simulink model "SIM_EXO_DAL_MN"  (R2021b)
(part 15 of 24)

t6933 = ct{2277};
t6934 = ct{2278};
t6994 = ct{2279};
t7 = ct{2280};
t7000 = ct{2281};
t7010 = ct{2282};
t7011 = ct{2283};
t7012 = ct{2284};
t7015 = ct{2285};
t7019 = ct{2286};
t7020 = ct{2287};
t7026 = ct{2288};
t7027 = ct{2289};
t7031 = ct{2290};
t7032 = ct{2291};
t7033 = ct{2292};
t7034 = ct{2293};
t7035 = ct{2294};
t7039 = ct{2295};
t7040 = ct{2296};
t7042 = ct{2297};
t7043 = ct{2298};
t7044 = ct{2299};
t7045 = ct{2300};
t7046 = ct{2301};
t7047 = ct{2302};
t7052 = ct{2303};
t7055 = ct{2304};
t7060 = ct{2305};
t7061 = ct{2306};
t7062 = ct{2307};
t7064 = ct{2308};
t7065 = ct{2309};
t7071 = ct{2310};
t7079 = ct{2311};
t7080 = ct{2312};
t7082 = ct{2313};
t7083 = ct{2314};
t7085 = ct{2315};
t7086 = ct{2316};
t7087 = ct{2317};
t7088 = ct{2318};
t7089 = ct{2319};
t7091 = ct{2320};
t7093 = ct{2321};
t7095 = ct{2322};
t7096 = ct{2323};
t7098 = ct{2324};
t71 = ct{2325};
t7100 = ct{2326};
t7104 = ct{2327};
t7108 = ct{2328};
t7109 = ct{2329};
t7110 = ct{2330};
t7113 = ct{2331};
t7115 = ct{2332};
t7119 = ct{2333};
t712 = ct{2334};
t7140 = ct{2335};
t7141 = ct{2336};
t7148 = ct{2337};
t7149 = ct{2338};
t7153 = ct{2339};
t7159 = ct{2340};
t7199 = ct{2341};
t72 = ct{2342};
t724 = ct{2343};
t7244 = ct{2344};
t7248 = ct{2345};
t7256 = ct{2346};
t7258 = ct{2347};
t7297 = ct{2348};
t73 = ct{2349};
t7306 = ct{2350};
t7334 = ct{2351};
t7335 = ct{2352};
t7364 = ct{2353};
t738 = ct{2354};
t739 = ct{2355};
t741 = ct{2356};
t742 = ct{2357};
t75 = ct{2358};
t7528 = ct{2359};
t753 = ct{2360};
t7549 = ct{2361};
t7550 = ct{2362};
t7551 = ct{2363};
t7553 = ct{2364};
t7557 = ct{2365};
t7558 = ct{2366};
t7560 = ct{2367};
t7564 = ct{2368};
t7565 = ct{2369};
t7567 = ct{2370};
t7568 = ct{2371};
t7569 = ct{2372};
t7570 = ct{2373};
t7571 = ct{2374};
t7573 = ct{2375};
t7574 = ct{2376};
t7575 = ct{2377};
t7576 = ct{2378};
t7577 = ct{2379};
t7578 = ct{2380};
t7579 = ct{2381};
t7580 = ct{2382};
t7581 = ct{2383};
t76 = ct{2384};
t760 = ct{2385};
t781 = ct{2386};
t792 = ct{2387};
t796 = ct{2388};
t797 = ct{2389};
t8 = ct{2390};
t803 = ct{2391};
t81 = ct{2392};
t824 = ct{2393};
t825 = ct{2394};
t826 = ct{2395};
t827 = ct{2396};
t830 = ct{2397};
t832 = ct{2398};
t84 = ct{2399};
t845 = ct{2400};
t847 = ct{2401};
t848 = ct{2402};
t852 = ct{2403};
t856 = ct{2404};
t86 = ct{2405};
t861 = ct{2406};
t866 = ct{2407};
t868 = ct{2408};
t869 = ct{2409};
t874 = ct{2410};
t875 = ct{2411};
t877 = ct{2412};
t878 = ct{2413};
t881 = ct{2414};
t893 = ct{2415};
t899 = ct{2416};
t9 = ct{2417};
t90 = ct{2418};
t902 = ct{2419};
t903 = ct{2420};
t905 = ct{2421};
t908 = ct{2422};
t909 = ct{2423};
t91 = ct{2424};
t910 = ct{2425};
t911 = ct{2426};
t912 = ct{2427};
t915 = ct{2428};
t917 = ct{2429};
t919 = ct{2430};
t922 = ct{2431};
t925 = ct{2432};
t926 = ct{2433};
t928 = ct{2434};
t929 = ct{2435};
t930 = ct{2436};
t931 = ct{2437};
t932 = ct{2438};
t934 = ct{2439};
t940 = ct{2440};
t944 = ct{2441};
t945 = ct{2442};
t947 = ct{2443};
t95 = ct{2444};
t952 = ct{2445};
t954 = ct{2446};
t955 = ct{2447};
t957 = ct{2448};
t958 = ct{2449};
t968 = ct{2450};
t970 = ct{2451};
t971 = ct{2452};
t972 = ct{2453};
t975 = ct{2454};
t976 = ct{2455};
t984 = ct{2456};
t985 = ct{2457};
t986 = ct{2458};
t989 = ct{2459};
t99 = ct{2460};
t991 = ct{2461};
t998 = ct{2462};
t6510 = t5822.*t6230.*(t29-t30).*(-5.517689141340903e-72);
t6527 = t5824.*t6222.*(t29-t30).*(-1.015171749786156e-71);
t6528 = t5824.*t6222.*(t29-t30).*(-5.520609140571798e-70);
t6529 = t5824.*t6222.*(t29-t30).*(-5.517689141340903e-72);
t6530 = t5824.*t6222.*(t29-t30).*1.015171749786156e-71;
t6531 = t5824.*t6222.*(t29-t30).*5.520609140571798e-70;
t6532 = t5824.*t6230.*(t29-t30).*(-1.015171749786156e-71);
t6533 = t5824.*t6230.*(t29-t30).*(-5.520609140571798e-70);
t6534 = t5824.*t6230.*(t29-t30).*(-5.517689141340903e-72);
t6535 = t5824.*t6230.*(t29-t30).*1.015171749786156e-71;
t6536 = t5824.*t6230.*(t29-t30).*5.520609140571798e-70;
t6550 = t5.*t5824.*t6230.*(t29-t30).*(-1.065477564130357e-78);
t6551 = t9.*t5824.*t6230.*(t29-t30).*(-1.065477564130357e-78);
t6552 = t9.*t5824.*t6230.*(t29-t30).*1.065477564130357e-78;
t6573 = t5824.*(t5879-t5.*(t7.*(t3719-t3788)+(t3.*t34.*t191.*(t29-t30))./8.112963841460668e+31)).*(t29-t30).*(-7.596454196607839e-68);
t6574 = (t5824.*(t5878+t9.*(t7.*(t3719-t3788)+(t3.*t34.*t191.*(t29-t30))./8.112963841460668e+31)).*(t29-t30))./1.316403645856965e+67;
t6580 = (t5779.*t6422)./2.0;
t6582 = t5824.*(t5879-t5.*(t7.*(t3719-t3788)+(t3.*t34.*t191.*(t29-t30))./8.112963841460668e+31)).*(t29-t30).*(-1.015171749786156e-71);
t6583 = t5824.*(t5879-t5.*(t7.*(t3719-t3788)+(t3.*t34.*t191.*(t29-t30))./8.112963841460668e+31)).*(t29-t30).*(-5.520609140571798e-70);
t6585 = t5824.*(t5878+t9.*(t7.*(t3719-t3788)+(t3.*t34.*t191.*(t29-t30))./8.112963841460668e+31)).*(t29-t30).*5.520609140571798e-70;
t6586 = t5824.*(t5878+t9.*(t7.*(t3719-t3788)+(t3.*t34.*t191.*(t29-t30))./8.112963841460668e+31)).*(t29-t30).*5.517689141340903e-72;
t6590 = t5824.*(t5879-t5.*(t7.*(t3719-t3788)+(t3.*t34.*t191.*(t29-t30))./8.112963841460668e+31)).*(t29-t30).*(-1.065477564130357e-78);
t6591 = t5824.*(t5878+t9.*(t7.*(t3719-t3788)+(t3.*t34.*t191.*(t29-t30))./8.112963841460668e+31)).*(t29-t30).*1.065477564130357e-78;
t6598 = t6103.*t6230.*2.0;
t6603 = t6103.*t6230.*2.67275158517898e-4;
t6604 = t6103.*t6230.*1.45270122047331e-4;
t6605 = t6103.*t6230.*8.40184101230148e-6;
t6607 = t6103.*t6230.*6.293113355513489e-13;
t6608 = t6103.*t6230.*8.252610559395431e-13;
t6634 = t6222.*t6230.*2.0;
t6638 = (t91.*t5824.*t6418)./1.316403645856965e+67;
t6649 = t6222.*t6230.*2.67275158517898e-4;
t6651 = t6222.*t6230.*1.45270122047331e-4;
t6653 = t6222.*t6230.*8.40184101230148e-6;
t6655 = t6222.*t6230.*6.293113355513489e-13;
t6657 = t6222.*t6230.*8.252610559395431e-13;
t6658 = t91.*t5824.*t6418.*5.520609140571798e-70;
t6659 = t91.*t5824.*t6418.*5.517689141340903e-72;
t6664 = t91.*t5824.*t6418.*1.065477564130357e-78;
t6696 = t6230.*(t5879-t5.*(t7.*(t3719-t3788)+(t3.*t34.*t191.*(t29-t30))./8.112963841460668e+31));
t6698 = -t6230.*(t5878+t9.*(t7.*(t3719-t3788)+(t3.*t34.*t191.*(t29-t30))./8.112963841460668e+31));
t6699 = t1498+t2507+t2772+t4837+t5024+t5145+t5301+t5638+t5639;
t6748 = t6230.*(t5878+t9.*(t7.*(t3719-t3788)+(t3.*t34.*t191.*(t29-t30))./8.112963841460668e+31)).*(-7.26350610236655e-5);
t6751 = t6230.*(t5878+t9.*(t7.*(t3719-t3788)+(t3.*t34.*t191.*(t29-t30))./8.112963841460668e+31)).*(-1.744166498897461e-6);
t6752 = t6230.*(t5878+t9.*(t7.*(t3719-t3788)+(t3.*t34.*t191.*(t29-t30))./8.112963841460668e+31)).*(-1.246862701090643e-6);
t6753 = t6230.*(t5878+t9.*(t7.*(t3719-t3788)+(t3.*t34.*t191.*(t29-t30))./8.112963841460668e+31)).*(-2.179051830709965e-7);
t6764 = t6230.*(t5878+t9.*(t7.*(t3719-t3788)+(t3.*t34.*t191.*(t29-t30))./8.112963841460668e+31)).*(-1.40259855e-11);
t6765 = t6230.*(t5878+t9.*(t7.*(t3719-t3788)+(t3.*t34.*t191.*(t29-t30))./8.112963841460668e+31)).*(-4.126305279697715e-13);
t6795 = t824+t1636+t1779+t3309+t3371+t3421+t3835+t3838+t4427+t5235+t5752;
t6828 = t6230.*(t6105-t9.*((t197.*(t29-t30))./9.007199254740992e+15+t3.*(t3219-t3230)));
t6829 = -t6230.*(t6106+t5.*((t197.*(t29-t30))./9.007199254740992e+15+t3.*(t3219-t3230)));
t6831 = t6230.*(t6106+t5.*((t197.*(t29-t30))./9.007199254740992e+15+t3.*(t3219-t3230)));
t6926 = t1488+t1567+t1628+t2570+t2805+t2889+t4927+t5017+t5093+t5144+t5423+t5650;
et8 = t5888+t5795.*(t2088-t4743).*8.081970098144003e-70;
et9 = t5683.*(t197.*(t29-t30).*9.007199254740992e+15+t3.*(t2444-t2449)).*8.081970098144003e-70;
t7013 = t4119.*(et8+et9).*(-1.0./2.0);
t7014 = t5771+t6353+t6354;
t7016 = -t7015;
et10 = t5889+t5795.*(t2088-t4743).*5.344156668414146e-72;
et11 = t5683.*(t197.*(t29-t30).*9.007199254740992e+15+t3.*(t2444-t2449)).*5.344156668414146e-72;
t7017 = t5658.*(et10+et11).*(-1.0./2.0);
et12 = t5892+t5795.*(t2088-t4743).*7.671525497590686e-73;
et13 = t5683.*(t197.*(t29-t30).*9.007199254740992e+15+t3.*(t2444-t2449)).*7.671525497590686e-73;
t7018 = t5662.*(et12+et13).*(-1.0./2.0);
et14 = t5883+t5795.*(t2088-t4743).*4.121912899099809e-68;
et15 = t5683.*(t197.*(t29-t30).*9.007199254740992e+15+t3.*(t2444-t2449)).*4.121912899099809e-68;
t7028 = t5939.*(et14+et15).*(-1.0./2.0);
et16 = t5882+t5795.*(t2088-t4743).*1.879526485671887e-68;
et17 = t5683.*(t197.*(t29-t30).*9.007199254740992e+15+t3.*(t2444-t2449)).*1.879526485671887e-68;
t7029 = t5940.*(et16+et17).*(-1.0./2.0);
t7030 = (t6422.*t6609)./2.0;
t7036 = -t7034;
t7041 = -t7039;
t7048 = -t7047;
t7051 = (t1429.*t7042)./2.0;
t7054 = (t1427.*t7045)./2.0;
t7056 = -t7055;
t7057 = (t6422.*t6874)./2.0;
t7067 = t1499+t1763+t2284+t2296+t2523+t2740+t2752+t3080+t3166+t4846+t5056+t5314+t5340+t5378+t5391+t5405+t5416+t5644+t5646;
t7069 = t1524+t1946+t2239+t2328+t2548+t2783+t2807+t3096+t3168+t4925+t5189+t5335+t5337+t5392+t5395+t5409+t5431+t5642+t5645;
t7078 = t1536+t1585+t1593+t1700+t1704+t2553+t2577+t2744+t2801+t2815+t2933+t4974+t5031+t5113+t5139+t5202+t5252+t5307+t5412+t5447+t5652+t5655;
t7084 = -t7083;
t7090 = -t7089;
t7092 = -t7091;
t7094 = -t7093;
t7097 = -t7096;
t7101 = -t7100;
t7111 = -t7110;
t7162 = t1533+t1663+t1760+t1809+t2358+t2362+t2435+t2452+t3565+t3572+t3617+t3640+t4047+t4050+t4069+t4083+t4186+t4211+t4683+t4714+t7042;
t7163 = t1683+t1807+t2036+t2081+t2359+t2364+t2439+t2454+t3676+t3717+t3781+t3818+t4053+t4056+t4070+t4086+t4256+t4333+t4684+t4717+t7045;
t7172 = t1605+t1849+t1896+t1961+t2079+t2100+t2176+t2208+t3648+t3752+t3754+t3833+t3892+t3904+t3915+t3940+t4315+t4368+t4371+t4460+t7062;
t5767 = -t5761;
t5785 = t5685./6.582018229284824e+63;
t5801 = t5685.*2.060956449549905e-68;
t5803 = t5685.*9.397632428359433e-69;
t5804 = t5685.*4.040985049072001e-70;
t5806 = t5685.*2.672078334207073e-72;
t5807 = t5685.*3.835762748795343e-73;
t5921 = (t1460.*t5840)./2.0;
t5924 = -t5922;
t5950 = (t3444.*t5840)./2.0;
t5987 = -t5985;
t5989 = -t5986;
t5993 = -t5992;
t6025 = -t6021;
t6040 = -t6033;
t6041 = -t6034;
t6044 = -t6037;
t6063 = -t6059;
t6080 = -t6074;
t6116 = t5657.*t5840;
t6141 = t6114.*7.26350610236655e-5;
t6144 = t6114.*1.744166498897461e-6;
t6146 = t6114.*1.246862701090643e-6;
t6147 = -t6142;
t6150 = -t6145;
t6155 = t6114.*2.179051830709965e-7;
t6172 = -t6170;
t6173 = t6114.*1.40259855e-11;
t6176 = -t6171;
t6177 = t6114.*4.126305279697715e-13;
t6216 = t5694+t5864;
t6217 = t5.*t6213;
t6218 = t9.*t6213;
t6219 = t5784.*t5840;
t6246 = -t6234;
t6252 = t5.*t6239;
t6253 = t9.*t6239;
t6256 = -t6254;
t6273 = t6214.*7.26735e-3;
t6275 = t6214.*7.26350610236655e-5;
t6290 = t6239.*1.33637579258949e-4;
t6294 = t6214.*1.40259855e-11;
t6296 = t6239.*7.26350610236655e-5;
t6297 = t47.*t6239;
t6300 = t6239.*4.20092050615074e-6;
t6304 = t58.*t6239;
t6305 = t75.*t6239;
t6306 = t76.*t6239;
t6307 = t84.*t6239;
t6310 = t71.*t6239;
t6321 = t6239.*3.146556677756745e-13;
t6323 = t6239.*4.126305279697715e-13;
t6324 = t142.*t6239;
t6327 = t151.*t6239;
t6334 = -t6332;
t6335 = -t6333;
t6339 = -t6336;
t6346 = -t6345;
t6358 = t5870+t5880;
t6370 = -t6368;
t6371 = -t6369;
t6394 = -t6392;
t6468 = t5874+t6233;
t6480 = (t91.*t5824.*t6213)./1.316403645856965e+67;
t6485 = -t6483;
t6498 = -t6496;
t6499 = t5.*t6497;
t6500 = t9.*t6497;
t6511 = t91.*t5824.*t6213.*1.015171749786156e-71;
t6512 = t91.*t5824.*t6213.*5.520609140571798e-70;
t6513 = t91.*t5824.*t6213.*5.517689141340903e-72;
t6537 = t9.*t6532;
t6538 = t5.*t6533;
t6539 = t9.*t6533;
t6540 = t9.*t6535;
t6541 = t9.*t6536;
t6542 = t5.*t6534;
t6570 = (t91.*t5824.*t6355)./1.316403645856965e+67;
t6571 = (t91.*t5824.*t6356)./1.316403645856965e+67;
t6575 = -t6574;
t6576 = t91.*t5824.*t6355.*1.015171749786156e-71;
t6577 = t91.*t5824.*t6355.*5.520609140571798e-70;
t6578 = t91.*t5824.*t6356.*5.520609140571798e-70;
t6579 = t91.*t5824.*t6356.*5.517689141340903e-72;
t6584 = t91.*t5824.*t6355.*1.065477564130357e-78;
t6587 = -t6585;
t6588 = t91.*t5824.*t6356.*1.065477564130357e-78;
t6592 = -t6591;
t6639 = (t91.*t5824.*t6419)./1.316403645856965e+67;
t6652 = -t6651;
t6654 = -t6653;
t6656 = -t6655;
t6660 = t91.*t5824.*t6419.*1.015171749786156e-71;
t6661 = t91.*t5824.*t6419.*5.520609140571798e-70;
t6667 = -t6664;
t6668 = t91.*t5824.*t6419.*1.065477564130357e-78;
t6688 = t5809+t6018+t6019;
t6737 = t6696.*1.33637579258949e-4;
t6743 = t6696.*4.00912737776847e-7;
t6744 = t6696.*1.246862701090643e-6;
t6745 = t6696.*3.383302988283333e-6;
t6756 = t6696.*3.146556677756745e-13;
t6757 = t6696.*1.40259855e-11;
t6810 = t5830+t6082+t6090;
t6813 = t5829+t6084+t6091;
t6816 = t5833+t6087+t6095;
t6819 = t5834+t6088+t6096;
t6820 = t5836+t6089+t6097;
t6830 = -t6828;
t6833 = t5843+t6117+t6122;
t6852 = t6828.*7.26350610236655e-5;
t6853 = t6831.*(-1.33637579258949e-4);
t6854 = t6828.*1.744166498897461e-6;
t6856 = t6828.*1.246862701090643e-6;
t6857 = t6831.*1.33637579258949e-4;
t6859 = t6828.*2.179051830709965e-7;
t6860 = t6831.*(-4.00912737776847e-7);
t6861 = t6831.*(-1.246862701090643e-6);
t6862 = t6831.*(-3.383302988283333e-6);
t6863 = t6831.*1.246862701090643e-6;
t6864 = t6828.*1.40259855e-11;
t6865 = t6828.*4.126305279697715e-13;
t6867 = t6831.*(-3.146556677756745e-13);
t6870 = t6831.*(-1.40259855e-11);
t6879 = t4119.*(t5831-t6095+t5679.*(t2088-t4743).*8.081970098144003e-70).*(-1.0./2.0);
t6880 = (t4119.*(t5831-t6095+t5679.*(t2088-t4743).*8.081970098144003e-70))./2.0;
t6886 = t5885+t6139+t6166;
t6887 = t5884+t6140+t6168;
t6899 = t5890+t6149+t6174;
t6905 = t5891+t6156+t6178;
t6912 = t5893+t6163+t6184;
t6927 = t1511+t1586+t1613+t2562+t2775+t2887+t4924+t4946+t5091+t5260+t5422+t5654;
t7006 = t5658.*(t5832-t6096+t5679.*(t2088-t4743).*5.344156668414146e-72).*(-1.0./2.0);
t7007 = (t5658.*(t5832-t6096+t5679.*(t2088-t4743).*5.344156668414146e-72))./2.0;
t7008 = t5662.*(t5835-t6097+t5679.*(t2088-t4743).*7.671525497590686e-73).*(-1.0./2.0);
t7009 = (t5662.*(t5835-t6097+t5679.*(t2088-t4743).*7.671525497590686e-73))./2.0;
t7022 = t5939.*(t5827-t6091+t5679.*(t2088-t4743).*4.121912899099809e-68).*(-1.0./2.0);
t7023 = t5940.*(t5828-t6090+t5679.*(t2088-t4743).*1.879526485671887e-68).*(-1.0./2.0);
t7024 = (t5939.*(t5827-t6091+t5679.*(t2088-t4743).*4.121912899099809e-68))./2.0;
t7025 = (t5940.*(t5828-t6090+t5679.*(t2088-t4743).*1.879526485671887e-68))./2.0;
t7068 = (t5.*t7067)./2.0;
t7070 = (t9.*t7069)./2.0;
t7177 = t2689+t2750+t3065+t3095+t3125+t3159+t4811+t4825+t4826+t4929+t5356+t5364+t5372+t5389+t5393+t5402+t7067;
t7178 = t2780+t2785+t3088+t3117+t3129+t3164+t4862+t4964+t5020+t5140+t5373+t5375+t5383+t5390+t5394+t5404+t7069;
t7214 = t2695+t2725+t2754+t2760+t2792+t2817+t2905+t2915+t4803+t4867+t4920+t4942+t4949+t4988+t4989+t5064+t5083+t5090+t5100+t5211+t7078;
t7544 = t753+t760+t797+t848+t852+t902+t908+t917+t928+t931+t944+t952+t975+t976+t991+t1090+t1122+t1147+t1156+t1194+t1292+t1441+t1816+t2028+t2223+t2486+t3416+t3417+t3426+t3429+t3432+t3436+t3464+t3465+t3469+t3489+t3498+t3501+t3504+t3510+t3521+t3530+t3535+t3540+t3554+t3571+t3574+t3577+t3578+t3605+t3607+t3637+t3659+t3666+t3694+t3726+t3863+t3960+t4004+t4008+t4011+t4015+t4134+t4423+t4592+t4597+t4780+t5228+t5316+t5323+t5354+t7030+t7044+t7048+t7113;
t5923 = -t5921;
t5953 = -t5950;
t6138 = t6116.*1.33637579258949e-4;
t6151 = -t6146;
t6152 = t6116.*3.383302988283333e-6;
t6158 = t6116.*4.00912737776847e-7;
t6159 = t6116.*1.246862701090643e-6;
t6162 = -t6155;
t6179 = t6116.*3.146556677756745e-13;
t6183 = t6116.*1.40259855e-11;
t6220 = t6216.^2;
t6223 = -t6218;
t6278 = t6219.*1.33637579258949e-4;
t6279 = t6219.*7.26735e-3;
t6298 = -t6294;
t6299 = -t6296;
t6301 = t6219.*1.40259855e-11;
t6311 = t6252.*(-7.26350610236655e-5);
t6312 = t6252.*(-1.246862701090643e-6);
t6316 = t6252.*(-1.744166498897461e-6);
t6322 = -t6321;
t6325 = t6252.*1.40259855e-11;
t6326 = t6253.*1.40259855e-11;
t6359 = t5515+t5783+t5785;
t6399 = t5619+t5799+t5803;
t6400 = t5617+t5798+t5801;
t6401 = t5623+t5800+t5804;
t6402 = t5626+t5802+t5806;
t6405 = t5628+t5805+t5807;
t6412 = (t91.*t4838.*t6216)./1.316403645856965e+67;
t6423 = t91.*t4838.*t6216.*1.015171749786156e-71;
t6424 = t91.*t4838.*t6216.*5.520609140571798e-70;
t6425 = t91.*t4838.*t6216.*5.517689141340903e-72;
t6426 = t91.*t4838.*t6216.*1.656182742171539e-72;
t6438 = (t91.*t5684.*t6216)./1.316403645856965e+67;
t6447 = t91.*t5684.*t6216.*1.015171749786156e-71;
t6448 = t91.*t5684.*t6216.*5.520609140571798e-70;
t6449 = t91.*t5684.*t6216.*5.517689141340903e-72;
t6464 = t4.*t6216.*(t3136-t5691).*-2.0;
t6465 = t5863+t6217;
t6470 = t5873+t6246;
t6472 = t4.*t6216.*(t3136-t5691).*(-2.67275158517898e-4);
t6473 = (t91.*t5822.*t6216)./1.316403645856965e+67;
t6474 = t4.*t6216.*(t3136-t5691).*(-1.45270122047331e-4);
t6475 = t4.*t6216.*(t3136-t5691).*1.45270122047331e-4;
t6476 = t4.*t6216.*(t3136-t5691).*(-8.40184101230148e-6);
t6479 = t4.*t6216.*(t3136-t5691).*(-6.293113355513489e-13);
t6482 = t4.*t6216.*(t3136-t5691).*6.293113355513489e-13;
t6484 = -t6480;
t6486 = (t91.*t5824.*t6216)./1.316403645856965e+67;
t6488 = t4.*t6216.*(t3136-t5691).*(-8.252610559395431e-13);
t6493 = t9.*t91.*t5824.*t6216.*(-7.596454196607839e-68);
t6503 = t91.*t5822.*t6216.*5.520609140571798e-70;
t6504 = t91.*t5822.*t6216.*1.015171749786156e-71;
t6505 = t91.*t5822.*t6216.*5.517689141340903e-72;
t6514 = -t6511;
t6515 = -t6512;
t6516 = t91.*t5824.*t6216.*1.015171749786156e-71;
t6517 = t91.*t5824.*t6216.*5.520609140571798e-70;
t6518 = t91.*t5824.*t6216.*5.517689141340903e-72;
t6524 = t9.*t91.*t5824.*t6216.*(-1.015171749786156e-71);
t6525 = t9.*t91.*t5824.*t6216.*(-5.520609140571798e-70);
t6543 = t5.*t91.*t5824.*t6216.*1.065477564130357e-78;
t6544 = t9.*t91.*t5824.*t6216.*1.065477564130357e-78;
t6572 = -t6571;
t6581 = -t6578;
t6589 = -t6588;
t6596 = t6216.*(t5670+t4.*(t1458-t5665)).*-2.0;
t6599 = t6216.*(t5670+t4.*(t1458-t5665)).*(-2.67275158517898e-4);
t6600 = t6216.*(t5670+t4.*(t1458-t5665)).*(-1.45270122047331e-4);
t6601 = t6216.*(t5670+t4.*(t1458-t5665)).*(-8.40184101230148e-6);
t6602 = t6216.*(t5670+t4.*(t1458-t5665)).*(-6.293113355513489e-13);
t6606 = t6216.*(t5670+t4.*(t1458-t5665)).*(-8.252610559395431e-13);
t6611 = t91.*t4838.*(t6218+t5.*(t3136-t5691)).*(-7.596454196607839e-68);
t6612 = (t91.*t4838.*(t6218+t5.*(t3136-t5691)))./1.316403645856965e+67;
t6613 = t4838.*t6468.*(t29-t30).*(-7.596454196607839e-68);
t6618 = t91.*t4838.*(t6218+t5.*(t3136-t5691)).*(-1.015171749786156e-71);
t6619 = t91.*t4838.*(t6218+t5.*(t3136-t5691)).*(-5.520609140571798e-70);
t6621 = t91.*t4838.*(t6218+t5.*(t3136-t5691)).*1.015171749786156e-71;
t6622 = t91.*t4838.*(t6218+t5.*(t3136-t5691)).*5.520609140571798e-70;
t6623 = t6213.*t6216.*2.0;
t6625 = t4838.*t6468.*(t29-t30).*(-5.520609140571798e-70);
t6626 = t91.*t4838.*(t6218+t5.*(t3136-t5691)).*(-1.065477564130357e-78);
t6627 = t4838.*t6468.*(t29-t30).*(-5.517689141340903e-72);
t6630 = t91.*t4838.*(t6218+t5.*(t3136-t5691)).*1.065477564130357e-78;
t6631 = t4838.*t6468.*(t29-t30).*5.517689141340903e-72;
t6635 = t4838.*t6468.*(t29-t30).*(-1.065477564130357e-78);
t6642 = t6213.*t6216.*2.67275158517898e-4;
t6643 = t6213.*t6216.*1.45270122047331e-4;
t6645 = t6213.*t6216.*8.40184101230148e-6;
t6647 = t6213.*t6216.*6.293113355513489e-13;
t6650 = t6213.*t6216.*8.252610559395431e-13;
t6673 = t91.*t5684.*(t6218+t5.*(t3136-t5691)).*(-7.596454196607839e-68);
t6674 = t5684.*t6468.*(t29-t30).*(-7.596454196607839e-68);
t6678 = t91.*t5684.*(t6218+t5.*(t3136-t5691)).*(-1.015171749786156e-71);
t6679 = t91.*t5684.*(t6218+t5.*(t3136-t5691)).*(-5.520609140571798e-70);
t6681 = t5684.*t6468.*(t29-t30).*(-5.520609140571798e-70);
t6682 = t91.*t5684.*(t6218+t5.*(t3136-t5691)).*(-1.065477564130357e-78);
t6683 = t5684.*t6468.*(t29-t30).*(-5.517689141340903e-72);
t6686 = t5684.*t6468.*(t29-t30).*(-1.065477564130357e-78);
t6692 = t6216.*t6355;
t6693 = t4.*(t6218+t5.*(t3136-t5691)).*(t3136-t5691);
t6694 = t6216.*t6356;
t6695 = t4.*t5861.*t6468;
t6705 = t91.*t5822.*(t6218+t5.*(t3136-t5691)).*(-7.596454196607839e-68);
t6707 = t44.*(t6218+t5.*(t3136-t5691)).*(t3136-t5691);
t6708 = (t91.*t5822.*(t6218+t5.*(t3136-t5691)))./1.316403645856965e+67;
t6722 = t5822.*t6468.*(t29-t30).*(-7.596454196607839e-68);
t6725 = (t5822.*t6468.*(t29-t30))./1.316403645856965e+67;
t6727 = t139.*(t6218+t5.*(t3136-t5691)).*(t3136-t5691);
t6736 = t91.*t5824.*(t6218+t5.*(t3136-t5691)).*(-7.596454196607839e-68);
t6754 = t5824.*t6468.*(t29-t30).*(-7.596454196607839e-68);
t6759 = -t6756;
t6769 = t91.*t5822.*(t6218+t5.*(t3136-t5691)).*(-1.015171749786156e-71);
t6770 = t91.*t5822.*(t6218+t5.*(t3136-t5691)).*(-5.520609140571798e-70);
t6772 = t91.*t5822.*(t6218+t5.*(t3136-t5691)).*1.015171749786156e-71;
t6773 = t91.*t5822.*(t6218+t5.*(t3136-t5691)).*5.520609140571798e-70;
t6775 = t5822.*t6468.*(t29-t30).*(-5.520609140571798e-70);
t6777 = t5822.*t6468.*(t29-t30).*5.520609140571798e-70;
t6778 = t91.*t5822.*(t6218+t5.*(t3136-t5691)).*(-1.065477564130357e-78);
t6780 = t5822.*t6468.*(t29-t30).*(-5.517689141340903e-72);
t6785 = t91.*t5822.*(t6218+t5.*(t3136-t5691)).*1.065477564130357e-78;
t6787 = t5822.*t6468.*(t29-t30).*5.517689141340903e-72;
t6791 = t91.*t5824.*(t6218+t5.*(t3136-t5691)).*(-1.015171749786156e-71);
t6792 = t91.*t5824.*(t6218+t5.*(t3136-t5691)).*(-5.520609140571798e-70);
t6793 = t91.*t5824.*(t6218+t5.*(t3136-t5691)).*(-5.517689141340903e-72);
t6794 = t91.*t5824.*(t6218+t5.*(t3136-t5691)).*5.520609140571798e-70;
t6796 = t5822.*t6468.*(t29-t30).*(-1.065477564130357e-78);
t6800 = t5824.*t6468.*(t29-t30).*(-1.015171749786156e-71);
t6801 = t5824.*t6468.*(t29-t30).*(-5.520609140571798e-70);
t6802 = t91.*t5824.*(t6218+t5.*(t3136-t5691)).*(-1.065477564130357e-78);
t6803 = t5824.*t6468.*(t29-t30).*(-5.517689141340903e-72);
t6805 = t5824.*t6468.*(t29-t30).*1.015171749786156e-71;
t6806 = t5824.*t6468.*(t29-t30).*5.520609140571798e-70;
t6807 = t91.*t5824.*(t6218+t5.*(t3136-t5691)).*1.065477564130357e-78;
t6814 = t5824.*t6468.*(t29-t30).*(-1.065477564130357e-78);
t6815 = t5824.*t6468.*(t29-t30).*1.065477564130357e-78;
t6822 = t6216.*t6418;
t6823 = t6216.*t6419;
t6855 = -t6852;
t6858 = -t6854;
t6866 = -t6864;
t6869 = -t6865;
t6876 = (t5670+t4.*(t1458-t5665)).*(t6218+t5.*(t3136-t5691));
t6877 = t6103.*t6468;
t6929 = -t6213.*(t6218+t5.*(t3136-t5691));
t6932 = -t6216.*(t6218+t5.*(t3136-t5691));
t6935 = t6222.*t6468;
t6937 = t6230.*t6468;
t6943 = t6213.*(t6218+t5.*(t3136-t5691)).*(-1.33637579258949e-4);
t6949 = t6216.*(t6218+t5.*(t3136-t5691)).*(-1.33637579258949e-4);
t6951 = t6213.*(t6218+t5.*(t3136-t5691)).*(-1.246862701090643e-6);
t6953 = t6213.*(t6218+t5.*(t3136-t5691)).*(-3.383302988283333e-6);
t6955 = t6216.*(t6218+t5.*(t3136-t5691)).*(-7.26350610236655e-5);
t6958 = t6216.*(t6218+t5.*(t3136-t5691)).*(-1.744166498897461e-6);
t6959 = t6216.*(t6218+t5.*(t3136-t5691)).*(-1.246862701090643e-6);
t6960 = t6216.*(t6218+t5.*(t3136-t5691)).*(-3.383302988283333e-6);
t6963 = t6213.*(t6218+t5.*(t3136-t5691)).*(-3.146556677756745e-13);
t6966 = t6213.*(t6218+t5.*(t3136-t5691)).*(-1.40259855e-11);
t6969 = t6216.*(t6218+t5.*(t3136-t5691)).*(-3.146556677756745e-13);
t6970 = t6216.*(t6218+t5.*(t3136-t5691)).*(-1.40259855e-11);
t6971 = t6216.*(t6218+t5.*(t3136-t5691)).*3.146556677756745e-13;
t6972 = t6216.*(t6218+t5.*(t3136-t5691)).*(-4.126305279697715e-13);
t6160 = -t6152;
t6164 = -t6158;
t6185 = -t6179;
t6188 = -t6183;
t6226 = t5.*t6220;
t6227 = t9.*t6220;
t6281 = t6220.*1.33637579258949e-4;
t6282 = t6220.*7.26350610236655e-5;
t6283 = t47.*t6220;
t6285 = t6220.*4.20092050615074e-6;
t6286 = t58.*t6220;
t6287 = t75.*t6220;
t6288 = t76.*t6220;
t6289 = t84.*t6220;
t6291 = t71.*t6220;
t6302 = t6220.*3.146556677756745e-13;
t6308 = t6220.*4.126305279697715e-13;
t6309 = t142.*t6220;
t6317 = t151.*t6220;
t6328 = -t6325;
t6413 = -t6412;
t6442 = (t4126.*t6401)./2.0;
t6443 = (t4149.*t6401)./2.0;
t6445 = (t4161.*t6402)./2.0;
t6450 = -t6449;
t6451 = (t4154.*t6405)./2.0;
t6466 = t5862+t6223;
t6477 = (t5620.*t6402)./2.0;
t6489 = (t5616.*t6405)./2.0;
t6490 = t5.*t6486;
t6491 = t9.*t6486;
t6519 = -t6516;
t6520 = -t6517;
t6521 = t9.*t6516;
t6522 = t5.*t6517;
t6523 = t9.*t6517;
t6526 = t5.*t6518;
t6545 = -t6544;
t6563 = (t5787.*t6399)./2.0;
t6564 = (t5786.*t6400)./2.0;
t6593 = (t5850.*t6399)./2.0;
t6594 = (t5851.*t6400)./2.0;
t6610 = (t91.*t4838.*t6465)./1.316403645856965e+67;
t6614 = t4838.*t6470.*(t29-t30).*(-7.596454196607839e-68);
t6615 = (t4838.*t6470.*(t29-t30))./1.316403645856965e+67;
t6616 = t91.*t4838.*t6465.*5.520609140571798e-70;
t6617 = t91.*t4838.*t6465.*5.517689141340903e-72;
t6624 = t91.*t4838.*t6465.*1.065477564130357e-78;
t6628 = t4838.*t6470.*(t29-t30).*(-1.015171749786156e-71);
t6629 = t4838.*t6470.*(t29-t30).*(-5.520609140571798e-70);
t6632 = t4838.*t6470.*(t29-t30).*1.015171749786156e-71;
t6633 = t4838.*t6470.*(t29-t30).*5.520609140571798e-70;
t6636 = t4838.*t6470.*(t29-t30).*(-1.065477564130357e-78);
t6637 = t4838.*t6470.*(t29-t30).*1.065477564130357e-78;
t6644 = -t6643;
t6646 = -t6645;
t6648 = -t6647;
t6672 = (t91.*t5684.*t6465)./1.316403645856965e+67;
t6675 = t5684.*t6470.*(t29-t30).*(-7.596454196607839e-68);
t6676 = t91.*t5684.*t6465.*5.520609140571798e-70;
t6677 = t91.*t5684.*t6465.*5.517689141340903e-72;
t6680 = t91.*t5684.*t6465.*1.065477564130357e-78;
t6684 = t5684.*t6470.*(t29-t30).*(-1.015171749786156e-71);
t6685 = t5684.*t6470.*(t29-t30).*(-5.520609140571798e-70);
t6687 = t5684.*t6470.*(t29-t30).*(-1.065477564130357e-78);
t6691 = -t4.*t6465.*(t3136-t5691);
t6697 = t4.*t5861.*t6470;
t6701 = (t91.*t5822.*t6465)./1.316403645856965e+67;
t6704 = t6692.*1.33637579258949e-4;
t6706 = -t57.*t6465.*(t3136-t5691);
t6709 = t4.*t6465.*(t3136-t5691).*(-1.744166498897461e-6);
t6710 = t4.*t6465.*(t3136-t5691).*(-1.246862701090643e-6);
t6711 = t6692.*4.00912737776847e-7;
t6712 = t6692.*1.246862701090643e-6;
t6713 = t6692.*3.383302988283333e-6;
t6714 = t4.*t6465.*(t3136-t5691).*(-2.179051830709965e-7);
t6715 = t6693.*4.00912737776847e-7;
t6716 = t6694.*7.26350610236655e-5;
t6717 = t6693.*1.246862701090643e-6;
t6718 = t6693.*3.383302988283333e-6;
t6719 = t6694.*1.744166498897461e-6;
t6720 = t6694.*1.246862701090643e-6;
t6721 = t6694.*2.179051830709965e-7;
t6723 = t4.*t6465.*(t3136-t5691).*(-1.40259855e-11);
t6724 = t6692.*3.146556677756745e-13;
t6726 = t6692.*1.40259855e-11;
t6729 = (t91.*t5824.*t6465)./1.316403645856965e+67;
t6730 = -t150.*t6465.*(t3136-t5691);
t6731 = t5822.*t6470.*(t29-t30).*(-7.596454196607839e-68);
t6732 = t6693.*1.40259855e-11;
t6733 = t6693.*(-3.146556677756745e-13);
t6734 = (t5822.*t6470.*(t29-t30))./1.316403645856965e+67;
t6735 = t6694.*1.40259855e-11;
t6738 = t6694.*4.126305279697715e-13;
t6739 = t6695.*7.26350610236655e-5;
t6740 = t44.*t5861.*t6470;
t6741 = t6695.*1.744166498897461e-6;
t6742 = t6695.*1.246862701090643e-6;
t6746 = t6695.*2.179051830709965e-7;
t6755 = t6695.*1.40259855e-11;
C_dq = ft_14({dq1,dq2,dq3,dq4,dq5,dq6,t1004,t1016,t1019,t1020,t1031,t1039,t1046,t1050,t1056,t1061,t1069,t1075,t1076,t1077,t1081,t1083,t1088,t1090,t1095,t1099,t1101,t1106,t1108,t112,t1122,t113,t1133,t1144,t1146,t1147,t115,t1150,t1152,t1155,t1156,t1158,t116,t1165,t1170,t1171,t1174,t1177,t1179,t1184,t1185,t1191,t1193,t1194,t1196,t1201,t1203,t1205,t1207,t121,t1211,t1212,t1213,t1215,t1221,t1224,t1225,t1227,t1228,t1233,t1245,t125,t1250,t1253,t1254,t1258,t1273,t1274,t1282,t1285,t1288,t1292,t1300,t1301,t1306,t131,t1316,t132,t1322,t1323,t1324,t133,t1330,t1331,t1333,t1337,t1342,t1344,t1345,t1348,t1353,t1365,t1377,t1379,t1380,t1383,t1388,t139,t1391,t1402,t1407,t1409,t1411,t1413,t1419,t1423,t1426,t1427,t1428,t1429,t1436,t144,t1440,t1441,t1443,t1445,t1446,t1449,t1454,t1457,t1458,t1460,t1471,t148,t1486,t1487,t1489,t1493,t1494,t1495,t1496,t15,t150,t1503,t1508,t1517,t1520,t1523,t1526,t1530,t1531,t1534,t1537,t1538,t1540,t1541,t1542,t1548,t1550,t1551,t156,t1568,t1570,t1574,t1577,t1578,t158,t1581,t1582,t1584,t1587,t1590,t1592,t1593,t1594,t1598,t16,t1600,t1601,t1602,t1606,t1607,t1609,t1612,t1614,t1615,t1616,t1617,t1619,t1620,t1621,t1622,t1625,t1627,t1630,t1642,t1647,t1648,t1651,t1655,t1656,t1659,t166,t1660,t1661,t1667,t1670,t1672,t1674,t1681,t1687,t1692,t1697,t1699,t17,t1701,t1704,t1705,t1706,t1707,t1708,t171,t1710,t1715,t1716,t1718,t1719,t1721,t1724,t1731,t1732,t1734,t1735,t1736,t1740,t1745,t1747,t1748,t1753,t1754,t1756,t1758,t1759,t1761,t1762,t1766,t1767,t1769,t1770,t1771,t1772,t1775,t1776,t1777,t1781,t1783,t1784,t1792,t1793,t1794,t1795,t1797,t1798,t18,t1800,t1805,t1806,t1808,t1811,t1812,t1814,t1815,t1816,t1820,t1821,t1823,t1827,t1828,t1829,t183,t1831,t1833,t1834,t1835,t1836,t1839,t1847,t185,t1855,t1856,t1858,t1860,t1861,t1863,t1868,t1870,t1873,t1878,t1882,t1884,t1886,t1892,t1899,t19,t190,t1900,t1902,t1906,t1908,t1909,t191,t1913,t1916,t1917,t1922,t1925,t1930,t1937,t1938,t1941,t1942,t1947,t1951,t1952,t196,t1967,t1968,t1969,t197,t1974,t1977,t1981,t1983,t1984,t1985,t1986,t1989,t199,t1992,t1993,t1995,t1997,t1998,t1999,t2,t20,t200,t2002,t2003,t2004,t2006,t2008,t201,t2014,t2015,t2017,t202,t2026,t2027,t2028,t2034,t2035,t2038,t2039,t2043,t2047,t2050,t2052,t2053,t206,t2060,t2062,t2066,t2068,t2069,t207,t2070,t2075,t2076,t2077,t2083,t2085,t2088,t2091,t2096,t2098,t21,t2106,t2110,t2113,t2115,t2116,t2118,t2119,t2121,t2123,t2128,t2130,t2132,t2133,t2134,t2136,t2142,t2143,t2145,t2149,t2150,t2154,t2158,t2164,t2165,t2177,t2178,t2180,t2181,t2184,t2186,t2187,t2189,t2191,t2192,t2193,t2196,t2197,t2199,t22,t2200,t2202,t2203,t2211,t2213,t2214,t2217,t2220,t2224,t2234,t2236,t224,t2243,t225,t2253,t2256,t2257,t2266,t2267,t227,t228,t2289,t2291,t2298,t2299,t23,t230,t2300,t2303,t2304,t231,t2312,t2314,t2315,t2320,t2326,t233,t2330,t2333,t2334,t2338,t234,t2341,t2342,t235,t236,t2383,t2390,t2392,t2395,t2396,t2397,t2398,t24,t240,t2416,t2420,t2421,t2424,t243,t244,t2443,t2444,t2449,t2465,t2466,t2474,t2481,t2483,t2486,t249,t2490,t2494,t2497,t2502,t2524,t2525,t2530,t2539,t2544,t2546,t2549,t2552,t2554,t2555,t2556,t2560,t2563,t2564,t2565,t2566,t2567,t2568,t2569,t257,t2571,t2574,t2575,t2576,t2578,t2579,t258,t2588,t2589,t2597,t2598,t2599,t2611,t2612,t2615,t2617,t2627,t263,t2640,t2641,t2655,t2656,t266,t2666,t2684,t2686,t2692,t2694,t270,t2706,t2720,t2722,t2724,t2726,t273,t2737,t274,t2741,t2743,t2748,t2749,t275,t2753,t2755,t2757,t2759,t276,t2761,t2764,t277,t2771,t2778,t278,t2791,t2793,t2795,t2797,t2798,t2799,t280,t2800,t2802,t2806,t2812,t2816,t2818,t2824,t2825,t2827,t2833,t2835,t284,t2851,t2857,t2861,t2868,t287,t2872,t2877,t2880,t2881,t2893,t2895,t2896,t29,t290,t2906,t291,t2911,t2913,t2916,t2918,t292,t2921,t2922,t2932,t294,t2941,t2944,t2956,t2958,t2965,t297,t2973,t2977,t2987,t299,t2999,t3,t30,t300,t302,t303,t304,t3047,t305,t306,t3083,t309,t310,t311,t313,t3136,t314,t3142,t315,t316,t318,t319,t320,t3200,t3209,t3213,t3219,t322,t3222,t3224,t3230,t3239,t324,t3247,t325,t3266,t3268,t3274,t328,t3321,t333,t3338,t336,t3365,t3368,t3369,t337,t3375,t3378,t3380,t3383,t3387,t3390,t3391,t3392,t3397,t34,t340,t3400,t3405,t3407,t3409,t3416,t3417,t3418,t3420,t3422,t3426,t3429,t3430,t3432,t3434,t3435,t3436,t3437,t3439,t344,t3440,t3441,t3443,t3444,t3445,t3446,t3449,t3450,t3453,t3457,t3458,t346,t3462,t3463,t3464,t3465,t3468,t3469,t347,t3471,t3472,t3474,t3475,t3476,t3479,t348,t3480,t3483,t3485,t3489,t349,t3490,t3491,t3492,t3493,t3496,t3498,t3499,t350,t3500,t3501,t3504,t3506,t3507,t3510,t3511,t3513,t3514,t3515,t3517,t3518,t352,t3521,t3522,t3523,t3526,t353,t3530,t3531,t3532,t3535,t3536,t3539,t3540,t3542,t3543,t3547,t3554,t3556,t3557,t356,t3562,t3568,t3569,t357,t3571,t3574,t3577,t3578,t358,t3582,t3583,t3584,t3585,t359,t3592,t3593,t3605,t3606,t3607,t361,t3610,t3611,t3612,t3618,t362,t3634,t3635,t3637,t3642,t3644,t365,t3656,t3658,t3659,t3662,t3666,t3667,t3668,t3672,t3673,t3678,t368,t3682,t369,t3694,t3702,t3706,t3708,t371,t3719,t372,t3725,t3726,t373,t3732,t3733,t3734,t3738,t374,t3743,t3746,t3753,t3755,t3757,t3759,t3761,t3763,t3764,t3765,t3767,t377,t3772,t378,t3783,t3785,t3788,t379,t3792,t380,t3819,t382,t3821,t3822,t3823,t3824,t3831,t384,t3843,t3845,t3851,t3852,t3853,t386,t3863,t3869,t387,t3871,t3873,t3874,t3875,t3876,t388,t3882,t3884,t3889,t3890,t3891,t3907,t391,t3910,t3913,t392,t3921,t3922,t3923,t3944,t395,t3951,t3954,t3956,t3957,t3959,t396,t3960,t3968,t3969,t3971,t3972,t3976,t3978,t3979,t3992,t3993,t3995,t3997,t4,t400,t4000,t4004,t401,t4010,t4011,t4014,t4015,t402,t403,t406,t4089,t4099,t410,t4100,t4103,t4108,t411,t4113,t4115,t4118,t4119,t412,t4121,t4123,t4126,t413,t4132,t4134,t4138,t414,t4143,t4146,t4148,t415,t4152,t4153,t4158,t416,t4166,t417,t4173,t4178,t4179,t418,t4181,t4183,t4185,t4190,t4196,t4197,t420,t4206,t4208,t4210,t4217,t422,t4221,t4223,t4226,t4228,t423,t4230,t4232,t4234,t424,t4243,t4249,t425,t4250,t4251,t4254,t4255,t4259,t4261,t4263,t427,t4274,t4276,t4278,t4279,t428,t4285,t4286,t429,t4293,t4298,t4301,t4304,t4305,t4306,t431,t4317,t4318,t432,t4327,t4329,t433,t4332,t4335,t4337,t4339,t434,t4342,t4344,t4345,t4347,t4348,t4349,t435,t4350,t436,t4369,t437,t4370,t4378,t438,t4380,t4382,t4385,t4388,t439,t4392,t4394,t4395,t4396,t4397,t440,t4402,t4403,t4405,t4406,t4407,t441,t4410,t4412,t4413,t4414,t4416,t4417,t4418,t4419,t442,t4420,t4423,t4425,t4426,t4428,t4429,t4431,t4436,t4437,t444,t4440,t4444,t4446,t4447,t4449,t445,t4450,t4453,t4462,t4467,t4468,t4469,t4471,t4473,t4475,t4478,t4479,t448,t4482,t4483,t4485,t4486,t4487,t4488,t4489,t449,t4490,t4494,t4495,t4498,t4499,t45,t450,t4500,t4501,t4502,t4505,t4506,t4509,t4510,t4515,t4518,t4519,t452,t4520,t4521,t4522,t4523,t4526,t4527,t4528,t453,t4530,t4534,t4536,t4538,t454,t4541,t4543,t4545,t4546,t4549,t4551,t4552,t4553,t4556,t4557,t4558,t4559,t4565,t4568,t457,t4570,t4572,t4575,t4577,t4578,t458,t4581,t4582,t4586,t4587,t4588,t4589,t459,t4590,t4591,t4592,t4593,t4595,t4596,t4598,t460,t4600,t4601,t4602,t4604,t4605,t4606,t4607,t4608,t461,t4614,t4616,t4619,t462,t4621,t4622,t4623,t4624,t4625,t4626,t4629,t463,t4633,t4634,t4636,t464,t4644,t4645,t4647,t4648,t465,t4654,t4656,t4659,t466,t4660,t4666,t4667,t4669,t4673,t4674,t4675,t4678,t468,t4682,t469,t4694,t4695,t4696,t4697,t470,t4707,t4708,t471,t472,t4724,t4727,t4728,t4731,t4732,t4733,t4737,t4738,t4739,t4742,t4743,t4745,t4747,t4748,t475,t4755,t4756,t4762,t4763,t477,t4773,t4775,t4780,t4781,t4782,t4783,t4785,t4786,t479,t480,t481,t4810,t482,t4824,t483,t4838,t4842,t485,t486,t4864,t4866,t4869,t4870,t488,t4884,t489,t4903,t4904,t491,t4911,t4914,t4919,t492,t493,t4934,t4936,t494,t4950,t4953,t4957,t496,t497,t4973,t498,t4981,t4983,t4984,t4987,t499,t4990,t4993,t4994,t4995,t4996,t5,t50,t500,t5000,t5002,t5007,t5008,t5009,t501,t502,t5021,t5022,t5023,t5026,t5027,t503,t5032,t5039,t504,t505,t5058,t506,t5061,t5063,t5065,t507,t5075,t5076,t508,t5080,t5084,t5086,t5087,t509,t5097,t5099,t510,t5102,t5107,t511,t5112,t5114,t512,t5121,t5123,t513,t5132,t5136,t514,t5147,t5150,t5151,t516,t5164,t5166,t517,t518,t5184,t5195,t520,t5203,t5204,t5206,t521,t5210,t5215,t5217,t5219,t522,t5227,t5228,t523,t5232,t5233,t5236,t5238,t524,t5242,t5244,t5249,t525,t5251,t5255,t5258,t5259,t526,t5262,t5269,t527,t5275,t5279,t528,t5280,t5285,t529,t5297,t53,t530,t531,t5316,t5318,t532,t5320,t5323,t5324,t533,t5333,t5339,t534,t5344,t535,t5354,t536,t537,t5370,t538,t539,t540,t543,t544,t5443,t545,t5450,t5457,t5459,t546,t5464,t5465,t5466,t547,t548,t5480,t5482,t5483,t5484,t5486,t5487,t5488,t549,t5507,t551,t552,t5521,t553,t554,t555,t556,t557,t558,t559,t560,t5602,t5605,t561,t562,t5621,t5622,t563,t5633,t5634,t5636,t564,t5647,t5648,t5657,t5658,t5662,t5665,t5666,t567,t5670,t5676,t5677,t5679,t568,t5683,t5684,t5688,t569,t5691,t5699,t57,t570,t5700,t5702,t5704,t5706,t5708,t5709,t571,t5710,t5717,t5718,t572,t5729,t573,t5730,t5735,t5738,t5739,t574,t5740,t5742,t5744,t5750,t5755,t5756,t5757,t576,t5762,t5766,t5767,t5769,t5770,t5772,t5774,t5775,t5776,t5778,t578,t5784,t5786,t5787,t5790,t5791,t5792,t5794,t5795,t5797,t580,t5808,t581,t5810,t582,t5822,t5823,t5824,t5825,t5826,t5831,t5838,t5839,t584,t5840,t5841,t5842,t5844,t5845,t5846,t5847,t5848,t5849,t5850,t5851,t5852,t5859,t586,t5861,t587,t5872,t5878,t5881,t5882,t5883,t5888,t5889,t589,t5892,t5894,t5895,t5897,t5898,t5899,t590,t5900,t5901,t5904,t5905,t5907,t5909,t591,t5911,t5912,t5914,t5915,t5916,t5917,t5918,t5919,t592,t5920,t5921,t5922,t5923,t5924,t5925,t5926,t5928,t5929,t593,t5930,t5931,t5932,t5933,t5934,t5935,t5936,t5937,t5938,t5939,t594,t5940,t5941,t5942,t5943,t5944,t5945,t5946,t5947,t5948,t5949,t595,t5950,t5951,t5952,t5953,t5954,t5956,t5957,t5958,t5959,t596,t5960,t5961,t5962,t5964,t5965,t5966,t5967,t5968,t597,t5970,t5971,t5972,t5973,t5974,t5975,t5976,t5977,t5978,t5979,t5980,t5981,t5982,t5983,t5984,t5985,t5986,t5987,t5988,t5989,t5991,t5993,t5994,t5995,t5996,t5997,t5998,t5999,t6,t60,t600,t6000,t6001,t6002,t6003,t6004,t6005,t6007,t6008,t6009,t6010,t6011,t6012,t6013,t6014,t6016,t6017,t6019,t602,t6020,t6024,t6025,t6026,t6028,t6029,t603,t6030,t6032,t6035,t6037,t6038,t604,t6040,t6041,t6042,t6043,t6044,t6045,t6046,t6047,t6048,t6049,t605,t6051,t6052,t6053,t6054,t6055,t6056,t6057,t6060,t6061,t6062,t6063,t6064,t6065,t6067,t6068,t6069,t6073,t6074,t6075,t6076,t6077,t6078,t6079,t6080,t6081,t6083,t6085,t6086,t609,t6093,t6094,t6095,t610,t6103,t6108,t6109,t611,t6110,t6111,t6113,t6114,t6116,t6118,t6119,t612,t6120,t6121,t6123,t6125,t6126,t6127,t6128,t6129,t613,t6130,t6131,t6132,t6134,t6135,t6136,t6137,t6138,t614,t6141,t6142,t6143,t6144,t6145,t6146,t6147,t615,t6150,t6151,t6152,t6154,t6155,t6157,t6158,t6159,t616,t6160,t6161,t6162,t6164,t6165,t6167,t6169,t6170,t6171,t6172,t6173,t6175,t6176,t6177,t6179,t618,t6180,t6182,t6183,t6185,t6186,t6187,t6188,t6189,t619,t6190,t6191,t6194,t6195,t6196,t6197,t6199,t620,t6200,t6201,t6202,t6203,t6204,t6205,t6206,t6207,t6208,t6209,t621,t6210,t6211,t6212,t6213,t6214,t6215,t6216,t6218,t6219,t622,t6220,t6221,t6222,t6225,t6226,t6227,t6228,t6229,t623,t6230,t6231,t6232,t6235,t6239,t624,t6240,t6241,t6242,t6243,t6244,t6245,t6248,t6249,t625,t6250,t6251,t6252,t6253,t6255,t6256,t6258,t6260,t6262,t6264,t6266,t6267,t6268,t6270,t6271,t6272,t6273,t6274,t6275,t6276,t6277,t6278,t6279,t6280,t6281,t6282,t6283,t6285,t6288,t6289,t6290,t6294,t6296,t6297,t6298,t6299,t6300,t6301,t6302,t6306,t6307,t6308,t6309,t6311,t6312,t6313,t6316,t6317,t6319,t632,t6320,t6322,t6323,t6324,t6326,t6327,t6328,t6329,t6330,t6331,t6332,t6333,t6334,t6335,t6338,t6339,t6341,t6342,t6343,t6345,t6346,t6347,t6348,t6349,t6350,t6351,t6352,t6359,t6360,t6361,t6362,t6364,t6365,t6366,t6367,t6370,t6371,t6374,t6375,t6376,t6378,t6379,t638,t6380,t6382,t6385,t6386,t6387,t6388,t6390,t6391,t6393,t6394,t6395,t6396,t6397,t6398,t6399,t640,t6400,t6401,t6402,t6404,t6405,t6406,t6407,t6408,t6412,t6413,t6414,t6415,t6422,t6423,t6424,t6425,t6426,t6427,t6428,t6429,t6430,t6431,t6432,t6433,t6434,t6435,t6436,t6438,t6439,t6440,t6441,t6442,t6443,t6445,t6447,t6448,t6449,t6450,t6451,t6452,t6453,t6454,t6455,t6456,t6457,t6458,t6459,t6460,t6461,t6462,t6463,t6464,t6465,t6467,t6468,t6469,t6470,t6471,t6472,t6473,t6475,t6476,t6477,t6478,t6481,t6482,t6484,t6485,t6486,t6487,t6488,t6489,t6490,t6493,t6495,t6497,t6498,t6499,t6501,t6502,t6503,t6504,t6505,t6507,t6508,t6509,t6510,t6513,t6514,t6515,t6518,t6519,t6520,t6521,t6522,t6523,t6524,t6525,t6526,t6529,t6530,t6531,t6534,t6535,t6536,t6537,t6538,t6539,t6540,t6541,t6542,t6543,t6544,t6545,t6546,t6547,t6548,t6549,t6550,t6551,t6552,t6555,t6556,t6557,t6558,t6560,t6561,t6562,t6563,t6564,t6566,t6567,t6569,t6570,t6571,t6572,t6573,t6574,t6575,t6576,t6577,t6578,t6579,t6580,t6581,t6582,t6583,t6584,t6585,t6586,t6587,t6589,t6590,t6592,t6593,t6594,t6596,t6597,t6598,t6599,t6600,t6601,t6602,t6603,t6604,t6605,t6606,t6607,t6608,t6610,t6612,t6613,t6615,t6616,t6617,t6621,t6622,t6623,t6624,t6625,t6630,t6631,t6632,t6633,t6634,t6635,t6637,t6638,t6639,t6640,t6641,t6642,t6644,t6646,t6648,t6649,t6650,t6652,t6654,t6656,t6657,t6658,t6659,t6660,t6661,t6662,t6663,t6664,t6665,t6666,t6667,t6668,t6669,t6670,t6671,t6672,t6673,t6674,t6675,t6676,t6677,t6678,t6679,t6680,t6681,t6682,t6683,t6684,t6685,t6686,t6687,t6689,t6691,t6692,t6693,t6694,t6695,t6696,t6697,t6698,t6699,t6700,t6701,t6702,t6704,t6706,t6707,t6708,t6709,t6710,t6711,t6712,t6713,t6714,t6715,t6716,t6717,t6718,t6719,t6720,t6721,t6723,t6724,t6725,t6726,t6727,t6729,t6730,t6732,t6733,t6734,t6735,t6736,t6737,t6738,t6739,t6740,t6741,t6742,t6743,t6744,t6745,t6746,t6748,t6751,t6752,t6753,t6754,t6755,t6756,t6757,t6759,t6764,t6765,t6772,t6773,t6776,t6777,t6785,t6787,t6791,t6792,t6793,t6794,t6795,t6796,t6801,t6802,t6803,t6805,t6806,t6807,t681,t6814,t6815,t6822,t6823,t6826,t6827,t6830,t6831,t6832,t684,t6855,t6856,t6857,t6858,t6859,t6860,t6862,t6863,t6865,t6866,t6867,t6868,t6869,t6870,t6871,t6872,t6873,t6876,t6877,t6879,t6880,t6896,t6902,t6919,t6926,t6927,t6929,t6932,t6933,t6934,t6935,t6937,t6943,t6949,t6951,t6953,t6955,t6958,t6959,t6960,t6963,t6966,t6970,t6971,t6972,t6994,t7,t7000,t7006,t7007,t7008,t7009,t7010,t7011,t7012,t7013,t7015,t7016,t7017,t7018,t7019,t7020,t7022,t7023,t7024,t7025,t7026,t7027,t7028,t7029,t7030,t7031,t7032,t7033,t7034,t7035,t7036,t7039,t7040,t7041,t7042,t7043,t7044,t7045,t7046,t7048,t7051,t7052,t7054,t7055,t7056,t7057,t7060,t7061,t7064,t7065,t7067,t7068,t7069,t7070,t7071,t7078,t7079,t7080,t7082,t7083,t7084,t7085,t7086,t7087,t7088,t7089,t7090,t7091,t7092,t7093,t7094,t7095,t7096,t7097,t7098,t7100,t7101,t7104,t7108,t7109,t7110,t7111,t7113,t7115,t7119,t712,t7140,t7141,t7148,t7149,t7153,t7159,t7162,t7163,t7177,t7178,t7199,t72,t7214,t724,t7244,t7248,t7256,t7258,t7297,t73,t7306,t7334,t7335,t7364,t738,t739,t741,t742,t7528,t753,t7544,t7549,t7550,t7551,t7553,t7557,t7558,t7560,t7564,t7565,t7567,t7568,t7569,t7570,t7571,t7573,t7574,t7575,t7576,t7577,t7578,t7579,t7580,t7581,t760,t781,t792,t796,t797,t8,t803,t81,t825,t826,t827,t830,t832,t845,t847,t848,t852,t856,t86,t861,t866,t868,t869,t874,t875,t877,t878,t881,t893,t899,t9,t90,t902,t903,t905,t908,t909,t91,t910,t911,t912,t915,t917,t919,t922,t925,t926,t928,t929,t930,t931,t932,t934,t940,t944,t945,t947,t95,t952,t954,t955,t957,t958,t968,t970,t971,t972,t975,t976,t984,t985,t986,t989,t99,t991,t998});
end
function C_dq = ft_14(ct)
dq1 = ct{1};
dq2 = ct{2};
dq3 = ct{3};
dq4 = ct{4};
dq5 = ct{5};
dq6 = ct{6};
t1004 = ct{7};
t1016 = ct{8};
t1019 = ct{9};
t1020 = ct{10};
t1031 = ct{11};
t1039 = ct{12};
t1046 = ct{13};
t1050 = ct{14};
t1056 = ct{15};
t1061 = ct{16};
t1069 = ct{17};
t1075 = ct{18};
t1076 = ct{19};
t1077 = ct{20};
t1081 = ct{21};
t1083 = ct{22};
t1088 = ct{23};
t1090 = ct{24};
t1095 = ct{25};
t1099 = ct{26};
t1101 = ct{27};
t1106 = ct{28};
t1108 = ct{29};
t112 = ct{30};
t1122 = ct{31};
t113 = ct{32};
t1133 = ct{33};
t1144 = ct{34};
t1146 = ct{35};
t1147 = ct{36};
t115 = ct{37};
t1150 = ct{38};
t1152 = ct{39};
t1155 = ct{40};
t1156 = ct{41};
t1158 = ct{42};
t116 = ct{43};
t1165 = ct{44};
t1170 = ct{45};
t1171 = ct{46};
t1174 = ct{47};
t1177 = ct{48};
t1179 = ct{49};
t1184 = ct{50};
t1185 = ct{51};
t1191 = ct{52};
t1193 = ct{53};
t1194 = ct{54};
t1196 = ct{55};
t1201 = ct{56};
t1203 = ct{57};
t1205 = ct{58};
t1207 = ct{59};
t121 = ct{60};
t1211 = ct{61};
t1212 = ct{62};
t1213 = ct{63};
t1215 = ct{64};
t1221 = ct{65};
t1224 = ct{66};
t1225 = ct{67};
t1227 = ct{68};
t1228 = ct{69};
t1233 = ct{70};
t1245 = ct{71};
t125 = ct{72};
t1250 = ct{73};
t1253 = ct{74};
t1254 = ct{75};
t1258 = ct{76};
t1273 = ct{77};
t1274 = ct{78};
t1282 = ct{79};
t1285 = ct{80};
t1288 = ct{81};
t1292 = ct{82};
t1300 = ct{83};
t1301 = ct{84};
t1306 = ct{85};
t131 = ct{86};
t1316 = ct{87};
t132 = ct{88};
t1322 = ct{89};
t1323 = ct{90};
t1324 = ct{91};
t133 = ct{92};
t1330 = ct{93};
t1331 = ct{94};
t1333 = ct{95};
t1337 = ct{96};
t1342 = ct{97};
t1344 = ct{98};
t1345 = ct{99};
t1348 = ct{100};
t1353 = ct{101};
t1365 = ct{102};
t1377 = ct{103};
t1379 = ct{104};
t1380 = ct{105};
t1383 = ct{106};
t1388 = ct{107};
t139 = ct{108};
t1391 = ct{109};
t1402 = ct{110};
t1407 = ct{111};
t1409 = ct{112};
t1411 = ct{113};
t1413 = ct{114};
t1419 = ct{115};
t1423 = ct{116};
t1426 = ct{117};
t1427 = ct{118};
t1428 = ct{119};
t1429 = ct{120};
t1436 = ct{121};
t144 = ct{122};
t1440 = ct{123};
t1441 = ct{124};
t1443 = ct{125};
t1445 = ct{126};
t1446 = ct{127};
t1449 = ct{128};
t1454 = ct{129};
t1457 = ct{130};
t1458 = ct{131};
t1460 = ct{132};
t1471 = ct{133};
t148 = ct{134};
t1486 = ct{135};
t1487 = ct{136};
t1489 = ct{137};
t1493 = ct{138};
t1494 = ct{139};
t1495 = ct{140};
t1496 = ct{141};
t15 = ct{142};
t150 = ct{143};
t1503 = ct{144};
t1508 = ct{145};
t1517 = ct{146};
t1520 = ct{147};
t1523 = ct{148};
t1526 = ct{149};
t1530 = ct{150};
t1531 = ct{151};
t1534 = ct{152};
t1537 = ct{153};
t1538 = ct{154};
t1540 = ct{155};
t1541 = ct{156};
t1542 = ct{157};
t1548 = ct{158};
t1550 = ct{159};
t1551 = ct{160};
t156 = ct{161};
t1568 = ct{162};
t1570 = ct{163};
t1574 = ct{164};
t1577 = ct{165};
t1578 = ct{166};
t158 = ct{167};
t1581 = ct{168};
t1582 = ct{169};
t1584 = ct{170};
t1587 = ct{171};
t1590 = ct{172};
t1592 = ct{173};
t1593 = ct{174};
t1594 = ct{175};
t1598 = ct{176};
t16 = ct{177};
t1600 = ct{178};
t1601 = ct{179};
t1602 = ct{180};
t1606 = ct{181};
t1607 = ct{182};
t1609 = ct{183};
t1612 = ct{184};
t1614 = ct{185};
t1615 = ct{186};
t1616 = ct{187};
t1617 = ct{188};
t1619 = ct{189};
t1620 = ct{190};
t1621 = ct{191};
t1622 = ct{192};
t1625 = ct{193};
t1627 = ct{194};
t1630 = ct{195};
t1642 = ct{196};
t1647 = ct{197};
t1648 = ct{198};
t1651 = ct{199};
t1655 = ct{200};
t1656 = ct{201};
t1659 = ct{202};
t166 = ct{203};
t1660 = ct{204};
t1661 = ct{205};
t1667 = ct{206};
t1670 = ct{207};
t1672 = ct{208};
t1674 = ct{209};
t1681 = ct{210};
t1687 = ct{211};
t1692 = ct{212};
t1697 = ct{213};
t1699 = ct{214};
t17 = ct{215};
t1701 = ct{216};
t1704 = ct{217};
t1705 = ct{218};
t1706 = ct{219};
t1707 = ct{220};
t1708 = ct{221};
t171 = ct{222};
t1710 = ct{223};
t1715 = ct{224};
t1716 = ct{225};
t1718 = ct{226};
t1719 = ct{227};
t1721 = ct{228};
t1724 = ct{229};
t1731 = ct{230};
t1732 = ct{231};
t1734 = ct{232};
t1735 = ct{233};
t1736 = ct{234};
t1740 = ct{235};
t1745 = ct{236};
t1747 = ct{237};
t1748 = ct{238};
t1753 = ct{239};
t1754 = ct{240};
t1756 = ct{241};
t1758 = ct{242};
t1759 = ct{243};
t1761 = ct{244};
t1762 = ct{245};
t1766 = ct{246};
t1767 = ct{247};
t1769 = ct{248};
t1770 = ct{249};
t1771 = ct{250};
t1772 = ct{251};
t1775 = ct{252};
t1776 = ct{253};
t1777 = ct{254};
t1781 = ct{255};
t1783 = ct{256};
t1784 = ct{257};
t1792 = ct{258};
t1793 = ct{259};
t1794 = ct{260};
t1795 = ct{261};
t1797 = ct{262};
t1798 = ct{263};
t18 = ct{264};
t1800 = ct{265};
t1805 = ct{266};
t1806 = ct{267};
t1808 = ct{268};
t1811 = ct{269};
t1812 = ct{270};
t1814 = ct{271};
t1815 = ct{272};
t1816 = ct{273};
t1820 = ct{274};
t1821 = ct{275};
t1823 = ct{276};
t1827 = ct{277};
t1828 = ct{278};
t1829 = ct{279};
t183 = ct{280};
t1831 = ct{281};
t1833 = ct{282};
t1834 = ct{283};
t1835 = ct{284};
t1836 = ct{285};
t1839 = ct{286};
t1847 = ct{287};
t185 = ct{288};
t1855 = ct{289};
t1856 = ct{290};
t1858 = ct{291};
t1860 = ct{292};
t1861 = ct{293};
t1863 = ct{294};
t1868 = ct{295};
t1870 = ct{296};
t1873 = ct{297};
t1878 = ct{298};
t1882 = ct{299};
t1884 = ct{300};
t1886 = ct{301};
t1892 = ct{302};
t1899 = ct{303};
t19 = ct{304};
t190 = ct{305};
t1900 = ct{306};
t1902 = ct{307};
t1906 = ct{308};
t1908 = ct{309};
t1909 = ct{310};
t191 = ct{311};
t1913 = ct{312};
t1916 = ct{313};
t1917 = ct{314};
t1922 = ct{315};
t1925 = ct{316};
t1930 = ct{317};
t1937 = ct{318};
t1938 = ct{319};
t1941 = ct{320};
t1942 = ct{321};
t1947 = ct{322};
t1951 = ct{323};
t1952 = ct{324};
t196 = ct{325};
t1967 = ct{326};
t1968 = ct{327};
t1969 = ct{328};
t197 = ct{329};
t1974 = ct{330};
t1977 = ct{331};
t1981 = ct{332};
t1983 = ct{333};
t1984 = ct{334};
t1985 = ct{335};
t1986 = ct{336};
t1989 = ct{337};
t199 = ct{338};
t1992 = ct{339};
t1993 = ct{340};
t1995 = ct{341};
t1997 = ct{342};
t1998 = ct{343};
t1999 = ct{344};
t2 = ct{345};
t20 = ct{346};
t200 = ct{347};
t2002 = ct{348};
t2003 = ct{349};
t2004 = ct{350};
t2006 = ct{351};
t2008 = ct{352};
t201 = ct{353};
t2014 = ct{354};
t2015 = ct{355};
t2017 = ct{356};
t202 = ct{357};
t2026 = ct{358};
t2027 = ct{359};
t2028 = ct{360};
t2034 = ct{361};
t2035 = ct{362};
t2038 = ct{363};
t2039 = ct{364};
t2043 = ct{365};
t2047 = ct{366};
t2050 = ct{367};
t2052 = ct{368};
t2053 = ct{369};
t206 = ct{370};
t2060 = ct{371};
t2062 = ct{372};
t2066 = ct{373};
t2068 = ct{374};
t2069 = ct{375};
t207 = ct{376};
t2070 = ct{377};
t2075 = ct{378};
t2076 = ct{379};
t2077 = ct{380};
t2083 = ct{381};
t2085 = ct{382};
t2088 = ct{383};
t2091 = ct{384};
t2096 = ct{385};
t2098 = ct{386};
t21 = ct{387};
t2106 = ct{388};
t2110 = ct{389};
t2113 = ct{390};
t2115 = ct{391};
t2116 = ct{392};
t2118 = ct{393};
t2119 = ct{394};
t2121 = ct{395};
t2123 = ct{396};
t2128 = ct{397};
t2130 = ct{398};
t2132 = ct{399};
t2133 = ct{400};
t2134 = ct{401};
t2136 = ct{402};
t2142 = ct{403};
t2143 = ct{404};
t2145 = ct{405};
t2149 = ct{406};
t2150 = ct{407};
t2154 = ct{408};
t2158 = ct{409};
t2164 = ct{410};
t2165 = ct{411};
t2177 = ct{412};
t2178 = ct{413};
t2180 = ct{414};
t2181 = ct{415};
t2184 = ct{416};
t2186 = ct{417};
t2187 = ct{418};
t2189 = ct{419};
t2191 = ct{420};
t2192 = ct{421};
t2193 = ct{422};
t2196 = ct{423};
t2197 = ct{424};
t2199 = ct{425};
t22 = ct{426};
t2200 = ct{427};
t2202 = ct{428};
t2203 = ct{429};
t2211 = ct{430};
t2213 = ct{431};
t2214 = ct{432};
t2217 = ct{433};
t2220 = ct{434};
t2224 = ct{435};
t2234 = ct{436};
t2236 = ct{437};
t224 = ct{438};
t2243 = ct{439};
t225 = ct{440};
t2253 = ct{441};
t2256 = ct{442};
t2257 = ct{443};
t2266 = ct{444};
t2267 = ct{445};
t227 = ct{446};
t228 = ct{447};
t2289 = ct{448};
t2291 = ct{449};
t2298 = ct{450};
t2299 = ct{451};
t23 = ct{452};
t230 = ct{453};
t2300 = ct{454};
t2303 = ct{455};
t2304 = ct{456};
t231 = ct{457};
t2312 = ct{458};
t2314 = ct{459};
t2315 = ct{460};
t2320 = ct{461};
t2326 = ct{462};
t233 = ct{463};
t2330 = ct{464};
t2333 = ct{465};
t2334 = ct{466};
t2338 = ct{467};
t234 = ct{468};
t2341 = ct{469};
t2342 = ct{470};
t235 = ct{471};
t236 = ct{472};
t2383 = ct{473};
t2390 = ct{474};
t2392 = ct{475};
t2395 = ct{476};
t2396 = ct{477};
t2397 = ct{478};
t2398 = ct{479};
t24 = ct{480};
t240 = ct{481};
t2416 = ct{482};
t2420 = ct{483};
t2421 = ct{484};
t2424 = ct{485};
t243 = ct{486};
t244 = ct{487};
t2443 = ct{488};
t2444 = ct{489};
t2449 = ct{490};
t2465 = ct{491};
t2466 = ct{492};
t2474 = ct{493};
t2481 = ct{494};
t2483 = ct{495};
t2486 = ct{496};
t249 = ct{497};
t2490 = ct{498};
t2494 = ct{499};
t2497 = ct{500};
t2502 = ct{501};
t2524 = ct{502};
t2525 = ct{503};
t2530 = ct{504};
t2539 = ct{505};
t2544 = ct{506};
t2546 = ct{507};
t2549 = ct{508};
t2552 = ct{509};
t2554 = ct{510};
t2555 = ct{511};
t2556 = ct{512};
t2560 = ct{513};
t2563 = ct{514};
t2564 = ct{515};
t2565 = ct{516};
t2566 = ct{517};
t2567 = ct{518};
t2568 = ct{519};
t2569 = ct{520};
t257 = ct{521};
t2571 = ct{522};
t2574 = ct{523};
t2575 = ct{524};
t2576 = ct{525};
t2578 = ct{526};
t2579 = ct{527};
t258 = ct{528};
t2588 = ct{529};
t2589 = ct{530};
t2597 = ct{531};
t2598 = ct{532};
t2599 = ct{533};
t2611 = ct{534};
t2612 = ct{535};
t2615 = ct{536};
t2617 = ct{537};
t2627 = ct{538};
t263 = ct{539};
t2640 = ct{540};
t2641 = ct{541};
t2655 = ct{542};
t2656 = ct{543};
t266 = ct{544};
t2666 = ct{545};
t2684 = ct{546};
t2686 = ct{547};
t2692 = ct{548};
t2694 = ct{549};
t270 = ct{550};
t2706 = ct{551};
t2720 = ct{552};
t2722 = ct{553};
t2724 = ct{554};
t2726 = ct{555};
t273 = ct{556};
t2737 = ct{557};
t274 = ct{558};
t2741 = ct{559};
t2743 = ct{560};
t2748 = ct{561};
t2749 = ct{562};
t275 = ct{563};
t2753 = ct{564};
t2755 = ct{565};
t2757 = ct{566};
t2759 = ct{567};
t276 = ct{568};
t2761 = ct{569};
t2764 = ct{570};
t277 = ct{571};
t2771 = ct{572};
t2778 = ct{573};
t278 = ct{574};
t2791 = ct{575};
t2793 = ct{576};
t2795 = ct{577};
t2797 = ct{578};
t2798 = ct{579};
t2799 = ct{580};
t280 = ct{581};
t2800 = ct{582};
t2802 = ct{583};
t2806 = ct{584};
t2812 = ct{585};
t2816 = ct{586};
t2818 = ct{587};
t2824 = ct{588};
t2825 = ct{589};
t2827 = ct{590};
t2833 = ct{591};
t2835 = ct{592};
t284 = ct{593};
t2851 = ct{594};
t2857 = ct{595};
t2861 = ct{596};
t2868 = ct{597};
t287 = ct{598};
t2872 = ct{599};
t2877 = ct{600};
t2880 = ct{601};
t2881 = ct{602};
t2893 = ct{603};
t2895 = ct{604};
t2896 = ct{605};
t29 = ct{606};
t290 = ct{607};
t2906 = ct{608};
t291 = ct{609};
t2911 = ct{610};
t2913 = ct{611};
t2916 = ct{612};
t2918 = ct{613};
t292 = ct{614};
t2921 = ct{615};
t2922 = ct{616};
t2932 = ct{617};
t294 = ct{618};
t2941 = ct{619};
t2944 = ct{620};
t2956 = ct{621};
t2958 = ct{622};
t2965 = ct{623};
t297 = ct{624};
t2973 = ct{625};
t2977 = ct{626};
t2987 = ct{627};
t299 = ct{628};
t2999 = ct{629};
t3 = ct{630};
t30 = ct{631};
t300 = ct{632};
t302 = ct{633};
t303 = ct{634};
t304 = ct{635};
t3047 = ct{636};
t305 = ct{637};
t306 = ct{638};
t3083 = ct{639};
t309 = ct{640};
t310 = ct{641};
t311 = ct{642};
t313 = ct{643};
t3136 = ct{644};
t314 = ct{645};
t3142 = ct{646};
t315 = ct{647};
t316 = ct{648};
t318 = ct{649};
t319 = ct{650};
t320 = ct{651};
t3200 = ct{652};
t3209 = ct{653};
t3213 = ct{654};
t3219 = ct{655};
t322 = ct{656};
t3222 = ct{657};
t3224 = ct{658};
t3230 = ct{659};
t3239 = ct{660};
t324 = ct{661};
t3247 = ct{662};
t325 = ct{663};
t3266 = ct{664};
t3268 = ct{665};
t3274 = ct{666};
t328 = ct{667};
t3321 = ct{668};
t333 = ct{669};
t3338 = ct{670};
t336 = ct{671};
t3365 = ct{672};
t3368 = ct{673};
t3369 = ct{674};
t337 = ct{675};
t3375 = ct{676};
t3378 = ct{677};
t3380 = ct{678};
t3383 = ct{679};
t3387 = ct{680};
t3390 = ct{681};
t3391 = ct{682};
t3392 = ct{683};
t3397 = ct{684};
t34 = ct{685};
t340 = ct{686};
t3400 = ct{687};
t3405 = ct{688};
t3407 = ct{689};
t3409 = ct{690};
t3416 = ct{691};
t3417 = ct{692};
t3418 = ct{693};
t3420 = ct{694};
t3422 = ct{695};
t3426 = ct{696};
t3429 = ct{697};
t3430 = ct{698};
t3432 = ct{699};
t3434 = ct{700};
t3435 = ct{701};
t3436 = ct{702};
t3437 = ct{703};
t3439 = ct{704};
t344 = ct{705};
t3440 = ct{706};
t3441 = ct{707};
t3443 = ct{708};
t3444 = ct{709};
t3445 = ct{710};
t3446 = ct{711};
t3449 = ct{712};
t3450 = ct{713};
t3453 = ct{714};
t3457 = ct{715};
t3458 = ct{716};
t346 = ct{717};
t3462 = ct{718};
t3463 = ct{719};
t3464 = ct{720};
t3465 = ct{721};
t3468 = ct{722};
t3469 = ct{723};
t347 = ct{724};
t3471 = ct{725};
t3472 = ct{726};
t3474 = ct{727};
t3475 = ct{728};
t3476 = ct{729};
t3479 = ct{730};
t348 = ct{731};
t3480 = ct{732};
t3483 = ct{733};
t3485 = ct{734};
t3489 = ct{735};
t349 = ct{736};
t3490 = ct{737};
t3491 = ct{738};
t3492 = ct{739};
t3493 = ct{740};
t3496 = ct{741};
t3498 = ct{742};
t3499 = ct{743};
t350 = ct{744};
t3500 = ct{745};
t3501 = ct{746};
t3504 = ct{747};
t3506 = ct{748};
t3507 = ct{749};
t3510 = ct{750};
t3511 = ct{751};
t3513 = ct{752};
t3514 = ct{753};
t3515 = ct{754};
t3517 = ct{755};
t3518 = ct{756};
t352 = ct{757};
t3521 = ct{758};
t3522 = ct{759};
t3523 = ct{760};
t3526 = ct{761};
t353 = ct{762};
t3530 = ct{763};
t3531 = ct{764};
t3532 = ct{765};
t3535 = ct{766};
t3536 = ct{767};
t3539 = ct{768};
t3540 = ct{769};
t3542 = ct{770};
t3543 = ct{771};
t3547 = ct{772};
t3554 = ct{773};
t3556 = ct{774};
t3557 = ct{775};
t356 = ct{776};
t3562 = ct{777};
t3568 = ct{778};
t3569 = ct{779};
t357 = ct{780};
t3571 = ct{781};
t3574 = ct{782};
t3577 = ct{783};
t3578 = ct{784};
t358 = ct{785};
t3582 = ct{786};
t3583 = ct{787};
t3584 = ct{788};
t3585 = ct{789};
t359 = ct{790};
t3592 = ct{791};
t3593 = ct{792};
t3605 = ct{793};
t3606 = ct{794};
t3607 = ct{795};
t361 = ct{796};
t3610 = ct{797};
t3611 = ct{798};
t3612 = ct{799};
t3618 = ct{800};
t362 = ct{801};
t3634 = ct{802};
t3635 = ct{803};
t3637 = ct{804};
t3642 = ct{805};
t3644 = ct{806};
t365 = ct{807};
t3656 = ct{808};
t3658 = ct{809};
t3659 = ct{810};
t3662 = ct{811};
t3666 = ct{812};
t3667 = ct{813};
t3668 = ct{814};
t3672 = ct{815};
t3673 = ct{816};
t3678 = ct{817};
t368 = ct{818};
t3682 = ct{819};
t369 = ct{820};
t3694 = ct{821};
t3702 = ct{822};
t3706 = ct{823};
t3708 = ct{824};
t371 = ct{825};
t3719 = ct{826};
t372 = ct{827};
t3725 = ct{828};
t3726 = ct{829};
t373 = ct{830};
t3732 = ct{831};
t3733 = ct{832};
t3734 = ct{833};
t3738 = ct{834};
t374 = ct{835};
t3743 = ct{836};
t3746 = ct{837};
t3753 = ct{838};
t3755 = ct{839};
t3757 = ct{840};
t3759 = ct{841};
t3761 = ct{842};
t3763 = ct{843};
t3764 = ct{844};
t3765 = ct{845};
t3767 = ct{846};
t377 = ct{847};
t3772 = ct{848};
t378 = ct{849};
t3783 = ct{850};
t3785 = ct{851};
t3788 = ct{852};
t379 = ct{853};
t3792 = ct{854};
t380 = ct{855};
t3819 = ct{856};
t382 = ct{857};
t3821 = ct{858};
t3822 = ct{859};
t3823 = ct{860};
t3824 = ct{861};
t3831 = ct{862};
t384 = ct{863};
t3843 = ct{864};
t3845 = ct{865};
t3851 = ct{866};
t3852 = ct{867};
t3853 = ct{868};
t386 = ct{869};
t3863 = ct{870};
t3869 = ct{871};
t387 = ct{872};
t3871 = ct{873};
t3873 = ct{874};
t3874 = ct{875};
t3875 = ct{876};
t3876 = ct{877};
t388 = ct{878};
t3882 = ct{879};
t3884 = ct{880};
t3889 = ct{881};
t3890 = ct{882};
t3891 = ct{883};
t3907 = ct{884};
t391 = ct{885};
t3910 = ct{886};
t3913 = ct{887};
t392 = ct{888};
t3921 = ct{889};
t3922 = ct{890};
t3923 = ct{891};
t3944 = ct{892};
t395 = ct{893};
t3951 = ct{894};
t3954 = ct{895};
t3956 = ct{896};
t3957 = ct{897};
t3959 = ct{898};
t396 = ct{899};
t3960 = ct{900};
t3968 = ct{901};
t3969 = ct{902};
t3971 = ct{903};
t3972 = ct{904};
t3976 = ct{905};
t3978 = ct{906};
t3979 = ct{907};
t3992 = ct{908};
t3993 = ct{909};
t3995 = ct{910};
t3997 = ct{911};
t4 = ct{912};
t400 = ct{913};
t4000 = ct{914};
t4004 = ct{915};
t401 = ct{916};
t4010 = ct{917};
t4011 = ct{918};
t4014 = ct{919};
t4015 = ct{920};
t402 = ct{921};
t403 = ct{922};
t406 = ct{923};
t4089 = ct{924};
t4099 = ct{925};
t410 = ct{926};
t4100 = ct{927};
t4103 = ct{928};
t4108 = ct{929};
t411 = ct{930};
t4113 = ct{931};
t4115 = ct{932};
t4118 = ct{933};
t4119 = ct{934};
t412 = ct{935};
t4121 = ct{936};
t4123 = ct{937};
t4126 = ct{938};
t413 = ct{939};
t4132 = ct{940};
t4134 = ct{941};
t4138 = ct{942};
t414 = ct{943};
t4143 = ct{944};
t4146 = ct{945};
t4148 = ct{946};
t415 = ct{947};
t4152 = ct{948};
t4153 = ct{949};
t4158 = ct{950};
t416 = ct{951};
t4166 = ct{952};
t417 = ct{953};
t4173 = ct{954};
t4178 = ct{955};
t4179 = ct{956};
t418 = ct{957};
t4181 = ct{958};
t4183 = ct{959};
t4185 = ct{960};
t4190 = ct{961};
t4196 = ct{962};
t4197 = ct{963};
t420 = ct{964};
t4206 = ct{965};
t4208 = ct{966};
t4210 = ct{967};
t4217 = ct{968};
t422 = ct{969};
t4221 = ct{970};
t4223 = ct{971};
t4226 = ct{972};
t4228 = ct{973};
t423 = ct{974};
t4230 = ct{975};
t4232 = ct{976};
t4234 = ct{977};
t424 = ct{978};
t4243 = ct{979};
t4249 = ct{980};
t425 = ct{981};
t4250 = ct{982};
t4251 = ct{983};
t4254 = ct{984};
t4255 = ct{985};
t4259 = ct{986};
t4261 = ct{987};
t4263 = ct{988};
t427 = ct{989};
t4274 = ct{990};
t4276 = ct{991};
t4278 = ct{992};
t4279 = ct{993};
t428 = ct{994};
t4285 = ct{995};
t4286 = ct{996};
t429 = ct{997};
t4293 = ct{998};
t4298 = ct{999};
t4301 = ct{1000};
t4304 = ct{1001};
t4305 = ct{1002};
t4306 = ct{1003};
t431 = ct{1004};
t4317 = ct{1005};
t4318 = ct{1006};
t432 = ct{1007};
t4327 = ct{1008};
t4329 = ct{1009};
t433 = ct{1010};
t4332 = ct{1011};
t4335 = ct{1012};
t4337 = ct{1013};
t4339 = ct{1014};
t434 = ct{1015};
t4342 = ct{1016};
t4344 = ct{1017};
t4345 = ct{1018};
t4347 = ct{1019};
t4348 = ct{1020};
t4349 = ct{1021};
t435 = ct{1022};
t4350 = ct{1023};
t436 = ct{1024};
t4369 = ct{1025};
t437 = ct{1026};
t4370 = ct{1027};
t4378 = ct{1028};
t438 = ct{1029};
t4380 = ct{1030};
t4382 = ct{1031};
t4385 = ct{1032};
t4388 = ct{1033};
t439 = ct{1034};
t4392 = ct{1035};
t4394 = ct{1036};
t4395 = ct{1037};
t4396 = ct{1038};
t4397 = ct{1039};
t440 = ct{1040};
t4402 = ct{1041};
t4403 = ct{1042};
t4405 = ct{1043};
t4406 = ct{1044};
t4407 = ct{1045};
t441 = ct{1046};
t4410 = ct{1047};
t4412 = ct{1048};
t4413 = ct{1049};
t4414 = ct{1050};
t4416 = ct{1051};
t4417 = ct{1052};
t4418 = ct{1053};
t4419 = ct{1054};
t442 = ct{1055};
t4420 = ct{1056};
t4423 = ct{1057};
t4425 = ct{1058};
t4426 = ct{1059};
t4428 = ct{1060};
t4429 = ct{1061};
t4431 = ct{1062};
t4436 = ct{1063};
t4437 = ct{1064};
t444 = ct{1065};
t4440 = ct{1066};
t4444 = ct{1067};
t4446 = ct{1068};
t4447 = ct{1069};
t4449 = ct{1070};
t445 = ct{1071};
t4450 = ct{1072};
t4453 = ct{1073};
t4462 = ct{1074};
t4467 = ct{1075};
t4468 = ct{1076};
t4469 = ct{1077};
t4471 = ct{1078};
t4473 = ct{1079};
t4475 = ct{1080};
t4478 = ct{1081};
t4479 = ct{1082};
t448 = ct{1083};
t4482 = ct{1084};
t4483 = ct{1085};
t4485 = ct{1086};
t4486 = ct{1087};
t4487 = ct{1088};
t4488 = ct{1089};
t4489 = ct{1090};
t449 = ct{1091};
t4490 = ct{1092};
t4494 = ct{1093};
t4495 = ct{1094};
t4498 = ct{1095};
t4499 = ct{1096};
t45 = ct{1097};
t450 = ct{1098};
t4500 = ct{1099};
t4501 = ct{1100};
t4502 = ct{1101};
t4505 = ct{1102};
t4506 = ct{1103};
t4509 = ct{1104};
t4510 = ct{1105};
t4515 = ct{1106};
t4518 = ct{1107};
t4519 = ct{1108};
t452 = ct{1109};
t4520 = ct{1110};
t4521 = ct{1111};
t4522 = ct{1112};
t4523 = ct{1113};
t4526 = ct{1114};
t4527 = ct{1115};
t4528 = ct{1116};
t453 = ct{1117};
t4530 = ct{1118};
t4534 = ct{1119};
t4536 = ct{1120};
t4538 = ct{1121};
t454 = ct{1122};
t4541 = ct{1123};
t4543 = ct{1124};
t4545 = ct{1125};
t4546 = ct{1126};
t4549 = ct{1127};
t4551 = ct{1128};
t4552 = ct{1129};
t4553 = ct{1130};
t4556 = ct{1131};
t4557 = ct{1132};
t4558 = ct{1133};
t4559 = ct{1134};
t4565 = ct{1135};
t4568 = ct{1136};
t457 = ct{1137};
t4570 = ct{1138};
t4572 = ct{1139};
t4575 = ct{1140};
t4577 = ct{1141};
t4578 = ct{1142};
t458 = ct{1143};
t4581 = ct{1144};
t4582 = ct{1145};
t4586 = ct{1146};
t4587 = ct{1147};
t4588 = ct{1148};
t4589 = ct{1149};
t459 = ct{1150};
t4590 = ct{1151};
t4591 = ct{1152};
t4592 = ct{1153};
t4593 = ct{1154};
t4595 = ct{1155};
t4596 = ct{1156};
t4598 = ct{1157};
t460 = ct{1158};
t4600 = ct{1159};
t4601 = ct{1160};
t4602 = ct{1161};
t4604 = ct{1162};
t4605 = ct{1163};
t4606 = ct{1164};
t4607 = ct{1165};
t4608 = ct{1166};
t461 = ct{1167};
t4614 = ct{1168};
t4616 = ct{1169};
t4619 = ct{1170};
t462 = ct{1171};
t4621 = ct{1172};
t4622 = ct{1173};
t4623 = ct{1174};
t4624 = ct{1175};
t4625 = ct{1176};
t4626 = ct{1177};
t4629 = ct{1178};
t463 = ct{1179};
t4633 = ct{1180};
t4634 = ct{1181};
t4636 = ct{1182};
t464 = ct{1183};
t4644 = ct{1184};
t4645 = ct{1185};
t4647 = ct{1186};
t4648 = ct{1187};
t465 = ct{1188};
t4654 = ct{1189};
t4656 = ct{1190};
t4659 = ct{1191};
t466 = ct{1192};
t4660 = ct{1193};
t4666 = ct{1194};
t4667 = ct{1195};
t4669 = ct{1196};
t4673 = ct{1197};
t4674 = ct{1198};
t4675 = ct{1199};
t4678 = ct{1200};
t468 = ct{1201};
t4682 = ct{1202};
t469 = ct{1203};
t4694 = ct{1204};
t4695 = ct{1205};
t4696 = ct{1206};
t4697 = ct{1207};
t470 = ct{1208};
t4707 = ct{1209};
t4708 = ct{1210};
t471 = ct{1211};
t472 = ct{1212};
t4724 = ct{1213};
t4727 = ct{1214};
t4728 = ct{1215};
t4731 = ct{1216};
t4732 = ct{1217};
t4733 = ct{1218};
t4737 = ct{1219};
t4738 = ct{1220};
t4739 = ct{1221};
t4742 = ct{1222};
t4743 = ct{1223};
t4745 = ct{1224};
t4747 = ct{1225};
t4748 = ct{1226};
t475 = ct{1227};
t4755 = ct{1228};
t4756 = ct{1229};
t4762 = ct{1230};
t4763 = ct{1231};
t477 = ct{1232};
t4773 = ct{1233};
t4775 = ct{1234};
t4780 = ct{1235};
t4781 = ct{1236};
t4782 = ct{1237};
t4783 = ct{1238};
t4785 = ct{1239};
t4786 = ct{1240};
t479 = ct{1241};
t480 = ct{1242};
t481 = ct{1243};
t4810 = ct{1244};
t482 = ct{1245};
t4824 = ct{1246};
t483 = ct{1247};
t4838 = ct{1248};
t4842 = ct{1249};
t485 = ct{1250};
t486 = ct{1251};
t4864 = ct{1252};
t4866 = ct{1253};
t4869 = ct{1254};
t4870 = ct{1255};
t488 = ct{1256};
t4884 = ct{1257};
t489 = ct{1258};
t4903 = ct{1259};
t4904 = ct{1260};
t491 = ct{1261};
t4911 = ct{1262};
t4914 = ct{1263};
t4919 = ct{1264};
t492 = ct{1265};
t493 = ct{1266};
t4934 = ct{1267};
t4936 = ct{1268};
t494 = ct{1269};
t4950 = ct{1270};
t4953 = ct{1271};
t4957 = ct{1272};
t496 = ct{1273};
t497 = ct{1274};
t4973 = ct{1275};
t498 = ct{1276};
t4981 = ct{1277};
t4983 = ct{1278};
t4984 = ct{1279};
t4987 = ct{1280};
t499 = ct{1281};
t4990 = ct{1282};
t4993 = ct{1283};
t4994 = ct{1284};
t4995 = ct{1285};
t4996 = ct{1286};
t5 = ct{1287};
t50 = ct{1288};
t500 = ct{1289};
t5000 = ct{1290};
t5002 = ct{1291};
t5007 = ct{1292};
t5008 = ct{1293};
t5009 = ct{1294};
t501 = ct{1295};
t502 = ct{1296};
t5021 = ct{1297};
t5022 = ct{1298};
t5023 = ct{1299};
t5026 = ct{1300};
t5027 = ct{1301};
t503 = ct{1302};
t5032 = ct{1303};
t5039 = ct{1304};
t504 = ct{1305};
t505 = ct{1306};
t5058 = ct{1307};
t506 = ct{1308};
t5061 = ct{1309};
t5063 = ct{1310};
t5065 = ct{1311};
t507 = ct{1312};
t5075 = ct{1313};
t5076 = ct{1314};
t508 = ct{1315};
t5080 = ct{1316};
t5084 = ct{1317};
t5086 = ct{1318};
t5087 = ct{1319};
t509 = ct{1320};
t5097 = ct{1321};
t5099 = ct{1322};
t510 = ct{1323};
t5102 = ct{1324};
t5107 = ct{1325};
t511 = ct{1326};
t5112 = ct{1327};
t5114 = ct{1328};
t512 = ct{1329};
t5121 = ct{1330};
t5123 = ct{1331};
t513 = ct{1332};
t5132 = ct{1333};
t5136 = ct{1334};
t514 = ct{1335};
t5147 = ct{1336};
t5150 = ct{1337};
t5151 = ct{1338};
t516 = ct{1339};
t5164 = ct{1340};
t5166 = ct{1341};
t517 = ct{1342};
t518 = ct{1343};
t5184 = ct{1344};
t5195 = ct{1345};
t520 = ct{1346};
t5203 = ct{1347};
t5204 = ct{1348};
t5206 = ct{1349};
t521 = ct{1350};
t5210 = ct{1351};
t5215 = ct{1352};
t5217 = ct{1353};
t5219 = ct{1354};
t522 = ct{1355};
t5227 = ct{1356};
t5228 = ct{1357};
t523 = ct{1358};
t5232 = ct{1359};
t5233 = ct{1360};
t5236 = ct{1361};
t5238 = ct{1362};
t524 = ct{1363};
t5242 = ct{1364};
t5244 = ct{1365};
t5249 = ct{1366};
t525 = ct{1367};
t5251 = ct{1368};
t5255 = ct{1369};
t5258 = ct{1370};
t5259 = ct{1371};
t526 = ct{1372};
t5262 = ct{1373};
t5269 = ct{1374};
t527 = ct{1375};
t5275 = ct{1376};
t5279 = ct{1377};
t528 = ct{1378};
t5280 = ct{1379};
t5285 = ct{1380};
t529 = ct{1381};
t5297 = ct{1382};
t53 = ct{1383};
t530 = ct{1384};
t531 = ct{1385};
t5316 = ct{1386};
t5318 = ct{1387};
t532 = ct{1388};
t5320 = ct{1389};
t5323 = ct{1390};
t5324 = ct{1391};
t533 = ct{1392};
t5333 = ct{1393};
t5339 = ct{1394};
t534 = ct{1395};
t5344 = ct{1396};
t535 = ct{1397};
t5354 = ct{1398};
t536 = ct{1399};
t537 = ct{1400};
t5370 = ct{1401};
t538 = ct{1402};
t539 = ct{1403};
t540 = ct{1404};
t543 = ct{1405};
t544 = ct{1406};
t5443 = ct{1407};
t545 = ct{1408};
t5450 = ct{1409};
t5457 = ct{1410};
t5459 = ct{1411};
t546 = ct{1412};
t5464 = ct{1413};
t5465 = ct{1414};
t5466 = ct{1415};
t547 = ct{1416};
t548 = ct{1417};
t5480 = ct{1418};
t5482 = ct{1419};
t5483 = ct{1420};
t5484 = ct{1421};
t5486 = ct{1422};
t5487 = ct{1423};
t5488 = ct{1424};
t549 = ct{1425};
t5507 = ct{1426};
t551 = ct{1427};
t552 = ct{1428};
t5521 = ct{1429};
t553 = ct{1430};
t554 = ct{1431};
t555 = ct{1432};
t556 = ct{1433};
t557 = ct{1434};
t558 = ct{1435};
t559 = ct{1436};
t560 = ct{1437};
t5602 = ct{1438};
t5605 = ct{1439};
t561 = ct{1440};
t562 = ct{1441};
t5621 = ct{1442};
t5622 = ct{1443};
t563 = ct{1444};
t5633 = ct{1445};
t5634 = ct{1446};
t5636 = ct{1447};
t564 = ct{1448};
t5647 = ct{1449};
t5648 = ct{1450};
t5657 = ct{1451};
t5658 = ct{1452};
t5662 = ct{1453};
t5665 = ct{1454};
t5666 = ct{1455};
t567 = ct{1456};
t5670 = ct{1457};
t5676 = ct{1458};
t5677 = ct{1459};
t5679 = ct{1460};
t568 = ct{1461};
t5683 = ct{1462};
t5684 = ct{1463};
t5688 = ct{1464};
t569 = ct{1465};
t5691 = ct{1466};
t5699 = ct{1467};
t57 = ct{1468};
t570 = ct{1469};
t5700 = ct{1470};
t5702 = ct{1471};
t5704 = ct{1472};
t5706 = ct{1473};
t5708 = ct{1474};
t5709 = ct{1475};
t571 = ct{1476};
t5710 = ct{1477};
t5717 = ct{1478};
t5718 = ct{1479};
t572 = ct{1480};
t5729 = ct{1481};
t573 = ct{1482};
t5730 = ct{1483};
t5735 = ct{1484};
t5738 = ct{1485};
t5739 = ct{1486};
t574 = ct{1487};
t5740 = ct{1488};
t5742 = ct{1489};
t5744 = ct{1490};
t5750 = ct{1491};
t5755 = ct{1492};
t5756 = ct{1493};
t5757 = ct{1494};
t576 = ct{1495};
t5762 = ct{1496};
t5766 = ct{1497};
t5767 = ct{1498};
t5769 = ct{1499};
t5770 = ct{1500};
t5772 = ct{1501};
t5774 = ct{1502};
t5775 = ct{1503};
t5776 = ct{1504};
t5778 = ct{1505};
t578 = ct{1506};
t5784 = ct{1507};
t5786 = ct{1508};
t5787 = ct{1509};
t5790 = ct{1510};
t5791 = ct{1511};
t5792 = ct{1512};
t5794 = ct{1513};
t5795 = ct{1514};
t5797 = ct{1515};
t580 = ct{1516};
t5808 = ct{1517};
t581 = ct{1518};
t5810 = ct{1519};
t582 = ct{1520};
t5822 = ct{1521};
t5823 = ct{1522};
t5824 = ct{1523};
t5825 = ct{1524};
t5826 = ct{1525};
t5831 = ct{1526};
t5838 = ct{1527};
t5839 = ct{1528};
t584 = ct{1529};
t5840 = ct{1530};
t5841 = ct{1531};
t5842 = ct{1532};
t5844 = ct{1533};
t5845 = ct{1534};
t5846 = ct{1535};
t5847 = ct{1536};
t5848 = ct{1537};
t5849 = ct{1538};
t5850 = ct{1539};
t5851 = ct{1540};
t5852 = ct{1541};
t5859 = ct{1542};
t586 = ct{1543};
t5861 = ct{1544};
t587 = ct{1545};
t5872 = ct{1546};
t5878 = ct{1547};
t5881 = ct{1548};
t5882 = ct{1549};
t5883 = ct{1550};
t5888 = ct{1551};
t5889 = ct{1552};
t589 = ct{1553};
t5892 = ct{1554};
t5894 = ct{1555};
t5895 = ct{1556};
t5897 = ct{1557};
t5898 = ct{1558};
t5899 = ct{1559};
t590 = ct{1560};
t5900 = ct{1561};
t5901 = ct{1562};
t5904 = ct{1563};
t5905 = ct{1564};
t5907 = ct{1565};
t5909 = ct{1566};
t591 = ct{1567};
t5911 = ct{1568};
t5912 = ct{1569};
t5914 = ct{1570};
t5915 = ct{1571};
t5916 = ct{1572};
t5917 = ct{1573};
t5918 = ct{1574};
t5919 = ct{1575};
t592 = ct{1576};
t5920 = ct{1577};
t5921 = ct{1578};
t5922 = ct{1579};
t5923 = ct{1580};
t5924 = ct{1581};
t5925 = ct{1582};
t5926 = ct{1583};
t5928 = ct{1584};
t5929 = ct{1585};
t593 = ct{1586};
t5930 = ct{1587};
t5931 = ct{1588};
t5932 = ct{1589};
t5933 = ct{1590};
t5934 = ct{1591};
t5935 = ct{1592};
t5936 = ct{1593};
t5937 = ct{1594};
t5938 = ct{1595};
t5939 = ct{1596};
t594 = ct{1597};
t5940 = ct{1598};
t5941 = ct{1599};
t5942 = ct{1600};
t5943 = ct{1601};
t5944 = ct{1602};
t5945 = ct{1603};
t5946 = ct{1604};
t5947 = ct{1605};
t5948 = ct{1606};
t5949 = ct{1607};
t595 = ct{1608};
t5950 = ct{1609};
t5951 = ct{1610};
t5952 = ct{1611};
t5953 = ct{1612};
t5954 = ct{1613};
t5956 = ct{1614};
t5957 = ct{1615};
t5958 = ct{1616};
t5959 = ct{1617};
t596 = ct{1618};
t5960 = ct{1619};
t5961 = ct{1620};
t5962 = ct{1621};
t5964 = ct{1622};
t5965 = ct{1623};
t5966 = ct{1624};
t5967 = ct{1625};
t5968 = ct{1626};
t597 = ct{1627};
t5970 = ct{1628};
t5971 = ct{1629};
t5972 = ct{1630};
t5973 = ct{1631};
t5974 = ct{1632};
t5975 = ct{1633};
t5976 = ct{1634};
t5977 = ct{1635};
t5978 = ct{1636};
t5979 = ct{1637};
t5980 = ct{1638};
t5981 = ct{1639};
t5982 = ct{1640};
t5983 = ct{1641};
t5984 = ct{1642};
t5985 = ct{1643};
t5986 = ct{1644};
t5987 = ct{1645};
t5988 = ct{1646};
t5989 = ct{1647};
t5991 = ct{1648};
t5993 = ct{1649};
t5994 = ct{1650};
t5995 = ct{1651};
t5996 = ct{1652};
t5997 = ct{1653};
t5998 = ct{1654};
t5999 = ct{1655};
t6 = ct{1656};
t60 = ct{1657};
t600 = ct{1658};
t6000 = ct{1659};
t6001 = ct{1660};
t6002 = ct{1661};
t6003 = ct{1662};
t6004 = ct{1663};
t6005 = ct{1664};
t6007 = ct{1665};
t6008 = ct{1666};
t6009 = ct{1667};
t6010 = ct{1668};
t6011 = ct{1669};
t6012 = ct{1670};
t6013 = ct{1671};
t6014 = ct{1672};
t6016 = ct{1673};
t6017 = ct{1674};
t6019 = ct{1675};
t602 = ct{1676};
t6020 = ct{1677};
t6024 = ct{1678};
t6025 = ct{1679};
t6026 = ct{1680};
t6028 = ct{1681};
t6029 = ct{1682};
t603 = ct{1683};
t6030 = ct{1684};
t6032 = ct{1685};
t6035 = ct{1686};
t6037 = ct{1687};
t6038 = ct{1688};
t604 = ct{1689};
t6040 = ct{1690};
t6041 = ct{1691};
t6042 = ct{1692};
t6043 = ct{1693};
t6044 = ct{1694};
t6045 = ct{1695};
t6046 = ct{1696};
t6047 = ct{1697};
t6048 = ct{1698};
t6049 = ct{1699};
t605 = ct{1700};
t6051 = ct{1701};
t6052 = ct{1702};
t6053 = ct{1703};
t6054 = ct{1704};
t6055 = ct{1705};
t6056 = ct{1706};
t6057 = ct{1707};
t6060 = ct{1708};
t6061 = ct{1709};
t6062 = ct{1710};
t6063 = ct{1711};
t6064 = ct{1712};
t6065 = ct{1713};
t6067 = ct{1714};
t6068 = ct{1715};
t6069 = ct{1716};
t6073 = ct{1717};
t6074 = ct{1718};
t6075 = ct{1719};
t6076 = ct{1720};
t6077 = ct{1721};
t6078 = ct{1722};
t6079 = ct{1723};
t6080 = ct{1724};
t6081 = ct{1725};
t6083 = ct{1726};
t6085 = ct{1727};
t6086 = ct{1728};
t609 = ct{1729};
t6093 = ct{1730};
t6094 = ct{1731};
t6095 = ct{1732};
t610 = ct{1733};
t6103 = ct{1734};
t6108 = ct{1735};
t6109 = ct{1736};
t611 = ct{1737};
t6110 = ct{1738};
t6111 = ct{1739};
t6113 = ct{1740};
t6114 = ct{1741};
t6116 = ct{1742};
t6118 = ct{1743};
t6119 = ct{1744};
t612 = ct{1745};
t6120 = ct{1746};
t6121 = ct{1747};
t6123 = ct{1748};
t6125 = ct{1749};
t6126 = ct{1750};
t6127 = ct{1751};
t6128 = ct{1752};
t6129 = ct{1753};
t613 = ct{1754};
t6130 = ct{1755};
t6131 = ct{1756};
t6132 = ct{1757};
t6134 = ct{1758};
t6135 = ct{1759};
t6136 = ct{1760};
t6137 = ct{1761};
t6138 = ct{1762};
t614 = ct{1763};
t6141 = ct{1764};
t6142 = ct{1765};
t6143 = ct{1766};
t6144 = ct{1767};
t6145 = ct{1768};
t6146 = ct{1769};
t6147 = ct{1770};
t615 = ct{1771};
t6150 = ct{1772};
t6151 = ct{1773};
t6152 = ct{1774};
t6154 = ct{1775};
t6155 = ct{1776};
t6157 = ct{1777};
t6158 = ct{1778};
t6159 = ct{1779};
t616 = ct{1780};
t6160 = ct{1781};
t6161 = ct{1782};
t6162 = ct{1783};
t6164 = ct{1784};
t6165 = ct{1785};
t6167 = ct{1786};
t6169 = ct{1787};
t6170 = ct{1788};
t6171 = ct{1789};
t6172 = ct{1790};
t6173 = ct{1791};
t6175 = ct{1792};
t6176 = ct{1793};
t6177 = ct{1794};
t6179 = ct{1795};
t618 = ct{1796};
t6180 = ct{1797};
t6182 = ct{1798};
t6183 = ct{1799};
t6185 = ct{1800};
t6186 = ct{1801};
t6187 = ct{1802};
t6188 = ct{1803};
t6189 = ct{1804};
t619 = ct{1805};
t6190 = ct{1806};
t6191 = ct{1807};
t6194 = ct{1808};
t6195 = ct{1809};
t6196 = ct{1810};
t6197 = ct{1811};
t6199 = ct{1812};
t620 = ct{1813};
t6200 = ct{1814};
t6201 = ct{1815};
t6202 = ct{1816};
t6203 = ct{1817};
t6204 = ct{1818};
t6205 = ct{1819};
t6206 = ct{1820};
t6207 = ct{1821};
t6208 = ct{1822};
t6209 = ct{1823};
t621 = ct{1824};
t6210 = ct{1825};
t6211 = ct{1826};
t6212 = ct{1827};
t6213 = ct{1828};
t6214 = ct{1829};
t6215 = ct{1830};
t6216 = ct{1831};
t6218 = ct{1832};
t6219 = ct{1833};
t622 = ct{1834};
t6220 = ct{1835};
t6221 = ct{1836};
t6222 = ct{1837};
t6225 = ct{1838};
t6226 = ct{1839};
t6227 = ct{1840};
t6228 = ct{1841};
t6229 = ct{1842};
t623 = ct{1843};
t6230 = ct{1844};
t6231 = ct{1845};
t6232 = ct{1846};
t6235 = ct{1847};
t6239 = ct{1848};
t624 = ct{1849};
t6240 = ct{1850};
t6241 = ct{1851};
t6242 = ct{1852};
t6243 = ct{1853};
t6244 = ct{1854};
t6245 = ct{1855};
t6248 = ct{1856};
t6249 = ct{1857};
t625 = ct{1858};
t6250 = ct{1859};
t6251 = ct{1860};
t6252 = ct{1861};
t6253 = ct{1862};
t6255 = ct{1863};
t6256 = ct{1864};
t6258 = ct{1865};
t6260 = ct{1866};
t6262 = ct{1867};
t6264 = ct{1868};
t6266 = ct{1869};
t6267 = ct{1870};
t6268 = ct{1871};
t6270 = ct{1872};
t6271 = ct{1873};
t6272 = ct{1874};
t6273 = ct{1875};
t6274 = ct{1876};
t6275 = ct{1877};
t6276 = ct{1878};
t6277 = ct{1879};
t6278 = ct{1880};
t6279 = ct{1881};
t6280 = ct{1882};
t6281 = ct{1883};
t6282 = ct{1884};
t6283 = ct{1885};
t6285 = ct{1886};
t6288 = ct{1887};
t6289 = ct{1888};
t6290 = ct{1889};
t6294 = ct{1890};
t6296 = ct{1891};
t6297 = ct{1892};
t6298 = ct{1893};
t6299 = ct{1894};
t6300 = ct{1895};
t6301 = ct{1896};
t6302 = ct{1897};
t6306 = ct{1898};
t6307 = ct{1899};
t6308 = ct{1900};
t6309 = ct{1901};
t6311 = ct{1902};
t6312 = ct{1903};
t6313 = ct{1904};
t6316 = ct{1905};
t6317 = ct{1906};
t6319 = ct{1907};
t632 = ct{1908};
t6320 = ct{1909};
t6322 = ct{1910};
t6323 = ct{1911};
t6324 = ct{1912};
t6326 = ct{1913};
t6327 = ct{1914};
t6328 = ct{1915};
t6329 = ct{1916};
t6330 = ct{1917};
t6331 = ct{1918};
t6332 = ct{1919};
t6333 = ct{1920};
t6334 = ct{1921};
t6335 = ct{1922};
t6338 = ct{1923};
t6339 = ct{1924};
t6341 = ct{1925};
t6342 = ct{1926};
t6343 = ct{1927};
t6345 = ct{1928};
t6346 = ct{1929};
t6347 = ct{1930};
t6348 = ct{1931};
t6349 = ct{1932};
t6350 = ct{1933};
t6351 = ct{1934};
t6352 = ct{1935};
t6359 = ct{1936};
t6360 = ct{1937};
t6361 = ct{1938};
t6362 = ct{1939};
t6364 = ct{1940};
t6365 = ct{1941};
t6366 = ct{1942};
t6367 = ct{1943};
t6370 = ct{1944};
t6371 = ct{1945};
t6374 = ct{1946};
t6375 = ct{1947};
t6376 = ct{1948};
t6378 = ct{1949};
t6379 = ct{1950};
t638 = ct{1951};
t6380 = ct{1952};
t6382 = ct{1953};
t6385 = ct{1954};
t6386 = ct{1955};
t6387 = ct{1956};
t6388 = ct{1957};
t6390 = ct{1958};
t6391 = ct{1959};
t6393 = ct{1960};
t6394 = ct{1961};
t6395 = ct{1962};
t6396 = ct{1963};
t6397 = ct{1964};
t6398 = ct{1965};
t6399 = ct{1966};
t640 = ct{1967};
t6400 = ct{1968};
t6401 = ct{1969};
t6402 = ct{1970};
t6404 = ct{1971};
t6405 = ct{1972};
t6406 = ct{1973};
t6407 = ct{1974};
t6408 = ct{1975};
t6412 = ct{1976};
t6413 = ct{1977};
t6414 = ct{1978};
t6415 = ct{1979};
t6422 = ct{1980};
t6423 = ct{1981};
t6424 = ct{1982};
t6425 = ct{1983};
t6426 = ct{1984};
t6427 = ct{1985};
t6428 = ct{1986};
t6429 = ct{1987};
t6430 = ct{1988};
t6431 = ct{1989};
t6432 = ct{1990};
t6433 = ct{1991};
t6434 = ct{1992};
t6435 = ct{1993};
t6436 = ct{1994};
t6438 = ct{1995};
t6439 = ct{1996};
t6440 = ct{1997};
t6441 = ct{1998};
t6442 = ct{1999};
t6443 = ct{2000};
t6445 = ct{2001};
t6447 = ct{2002};
t6448 = ct{2003};
t6449 = ct{2004};
t6450 = ct{2005};
t6451 = ct{2006};
t6452 = ct{2007};
t6453 = ct{2008};
t6454 = ct{2009};
t6455 = ct{2010};
t6456 = ct{2011};
t6457 = ct{2012};
t6458 = ct{2013};
t6459 = ct{2014};
t6460 = ct{2015};
t6461 = ct{2016};
t6462 = ct{2017};
t6463 = ct{2018};
t6464 = ct{2019};
t6465 = ct{2020};
t6467 = ct{2021};
t6468 = ct{2022};
t6469 = ct{2023};
t6470 = ct{2024};
t6471 = ct{2025};
t6472 = ct{2026};
t6473 = ct{2027};
t6475 = ct{2028};
t6476 = ct{2029};
t6477 = ct{2030};
t6478 = ct{2031};
t6481 = ct{2032};
t6482 = ct{2033};
t6484 = ct{2034};
t6485 = ct{2035};
t6486 = ct{2036};
t6487 = ct{2037};
t6488 = ct{2038};
t6489 = ct{2039};
t6490 = ct{2040};
t6493 = ct{2041};
t6495 = ct{2042};
t6497 = ct{2043};
t6498 = ct{2044};
t6499 = ct{2045};
t6501 = ct{2046};
t6502 = ct{2047};
t6503 = ct{2048};
t6504 = ct{2049};
t6505 = ct{2050};
t6507 = ct{2051};
t6508 = ct{2052};
t6509 = ct{2053};
t6510 = ct{2054};
t6513 = ct{2055};
t6514 = ct{2056};
t6515 = ct{2057};
t6518 = ct{2058};
t6519 = ct{2059};
t6520 = ct{2060};
t6521 = ct{2061};
t6522 = ct{2062};
t6523 = ct{2063};
t6524 = ct{2064};
t6525 = ct{2065};
t6526 = ct{2066};
t6529 = ct{2067};
t6530 = ct{2068};
t6531 = ct{2069};
t6534 = ct{2070};
t6535 = ct{2071};
t6536 = ct{2072};
t6537 = ct{2073};
t6538 = ct{2074};
t6539 = ct{2075};
t6540 = ct{2076};
t6541 = ct{2077};
t6542 = ct{2078};
t6543 = ct{2079};
t6544 = ct{2080};
t6545 = ct{2081};
t6546 = ct{2082};
t6547 = ct{2083};
t6548 = ct{2084};
t6549 = ct{2085};
t6550 = ct{2086};
t6551 = ct{2087};
t6552 = ct{2088};
t6555 = ct{2089};
t6556 = ct{2090};
t6557 = ct{2091};
t6558 = ct{2092};
t6560 = ct{2093};
t6561 = ct{2094};
t6562 = ct{2095};
t6563 = ct{2096};
t6564 = ct{2097};
t6566 = ct{2098};
t6567 = ct{2099};
t6569 = ct{2100};
t6570 = ct{2101};
t6571 = ct{2102};
t6572 = ct{2103};
t6573 = ct{2104};
t6574 = ct{2105};
t6575 = ct{2106};
t6576 = ct{2107};
t6577 = ct{2108};
t6578 = ct{2109};
t6579 = ct{2110};
t6580 = ct{2111};
t6581 = ct{2112};
t6582 = ct{2113};
t6583 = ct{2114};
t6584 = ct{2115};
t6585 = ct{2116};
t6586 = ct{2117};
t6587 = ct{2118};
t6589 = ct{2119};
t6590 = ct{2120};
t6592 = ct{2121};
t6593 = ct{2122};
t6594 = ct{2123};
t6596 = ct{2124};
t6597 = ct{2125};
t6598 = ct{2126};
t6599 = ct{2127};
t6600 = ct{2128};
t6601 = ct{2129};
t6602 = ct{2130};
t6603 = ct{2131};
t6604 = ct{2132};
t6605 = ct{2133};
t6606 = ct{2134};
t6607 = ct{2135};
t6608 = ct{2136};
t6610 = ct{2137};
t6612 = ct{2138};
t6613 = ct{2139};
t6615 = ct{2140};
t6616 = ct{2141};
t6617 = ct{2142};
t6621 = ct{2143};
t6622 = ct{2144};
t6623 = ct{2145};
t6624 = ct{2146};
t6625 = ct{2147};
t6630 = ct{2148};
t6631 = ct{2149};
t6632 = ct{2150};
t6633 = ct{2151};
t6634 = ct{2152};
t6635 = ct{2153};
t6637 = ct{2154};
t6638 = ct{2155};
t6639 = ct{2156};
t6640 = ct{2157};
t6641 = ct{2158};
t6642 = ct{2159};
t6644 = ct{2160};
t6646 = ct{2161};
t6648 = ct{2162};
t6649 = ct{2163};
t6650 = ct{2164};
t6652 = ct{2165};
t6654 = ct{2166};
t6656 = ct{2167};
t6657 = ct{2168};
t6658 = ct{2169};
t6659 = ct{2170};
t6660 = ct{2171};
t6661 = ct{2172};
t6662 = ct{2173};
t6663 = ct{2174};
t6664 = ct{2175};
t6665 = ct{2176};
t6666 = ct{2177};
t6667 = ct{2178};
t6668 = ct{2179};
t6669 = ct{2180};
t6670 = ct{2181};
t6671 = ct{2182};
t6672 = ct{2183};
t6673 = ct{2184};
t6674 = ct{2185};
t6675 = ct{2186};
t6676 = ct{2187};
t6677 = ct{2188};
t6678 = ct{2189};
t6679 = ct{2190};
t6680 = ct{2191};
t6681 = ct{2192};
t6682 = ct{2193};
t6683 = ct{2194};
t6684 = ct{2195};
t6685 = ct{2196};
t6686 = ct{2197};
t6687 = ct{2198};
t6689 = ct{2199};
t6691 = ct{2200};
t6692 = ct{2201};
t6693 = ct{2202};
t6694 = ct{2203};
t6695 = ct{2204};
t6696 = ct{2205};
t6697 = ct{2206};
t6698 = ct{2207};
t6699 = ct{2208};
t6700 = ct{2209};
t6701 = ct{2210};
t6702 = ct{2211};
t6704 = ct{2212};
t6706 = ct{2213};
t6707 = ct{2214};
t6708 = ct{2215};
t6709 = ct{2216};
t6710 = ct{2217};
t6711 = ct{2218};
t6712 = ct{2219};
t6713 = ct{2220};
t6714 = ct{2221};
t6715 = ct{2222};
t6716 = ct{2223};
t6717 = ct{2224};
t6718 = ct{2225};
t6719 = ct{2226};
t6720 = ct{2227};
t6721 = ct{2228};
t6723 = ct{2229};
t6724 = ct{2230};
t6725 = ct{2231};
t6726 = ct{2232};
t6727 = ct{2233};
t6729 = ct{2234};
t6730 = ct{2235};
t6732 = ct{2236};
t6733 = ct{2237};
t6734 = ct{2238};
t6735 = ct{2239};
t6736 = ct{2240};
t6737 = ct{2241};
t6738 = ct{2242};
t6739 = ct{2243};
t6740 = ct{2244};
t6741 = ct{2245};
t6742 = ct{2246};
t6743 = ct{2247};
t6744 = ct{2248};
t6745 = ct{2249};
t6746 = ct{2250};
t6748 = ct{2251};
t6751 = ct{2252};
t6752 = ct{2253};
t6753 = ct{2254};
t6754 = ct{2255};
t6755 = ct{2256};
t6756 = ct{2257};
t6757 = ct{2258};
t6759 = ct{2259};
t6764 = ct{2260};
t6765 = ct{2261};
t6772 = ct{2262};
t6773 = ct{2263};
t6776 = ct{2264};
t6777 = ct{2265};
t6785 = ct{2266};
t6787 = ct{2267};
t6791 = ct{2268};
t6792 = ct{2269};
t6793 = ct{2270};
t6794 = ct{2271};
t6795 = ct{2272};
t6796 = ct{2273};
t6801 = ct{2274};
t6802 = ct{2275};
t6803 = ct{2276};
t6805 = ct{2277};
t6806 = ct{2278};
t6807 = ct{2279};
t681 = ct{2280};
t6814 = ct{2281};
t6815 = ct{2282};
t6822 = ct{2283};
t6823 = ct{2284};
t6826 = ct{2285};
t6827 = ct{2286};
t6830 = ct{2287};
t6831 = ct{2288};
t6832 = ct{2289};
t684 = ct{2290};
t6855 = ct{2291};
t6856 = ct{2292};
t6857 = ct{2293};
t6858 = ct{2294};
t6859 = ct{2295};
t6860 = ct{2296};
t6862 = ct{2297};
t6863 = ct{2298};
t6865 = ct{2299};
t6866 = ct{2300};
t6867 = ct{2301};
t6868 = ct{2302};
t6869 = ct{2303};
t6870 = ct{2304};
t6871 = ct{2305};
t6872 = ct{2306};
t6873 = ct{2307};
t6876 = ct{2308};
t6877 = ct{2309};
t6879 = ct{2310};
t6880 = ct{2311};
t6896 = ct{2312};
t6902 = ct{2313};
t6919 = ct{2314};
t6926 = ct{2315};
t6927 = ct{2316};
t6929 = ct{2317};
t6932 = ct{2318};
t6933 = ct{2319};
t6934 = ct{2320};
t6935 = ct{2321};
t6937 = ct{2322};
t6943 = ct{2323};
t6949 = ct{2324};
t6951 = ct{2325};
t6953 = ct{2326};
t6955 = ct{2327};
t6958 = ct{2328};
t6959 = ct{2329};
t6960 = ct{2330};
t6963 = ct{2331};
t6966 = ct{2332};
t6970 = ct{2333};
t6971 = ct{2334};
t6972 = ct{2335};
t6994 = ct{2336};
t7 = ct{2337};
t7000 = ct{2338};
t7006 = ct{2339};
t7007 = ct{2340};
t7008 = ct{2341};
t7009 = ct{2342};
t7010 = ct{2343};
t7011 = ct{2344};
t7012 = ct{2345};
t7013 = ct{2346};
t7015 = ct{2347};
t7016 = ct{2348};
t7017 = ct{2349};
t7018 = ct{2350};
t7019 = ct{2351};
t7020 = ct{2352};
t7022 = ct{2353};
t7023 = ct{2354};
t7024 = ct{2355};
t7025 = ct{2356};
t7026 = ct{2357};
t7027 = ct{2358};
t7028 = ct{2359};
t7029 = ct{2360};
t7030 = ct{2361};
t7031 = ct{2362};
t7032 = ct{2363};
t7033 = ct{2364};
t7034 = ct{2365};
t7035 = ct{2366};
t7036 = ct{2367};
t7039 = ct{2368};
t7040 = ct{2369};
t7041 = ct{2370};
t7042 = ct{2371};
t7043 = ct{2372};
t7044 = ct{2373};
t7045 = ct{2374};
t7046 = ct{2375};
t7048 = ct{2376};
t7051 = ct{2377};
t7052 = ct{2378};
t7054 = ct{2379};
t7055 = ct{2380};
t7056 = ct{2381};
t7057 = ct{2382};
t7060 = ct{2383};
t7061 = ct{2384};
t7064 = ct{2385};
t7065 = ct{2386};
t7067 = ct{2387};
t7068 = ct{2388};
t7069 = ct{2389};
t7070 = ct{2390};
t7071 = ct{2391};
t7078 = ct{2392};
t7079 = ct{2393};
t7080 = ct{2394};
t7082 = ct{2395};
t7083 = ct{2396};
t7084 = ct{2397};
t7085 = ct{2398};
t7086 = ct{2399};
t7087 = ct{2400};
t7088 = ct{2401};
t7089 = ct{2402};
t7090 = ct{2403};
t7091 = ct{2404};
t7092 = ct{2405};
t7093 = ct{2406};
t7094 = ct{2407};
t7095 = ct{2408};
t7096 = ct{2409};
t7097 = ct{2410};
t7098 = ct{2411};
t7100 = ct{2412};
t7101 = ct{2413};
t7104 = ct{2414};
t7108 = ct{2415};
t7109 = ct{2416};
t7110 = ct{2417};
t7111 = ct{2418};
t7113 = ct{2419};
t7115 = ct{2420};
t7119 = ct{2421};
t712 = ct{2422};
t7140 = ct{2423};
t7141 = ct{2424};
t7148 = ct{2425};
t7149 = ct{2426};
t7153 = ct{2427};
t7159 = ct{2428};
t7162 = ct{2429};
t7163 = ct{2430};
t7177 = ct{2431};
t7178 = ct{2432};
t7199 = ct{2433};
t72 = ct{2434};
t7214 = ct{2435};
t724 = ct{2436};
t7244 = ct{2437};
t7248 = ct{2438};
t7256 = ct{2439};
t7258 = ct{2440};
t7297 = ct{2441};
t73 = ct{2442};
t7306 = ct{2443};
t7334 = ct{2444};
t7335 = ct{2445};
t7364 = ct{2446};
t738 = ct{2447};
t739 = ct{2448};
t741 = ct{2449};
t742 = ct{2450};
t7528 = ct{2451};
t753 = ct{2452};
t7544 = ct{2453};
t7549 = ct{2454};
t7550 = ct{2455};
t7551 = ct{2456};
t7553 = ct{2457};
t7557 = ct{2458};
t7558 = ct{2459};
t7560 = ct{2460};
t7564 = ct{2461};
t7565 = ct{2462};
t7567 = ct{2463};
t7568 = ct{2464};
t7569 = ct{2465};
t7570 = ct{2466};
t7571 = ct{2467};
t7573 = ct{2468};
t7574 = ct{2469};
t7575 = ct{2470};
t7576 = ct{2471};
t7577 = ct{2472};
t7578 = ct{2473};
t7579 = ct{2474};
t7580 = ct{2475};
t7581 = ct{2476};
t760 = ct{2477};
t781 = ct{2478};
t792 = ct{2479};
t796 = ct{2480};
t797 = ct{2481};
t8 = ct{2482};
t803 = ct{2483};
t81 = ct{2484};
t825 = ct{2485};
t826 = ct{2486};
t827 = ct{2487};
t830 = ct{2488};
t832 = ct{2489};
t845 = ct{2490};
t847 = ct{2491};
t848 = ct{2492};
t852 = ct{2493};
t856 = ct{2494};
t86 = ct{2495};
t861 = ct{2496};
t866 = ct{2497};
t868 = ct{2498};
t869 = ct{2499};
t874 = ct{2500};
t875 = ct{2501};
t877 = ct{2502};
t878 = ct{2503};
t881 = ct{2504};
t893 = ct{2505};
t899 = ct{2506};
t9 = ct{2507};
t90 = ct{2508};
t902 = ct{2509};
t903 = ct{2510};
t905 = ct{2511};
t908 = ct{2512};
t909 = ct{2513};
t91 = ct{2514};
t910 = ct{2515};
t911 = ct{2516};
t912 = ct{2517};
t915 = ct{2518};
t917 = ct{2519};
t919 = ct{2520};
t922 = ct{2521};
t925 = ct{2522};
t926 = ct{2523};
t928 = ct{2524};
t929 = ct{2525};
t930 = ct{2526};
t931 = ct{2527};
t932 = ct{2528};
t934 = ct{2529};
t940 = ct{2530};
t944 = ct{2531};
t945 = ct{2532};
t947 = ct{2533};
t95 = ct{2534};
t952 = ct{2535};
t954 = ct{2536};
t955 = ct{2537};
t957 = ct{2538};
t958 = ct{2539};
t968 = ct{2540};
t970 = ct{2541};
t971 = ct{2542};
t972 = ct{2543};
t975 = ct{2544};
t976 = ct{2545};
t984 = ct{2546};
t985 = ct{2547};
t986 = ct{2548};
t989 = ct{2549};
t99 = ct{2550};
t991 = ct{2551};
t998 = ct{2552};
t6758 = t139.*t5861.*t6470;
t6760 = t5824.*t6470.*(t29-t30).*(-7.596454196607839e-68);
t6761 = t6695.*4.126305279697715e-13;
t6766 = t91.*t5822.*t6465.*5.520609140571798e-70;
t6768 = t91.*t5822.*t6465.*5.517689141340903e-72;
t6774 = t91.*t5822.*t6465.*1.065477564130357e-78;
t6779 = t91.*t5824.*t6465.*1.015171749786156e-71;
t6781 = t91.*t5824.*t6465.*5.520609140571798e-70;
t6782 = t5822.*t6470.*(t29-t30).*(-1.015171749786156e-71);
t6783 = t91.*t5824.*t6465.*5.517689141340903e-72;
t6784 = t5822.*t6470.*(t29-t30).*(-5.520609140571798e-70);
t6789 = t5822.*t6470.*(t29-t30).*1.015171749786156e-71;
t6790 = t5822.*t6470.*(t29-t30).*5.520609140571798e-70;
t6797 = t91.*t5824.*t6465.*1.065477564130357e-78;
t6799 = t5822.*t6470.*(t29-t30).*(-1.065477564130357e-78);
t6804 = t5822.*t6470.*(t29-t30).*1.065477564130357e-78;
t6808 = t5824.*t6470.*(t29-t30).*(-1.015171749786156e-71);
t6809 = t5824.*t6470.*(t29-t30).*(-5.520609140571798e-70);
t6811 = t5824.*t6470.*(t29-t30).*(-5.517689141340903e-72);
t6812 = t5824.*t6470.*(t29-t30).*5.520609140571798e-70;
t6817 = t5824.*t6470.*(t29-t30).*(-1.065477564130357e-78);
t6818 = t5824.*t6470.*(t29-t30).*1.065477564130357e-78;
t6821 = t5666+t6220+t6239;
t6824 = -t6822;
t6825 = -t6823;
t6834 = t6822.*7.26350610236655e-5;
t6835 = t6823.*1.33637579258949e-4;
t6836 = t6822.*1.744166498897461e-6;
t6838 = t6822.*1.246862701090643e-6;
t6841 = t6822.*2.179051830709965e-7;
t6842 = t6823.*4.00912737776847e-7;
t6843 = t6823.*1.246862701090643e-6;
t6844 = t6823.*3.383302988283333e-6;
t6846 = t6822.*1.40259855e-11;
t6847 = t6822.*4.126305279697715e-13;
t6849 = t6823.*3.146556677756745e-13;
t6851 = t6823.*1.40259855e-11;
t6875 = -t6465.*(t5670+t4.*(t1458-t5665));
t6878 = t6103.*t6470;
t6881 = t6465.*(t5670+t4.*(t1458-t5665)).*(-7.26350610236655e-5);
t6882 = t6876.*1.33637579258949e-4;
t6883 = t6465.*(t5670+t4.*(t1458-t5665)).*(-1.744166498897461e-6);
t6884 = t6465.*(t5670+t4.*(t1458-t5665)).*(-1.246862701090643e-6);
t6885 = t6465.*(t5670+t4.*(t1458-t5665)).*1.246862701090643e-6;
t6888 = t6876.*4.00912737776847e-7;
t6889 = t6876.*1.246862701090643e-6;
t6890 = t6876.*3.383302988283333e-6;
t6891 = t6465.*(t5670+t4.*(t1458-t5665)).*(-2.179051830709965e-7);
t6894 = t6465.*(t5670+t4.*(t1458-t5665)).*2.179051830709965e-7;
t6897 = t6465.*(t5670+t4.*(t1458-t5665)).*(-1.40259855e-11);
t6898 = t6876.*3.146556677756745e-13;
t6900 = t6465.*(t5670+t4.*(t1458-t5665)).*(-4.126305279697715e-13);
t6903 = t6876.*1.40259855e-11;
t6906 = t6877.*7.26350610236655e-5;
t6908 = t6877.*1.744166498897461e-6;
t6909 = t6877.*1.246862701090643e-6;
t6915 = t6877.*2.179051830709965e-7;
t6920 = t6877.*1.40259855e-11;
t6922 = t6877.*4.126305279697715e-13;
t6928 = t6213.*t6465;
t6930 = t6216.*t6465;
t6936 = t6222.*t6470;
t6938 = -t6935;
t6939 = t6230.*t6470;
t6973 = t6935.*7.26350610236655e-5;
t6975 = t6937.*1.33637579258949e-4;
t6976 = t6935.*1.744166498897461e-6;
t6977 = t6935.*1.246862701090643e-6;
t6979 = t6937.*7.26350610236655e-5;
t6981 = t6937.*1.744166498897461e-6;
t6983 = t6937.*1.246862701090643e-6;
t6985 = t6937.*3.383302988283333e-6;
t6992 = t6935.*1.40259855e-11;
t6993 = t6935.*4.126305279697715e-13;
t6996 = t6937.*3.146556677756745e-13;
t6999 = t6937.*1.40259855e-11;
t7001 = t6937.*4.126305279697715e-13;
t7037 = t6359.*(t5831-t6095+t5679.*(t2088-t4743).*8.081970098144003e-70).*(-1.0./2.0);
t7038 = t6401.*(t5808-t6019+t5679.*(t2088-t4743).*3.038581678643136e-64).*(-1.0./2.0);
et18 = t5888+t5795.*(t2088-t4743).*8.081970098144003e-70;
et19 = t5683.*(t197.*(t29-t30).*9.007199254740992e+15+t3.*(t2444-t2449)).*8.081970098144003e-70;
t7049 = t6359.*(et18+et19).*(-1.0./2.0);
et20 = t5842+t5795.*(t2088-t4743).*3.038581678643136e-64;
et21 = t5683.*(t197.*(t29-t30).*9.007199254740992e+15+t3.*(t2444-t2449)).*3.038581678643136e-64;
t7050 = t6401.*(et20+et21).*(-1.0./2.0);
t7053 = t5859+t6464+t6467;
t7063 = t6010+t6486+t6497;
t7066 = t520.*(t6005-t6486+(t5824.*t6230.*(t29-t30))./1.316403645856965e+67).*(-1.0./2.0);
t7072 = t5929+t6596+t6598;
t7077 = t5957+t6623+t6634;
t7103 = ((t6005-t6486+(t5824.*t6230.*(t29-t30))./1.316403645856965e+67).*(t4148.*1.33637579258949e-4-t5087+t45.*(t2421-t4158)+t60.*(t2421-t4158)))./2.0;
t7114 = t6558.*(t6005-t6486+(t5824.*t6230.*(t29-t30))./1.316403645856965e+67).*(-1.0./2.0);
t7116 = (t6558.*(t6005-t6486+(t5824.*t6230.*(t29-t30))./1.316403645856965e+67))./2.0;
t7120 = t6597.*(t6005-t6486+(t5824.*t6230.*(t29-t30))./1.316403645856965e+67).*(-1.0./2.0);
t7121 = (t6597.*(t6005-t6486+(t5824.*t6230.*(t29-t30))./1.316403645856965e+67))./2.0;
t7143 = t1426.*(-t5881+t5918+t6412+t6414+(t4.*t5824.*t5861.*(t29-t30))./1.316403645856965e+67+(t4.*t91.*t5824.*(t3136-t5691))./1.316403645856965e+67).*(-1.0./2.0);
t7152 = t230+t266+t276+t400+t5912+t5932+t6376+t6388+t6424+t6429;
t7170 = t6700.*(t6313+(t91.*t5824.*(t6218+t5.*(t3136-t5691)))./1.316403645856965e+67+(t5824.*t6470.*(t29-t30))./1.316403645856965e+67).*(-1.0./2.0);
t7171 = (t6700.*(t6313+(t91.*t5824.*(t6218+t5.*(t3136-t5691)))./1.316403645856965e+67+(t5824.*t6470.*(t29-t30))./1.316403645856965e+67))./2.0;
t7173 = t6776.*(t6313+(t91.*t5824.*(t6218+t5.*(t3136-t5691)))./1.316403645856965e+67+(t5824.*t6470.*(t29-t30))./1.316403645856965e+67).*(-1.0./2.0);
t7176 = t5930+t6013+t6438+t6439+t6484+t6495;
t7181 = t5962+t6215+t6440+t6441+t6473+t6478;
t7183 = t6994.*(t6313+(t91.*t5824.*(t6218+t5.*(t3136-t5691)))./1.316403645856965e+67+(t5824.*t6470.*(t29-t30))./1.316403645856965e+67).*(-1.0./2.0);
t7184 = t5987+t6274+t6457+t6460+t6503+t6508;
t7186 = t243+t270+t292+t365+t5946+t6077+t6448+t6453+t6515+t6531;
t7194 = t7027.*(t6313+(t91.*t5824.*(t6218+t5.*(t3136-t5691)))./1.316403645856965e+67+(t5824.*t6470.*(t29-t30))./1.316403645856965e+67).*(-1.0./2.0);
t7195 = (t7027.*(t6313+(t91.*t5824.*(t6218+t5.*(t3136-t5691)))./1.316403645856965e+67+(t5824.*t6470.*(t29-t30))./1.316403645856965e+67))./2.0;
t7209 = t6919.*(-t5881+t5918+t6412+t6414+(t4.*t5824.*t5861.*(t29-t30))./1.316403645856965e+67+(t4.*t91.*t5824.*(t3136-t5691))./1.316403645856965e+67).*(-1.0./2.0);
t7273 = t1471.*(t5984+t5988-t6694-t6695+t6230.*(t5878+t9.*(t7.*(t3719-t3788)+(t3.*t34.*t191.*(t29-t30))./8.112963841460668e+31))+t4.*t6465.*(t3136-t5691)).*(-1.0./2.0);
t7388 = t7085.*(t5984+t5988-t6694-t6695+t6230.*(t5878+t9.*(t7.*(t3719-t3788)+(t3.*t34.*t191.*(t29-t30))./8.112963841460668e+31))+t4.*t6465.*(t3136-t5691)).*(-1.0./2.0);
et22 = t284-t311+t391-t463+t534+t5947-t6009.*1.40259855e-11+t6013.*7.26350610236655e-5-t6194+t6449+t6454-t6513+t6544+t6551;
et23 = t91.*t5684.*(t6218+t5.*(t3136-t5691)).*1.065477564130357e-78-t4.*t7.*t9.*1.07175327657342e-6;
et24 = t5824.*t6222.*(t29-t30).*5.517689141340903e-72;
et25 = t5684.*t6470.*(t29-t30).*1.065477564130357e-78;
t7437 = ((t4148+t5.*(t2421-t4158)).*(et22+et23+et24+et25))./2.0;
t7467 = t7248.*(t5984+t5988-t6694-t6695+t6230.*(t5878+t9.*(t7.*(t3719-t3788)+(t3.*t34.*t191.*(t29-t30))./8.112963841460668e+31))+t4.*t6465.*(t3136-t5691)).*(-1.0./2.0);
t6284 = -t6282;
t6292 = t6226.*(-7.26350610236655e-5);
t6293 = t6226.*(-1.246862701090643e-6);
t6295 = t6226.*(-1.744166498897461e-6);
t6303 = -t6302;
t6314 = t6226.*1.40259855e-11;
t6315 = t6227.*1.40259855e-11;
t6444 = -t6443;
t6446 = -t6445;
t6492 = -t6489;
t6595 = -t6593;
t6620 = -t6617;
t6703 = -t6701;
t6728 = -t6724;
t6747 = t6697.*4.00912737776847e-7;
t6749 = t6697.*1.246862701090643e-6;
t6750 = t6697.*3.383302988283333e-6;
t6762 = t6697.*1.40259855e-11;
t6763 = t6697.*(-3.146556677756745e-13);
t6767 = -t6766;
t6771 = -t6768;
t6786 = -t6779;
t6788 = -t6781;
t6798 = -t6797;
t6837 = -t6834;
t6839 = -t6835;
t6840 = -t6836;
t6845 = -t6843;
t6848 = -t6846;
t6850 = -t6847;
t6892 = -t6888;
t6893 = -t6890;
t6901 = -t6898;
t6904 = -t6903;
t6907 = t6878.*1.33637579258949e-4;
t6910 = -t6909;
t6911 = t6878.*4.00912737776847e-7;
t6913 = t6878.*1.246862701090643e-6;
t6914 = t6878.*3.383302988283333e-6;
t6918 = -t6915;
t6921 = t6878.*3.146556677756745e-13;
t6924 = t6878.*1.40259855e-11;
t6931 = -t6928;
t6941 = (t4763.*t6821)./2.0;
t6942 = t6928.*7.26350610236655e-5;
t6944 = t6930.*1.33637579258949e-4;
t6945 = t6928.*1.744166498897461e-6;
t6946 = t6928.*1.246862701090643e-6;
t6948 = t6930.*7.26350610236655e-5;
t6950 = t6930.*1.744166498897461e-6;
t6952 = t6930.*1.246862701090643e-6;
t6954 = t6930.*3.383302988283333e-6;
t6961 = t6928.*1.40259855e-11;
t6962 = t6928.*4.126305279697715e-13;
t6964 = t6930.*3.146556677756745e-13;
t6967 = t6930.*1.40259855e-11;
t6968 = t6930.*4.126305279697715e-13;
t6974 = t6936.*1.33637579258949e-4;
t6978 = -t6975;
t6980 = t6939.*1.33637579258949e-4;
t6982 = t6936.*1.246862701090643e-6;
t6984 = t6936.*3.383302988283333e-6;
t6986 = t6939.*7.26350610236655e-5;
t6987 = -t6983;
t6988 = -t6985;
t6989 = t6939.*1.744166498897461e-6;
t6990 = t6939.*1.246862701090643e-6;
t6991 = t6939.*3.383302988283333e-6;
t6995 = t6936.*3.146556677756745e-13;
t6997 = -t6993;
t6998 = t6936.*1.40259855e-11;
t7002 = t6939.*3.146556677756745e-13;
t7003 = t6939.*1.40259855e-11;
t7005 = t6939.*4.126305279697715e-13;
t7058 = (t640.*t7053)./2.0;
t7073 = (t640.*t7072)./2.0;
t7075 = t225+t227+t274+t291+t294+t368+t6068+t6520+t6536;
t7076 = (t4742.*t7072)./2.0;
t7081 = (t4742.*t7077)./2.0;
t7105 = t6319+t6729+t6754;
t7106 = t6320+t6736+t6760;
t7117 = t503+t530+t555+t6338+t6781+t6801;
t7118 = t499+t502+t554+t6335+t6792+t6809;
t7122 = t206+t228+t462+t537+t574+t6333+t6794+t6812;
t7124 = t303+t324+t344+t359+t388+t396+t6347+t6797+t6814;
t7125 = t319+t346+t353+t369+t382+t392+t6346+t6802+t6817;
t7128 = t5.*(t305-t319+t322+t336+t6345+t6807+t6818-t5.*t7.*t8.*2.908151843953269e-6-t7.*t8.*t9.*1.07175327657342e-6).*(-1.0./2.0);
t7129 = t6191+t6932+t6939;
t7130 = t6197+t6930+t6937;
t7138 = t5881+t5920+t6366+t6367+t6413+t6415;
et26 = t741+t868+t1568+t1834-t3274-t3391-t3440+t3874+t3891+t4348+t5259+t5742+t5757-t5.*t8.*1.133811468776912e-7;
et27 = t5.*t201.*(-6.364473664374288e-6)+t8.*t3365+t8.*t3449;
et28 = t4.*t5.*t7.*(-1.907069379620846e-7);
et29 = t8.*t9.*t190.*(-6.800564119502148e-6);
et30 = t3.*t4.*t5.*t34.*t191.*(-7.138318981153782e-22);
t7139 = t6821.*(et26+et27+et28+et29+et30).*(-1.0./2.0);
t7142 = (t6821.*t7065)./2.0;
t7146 = t5872.*(t305-t319+t322+t336+t6345+t6807+t6818-t5.*t7.*t8.*2.908151843953269e-6-t7.*t8.*t9.*1.07175327657342e-6).*(-1.0./2.0);
t7147 = (t5872.*(t305-t319+t322+t336+t6345+t6807+t6818-t5.*t7.*t8.*2.908151843953269e-6-t7.*t8.*t9.*1.07175327657342e-6))./2.0;
t7154 = (t6821.*t7078)./2.0;
t7165 = t6462.*(t462+t537+t574+t6333+t6794+t6812).*(-1.0./2.0);
t7168 = t6702.*(-t6729+t5784.*(t4148+t5.*(t2421-t4158))+(t5824.*t6468.*(t29-t30))./1.316403645856965e+67).*(-1.0./2.0);
t7169 = (t6702.*(-t6729+t5784.*(t4148+t5.*(t2421-t4158))+(t5824.*t6468.*(t29-t30))./1.316403645856965e+67))./2.0;
t7174 = t6795.*(-t6729+t5784.*(t4148+t5.*(t2421-t4158))+(t5824.*t6468.*(t29-t30))./1.316403645856965e+67).*(-1.0./2.0);
t7175 = (t6795.*(-t6729+t5784.*(t4148+t5.*(t2421-t4158))+(t5824.*t6468.*(t29-t30))./1.316403645856965e+67))./2.0;
t7179 = (t6136.*t7152)./2.0;
t7182 = t7000.*(-t6729+t5784.*(t4148+t5.*(t2421-t4158))+(t5824.*t6468.*(t29-t30))./1.316403645856965e+67).*(-1.0./2.0);
t7185 = (t6821.*t7119)./2.0;
t7191 = t5677+t6196+t6227+t6253+t6929+t6936;
t7193 = t7026.*(-t6729+t5784.*(t4148+t5.*(t2421-t4158))+(t5824.*t6468.*(t29-t30))./1.316403645856965e+67).*(-1.0./2.0);
t7215 = t6009+t6120+t6493+t6502+t6673+t6675;
t7216 = t6016+t6126+t6490+t6499+t6672+t6674;
t7217 = (t6136.*t7186)./2.0;
t7219 = t5997+t6110+t6570+t6573+t6612+t6615;
t7220 = t6000+t6111+t6572+t6575+t6610+t6613;
t7223 = t5.*(t6109+t6571+t6574-t6610+t4528.*(t4148+t5.*(t2421-t4158))+(t4838.*t6468.*(t29-t30))./1.316403645856965e+67).*(-7.01299275e-12);
t7224 = t5.*(t6109+t6571+t6574-t6610+t4528.*(t4148+t5.*(t2421-t4158))+(t4838.*t6468.*(t29-t30))./1.316403645856965e+67).*7.01299275e-12;
t7225 = (t6832.*t7152)./2.0;
t7226 = (t7053.*t7109)./2.0;
t7227 = t224+t501+t570+t6054+t6132+t6577+t6583+t6622+t6633;
t7228 = t337+t500+t552+t6061+t6129+t6581+t6587+t6616+t6625;
t7229 = t207+t244+t504+t571+t6076+t6169+t6525+t6541+t6679+t6685;
t7230 = t231+t299+t507+t573+t6080+t6180+t6522+t6538+t6676+t6681;
t7238 = t7060.*(t462+t537+t574+t6333+t6794+t6812).*(-1.0./2.0);
t7240 = (t7060.*(t462+t537+t574+t6333+t6794+t6812))./2.0;
et31 = t741+t868+t1568+t1735+t1834+t1969+t1998+t2116-t3274-t3391-t3440+t3672+t3764+t3823+t3853+t3874+t3891+t4250+t4305+t4348+t5259+t5742+t5757-t5.*t8.*1.133811468776912e-7;
et32 = t5.*t201.*(-6.364473664374288e-6)+t8.*t3365+t8.*t3449;
et33 = t2.*t5.*t8.*(-3.96815841743287e-6);
et34 = t4.*t5.*t7.*(-1.907069379620846e-7);
et35 = t6.*t8.*t9.*(-1.769880715106441e-6);
et36 = t8.*t9.*t190.*(-6.800564119502148e-6);
et37 = t2.*t5.*t201.*(-9.619703863182361e-7);
et38 = t5.*t6.*t201.*(-3.96815841743287e-6);
et39 = t2.*t4.*t5.*t7.*(-6.674437170347525e-6);
et40 = t4.*t6.*t7.*t9.*(-2.976937004352228e-6);
et41 = t2.*t8.*t9.*t190.*(-2.976937004352228e-6);
et42 = t6.*t8.*t9.*t190.*(-1.22799597575967e-5);
et43 = t3.*t4.*t5.*t34.*t191.*(-7.138318981153782e-22);
et44 = t2.*t3.*t4.*t5.*t34.*t191.*(-2.089880210625419e-22);
et45 = t3.*t4.*t5.*t6.*t34.*t191.*(-8.620822290548326e-22);
t7257 = t6821.*(et31+et32+et33+et34+et35+et36+et37+et38+et39+et40+et41+et42+et43+et44+et45).*(-1.0./2.0);
et46 = t741+t868+t1568+t1735+t1834+t1969+t1998+t2116-t3274-t3391-t3440+t3672+t3764+t3823+t3853+t3874+t3891+t4250+t4305+t4348+t5259+t5742+t5757-t5.*t8.*1.133811468776912e-7;
et47 = t5.*t201.*(-6.364473664374288e-6)+t8.*t3365+t8.*t3449;
et48 = t2.*t5.*t8.*(-3.96815841743287e-6);
et49 = t4.*t5.*t7.*(-1.907069379620846e-7);
et50 = t6.*t8.*t9.*(-1.769880715106441e-6);
et51 = t8.*t9.*t190.*(-6.800564119502148e-6);
et52 = t2.*t5.*t201.*(-9.619703863182361e-7);
et53 = t5.*t6.*t201.*(-3.96815841743287e-6);
et54 = t2.*t4.*t5.*t7.*(-6.674437170347525e-6);
et55 = t4.*t6.*t7.*t9.*(-2.976937004352228e-6);
et56 = t2.*t8.*t9.*t190.*(-2.976937004352228e-6);
et57 = t6.*t8.*t9.*t190.*(-1.22799597575967e-5);
et58 = t3.*t4.*t5.*t34.*t191.*(-7.138318981153782e-22);
et59 = t2.*t3.*t4.*t5.*t34.*t191.*(-2.089880210625419e-22);
et60 = t3.*t4.*t5.*t6.*t34.*t191.*(-8.620822290548326e-22);
t7259 = (t6821.*(et46+et47+et48+et49+et50+et51+et52+et53+et54+et55+et56+et57+et58+et59+et60))./2.0;
t7260 = (t7072.*t7109)./2.0;
t7261 = (t6919.*t7176)./2.0;
t7263 = t5983+t5995+t6692+t6693+t6696+t6697;
t7264 = t5991+t5994+t6691+t6694+t6695+t6698;
t7269 = t280+t346+t353+t362+t392+t420+t466+t528+t6078+t6345+t6518+t6534+t6807+t6818;
t7271 = (t7077.*t7109)./2.0;
t7275 = (t6832.*t7186)./2.0;
t7276 = t6219+t6365+t6639+t6641+t6708+t6734;
t7284 = t6279+t6371+t6661+t6666+t6773+t6790;
t7296 = (t6821.*t7199)./2.0;
t7299 = t6462.*(-t337-t500-t552+t6128+t6578+t6585-t6616+t4528.*(t4148+t5.*(t2421-t4158)).*7.26735e-3+t4838.*t6468.*(t29-t30).*5.520609140571798e-70).*(-1.0./2.0);
et61 = -t207+t233+t465+t551-t6076-t6169+t6523+t6539+t91.*t5684.*(t6218+t5.*(t3136-t5691)).*5.520609140571798e-70;
et62 = t5684.*t6470.*(t29-t30).*5.520609140571798e-70;
t7300 = t6463.*(et61+et62).*(-1.0./2.0);
et63 = -t207+t233+t465+t551-t6076-t6169+t6523+t6539+t91.*t5684.*(t6218+t5.*(t3136-t5691)).*5.520609140571798e-70;
et64 = t5684.*t6470.*(t29-t30).*5.520609140571798e-70;
t7301 = (t6463.*(et63+et64))./2.0;
et65 = -t231+t275+t469+t553+t6074+t6175-t6676+t5.*t6536+t5684.*t6468.*(t29-t30).*5.520609140571798e-70;
et66 = t5.*t91.*t5824.*t6216.*(-5.520609140571798e-70);
t7302 = t6462.*(et65+et66).*(-1.0./2.0);
t7303 = (t6821.*t7214)./2.0;
t7304 = t6114+t6118+t6824+t6830+t6875+t6877;
t7305 = t6113+t6116+t6825+t6831+t6876+t6878;
t7313 = t249+t347+t438+t506+t529+t546+t556+t569+t6334+t6343+t6783+t6791+t6803+t6808;
et67 = t236+t314+t410+t468-t529+t531+t6332-t6783+t5784.*(t4148+t5.*(t2421-t4158)).*7.26350610236655e-5+t91.*t5824.*(t6218+t5.*(t3136-t5691)).*1.015171749786156e-71;
et68 = t5.*t7.*t8.*(-3.546806877605634e-13)-t7.*t8.*t9.*2.7046541903611e-13;
et69 = t5824.*t6468.*(t29-t30).*5.517689141340903e-72;
et70 = t5824.*t6470.*(t29-t30).*1.015171749786156e-71;
t7314 = t4.*t4119.*(et67+et68+et69+et70).*(-1.0./2.0);
et71 = t236+t314+t410+t468-t529+t531+t6332-t6783+t5784.*(t4148+t5.*(t2421-t4158)).*7.26350610236655e-5+t91.*t5824.*(t6218+t5.*(t3136-t5691)).*1.015171749786156e-71;
et72 = t5.*t7.*t8.*(-3.546806877605634e-13)-t7.*t8.*t9.*2.7046541903611e-13;
et73 = t5824.*t6468.*(t29-t30).*5.517689141340903e-72;
et74 = t5824.*t6470.*(t29-t30).*1.015171749786156e-71;
t7315 = (t4.*t4119.*(et71+et72+et73+et74))./2.0;
et75 = t236+t314+t410+t468-t529+t531+t6332-t6783+t5784.*(t4148+t5.*(t2421-t4158)).*7.26350610236655e-5+t91.*t5824.*(t6218+t5.*(t3136-t5691)).*1.015171749786156e-71;
et76 = t5.*t7.*t8.*(-3.546806877605634e-13)-t7.*t8.*t9.*2.7046541903611e-13;
et77 = t5824.*t6468.*(t29-t30).*5.517689141340903e-72;
et78 = t5824.*t6470.*(t29-t30).*1.015171749786156e-71;
t7318 = t5622.*(et75+et76+et77+et78).*(-1.0./2.0);
et79 = t236+t314+t410+t468-t529+t531+t6332-t6783+t5784.*(t4148+t5.*(t2421-t4158)).*7.26350610236655e-5+t91.*t5824.*(t6218+t5.*(t3136-t5691)).*1.015171749786156e-71;
et80 = t5.*t7.*t8.*(-3.546806877605634e-13)-t7.*t8.*t9.*2.7046541903611e-13;
et81 = t5824.*t6468.*(t29-t30).*5.517689141340903e-72;
et82 = t5824.*t6470.*(t29-t30).*1.015171749786156e-71;
t7319 = (t5622.*(et79+et80+et81+et82))./2.0;
et83 = t236+t314+t410+t468-t529+t531+t6332-t6783+t5784.*(t4148+t5.*(t2421-t4158)).*7.26350610236655e-5+t91.*t5824.*(t6218+t5.*(t3136-t5691)).*1.015171749786156e-71;
et84 = t5.*t7.*t8.*(-3.546806877605634e-13)-t7.*t8.*t9.*2.7046541903611e-13;
et85 = t5824.*t6468.*(t29-t30).*5.517689141340903e-72;
et86 = t5824.*t6470.*(t29-t30).*1.015171749786156e-71;
t7320 = ((t2421-t4158).*(et83+et84+et85+et86))./2.0;
et87 = t6008+t6123-t6672+(t5684.*t6468.*(t29-t30))./1.316403645856965e+67-(t5.*t91.*t5824.*t6216)./1.316403645856965e+67;
et88 = (t5.*t5824.*t6230.*(t29-t30))./1.316403645856965e+67;
t7323 = t7027.*(et87+et88).*(-1.0./2.0);
t7326 = t7027.*(t6109+t6571+t6574-t6610+t4528.*(t4148+t5.*(t2421-t4158))+(t4838.*t6468.*(t29-t30))./1.316403645856965e+67).*(-1.0./2.0);
t7353 = t7060.*(-t337-t500-t552+t6128+t6578+t6585-t6616+t4528.*(t4148+t5.*(t2421-t4158)).*7.26735e-3+t4838.*t6468.*(t29-t30).*5.520609140571798e-70).*(-1.0./2.0);
t7354 = (t7060.*(-t337-t500-t552+t6128+t6578+t6585-t6616+t4528.*(t4148+t5.*(t2421-t4158)).*7.26735e-3+t4838.*t6468.*(t29-t30).*5.520609140571798e-70))./2.0;
et89 = -t207+t233+t465+t551-t6076-t6169+t6523+t6539+t91.*t5684.*(t6218+t5.*(t3136-t5691)).*5.520609140571798e-70;
et90 = t5684.*t6470.*(t29-t30).*5.520609140571798e-70;
t7355 = t7061.*(et89+et90).*(-1.0./2.0);
et91 = -t231+t275+t469+t553+t6074+t6175-t6676+t5.*t6536+t5684.*t6468.*(t29-t30).*5.520609140571798e-70;
et92 = t5.*t91.*t5824.*t6216.*(-5.520609140571798e-70);
t7356 = t7060.*(et91+et92).*(-1.0./2.0);
et93 = -t231+t275+t469+t553+t6074+t6175-t6676+t5.*t6536+t5684.*t6468.*(t29-t30).*5.520609140571798e-70;
et94 = t5.*t91.*t5824.*t6216.*(-5.520609140571798e-70);
t7357 = (t7060.*(et93+et94))./2.0;
t7362 = t5901+t6055+t6062+t6472+t6481+t6723+t6735+t6755+t6764;
t7387 = (t7053.*t7306)./2.0;
et95 = t236+t314+t410+t468-t529+t531+t6332-t6783+t5784.*(t4148+t5.*(t2421-t4158)).*7.26350610236655e-5+t91.*t5824.*(t6218+t5.*(t3136-t5691)).*1.015171749786156e-71;
et96 = t5.*t7.*t8.*(-3.546806877605634e-13)-t7.*t8.*t9.*2.7046541903611e-13;
et97 = t5824.*t6468.*(t29-t30).*5.517689141340903e-72;
et98 = t5824.*t6470.*(t29-t30).*1.015171749786156e-71;
t7397 = t7053.*(et95+et96+et97+et98).*(-1.0./2.0);
t7400 = (t7072.*t7306)./2.0;
t7405 = (t7077.*t7306)./2.0;
t7408 = t320+t328+t380+t414+t505+t5911+t5931+t6086+t6134+t6375+t6387+t6423+t6428+t6589+t6592+t6624+t6635;
t7411 = t325+t333+t386+t416+t526+t5914+t5933+t6083+t6135+t6379+t6390+t6425+t6430+t6584+t6590+t6630+t6637;
et99 = t236+t314+t410+t468-t529+t531+t6332-t6783+t5784.*(t4148+t5.*(t2421-t4158)).*7.26350610236655e-5+t91.*t5824.*(t6218+t5.*(t3136-t5691)).*1.015171749786156e-71;
et100 = t5.*t7.*t8.*(-3.546806877605634e-13)-t7.*t8.*t9.*2.7046541903611e-13;
et101 = t5824.*t6468.*(t29-t30).*5.517689141340903e-72;
et102 = t5824.*t6470.*(t29-t30).*1.015171749786156e-71;
t7414 = t7077.*(et99+et100+et101+et102).*(-1.0./2.0);
et103 = t236+t314+t410+t468-t529+t531+t6332-t6783+t5784.*(t4148+t5.*(t2421-t4158)).*7.26350610236655e-5+t91.*t5824.*(t6218+t5.*(t3136-t5691)).*1.015171749786156e-71;
et104 = t5.*t7.*t8.*(-3.546806877605634e-13)-t7.*t8.*t9.*2.7046541903611e-13;
et105 = t5824.*t6468.*(t29-t30).*5.517689141340903e-72;
et106 = t5824.*t6470.*(t29-t30).*1.015171749786156e-71;
t7415 = (t7077.*(et103+et104+et105+et106))./2.0;
t7421 = t306+t340+t350+t384+t412+t511+t5945+t6075+t6094+t6200+t6447+t6452+t6514+t6530+t6543+t6550+t6680+t6686;
t7424 = t304+t311+t387+t417+t463+t557+t5948+t6079+t6093+t6194+t6450+t6455+t6513+t6529+t6545+t6552+t6682+t6687;
t7438 = -t7437;
t7449 = t5989+t6272+t6298+t6398+t6456+t6459+t6504+t6509+t6667+t6670+t6774+t6796;
t7450 = t5993+t6277+t6301+t6394+t6458+t6461+t6505+t6510+t6668+t6671+t6785+t6804;
t7451 = t235+t348+t439+t558+t562+t593+t6073+t6085+t6167+t6187+t6524+t6526+t6540+t6542+t6677+t6678+t6683+t6684;
et107 = -t235+t315+t413+t539+t543+t567+t6081-t6167+t6182+t6521+t6537-t6677+t5704.*t5784+t91.*t5684.*(t6218+t5.*(t3136-t5691)).*1.015171749786156e-71;
et108 = t5684.*t6468.*(t29-t30).*5.517689141340903e-72;
et109 = t5684.*t6470.*(t29-t30).*1.015171749786156e-71;
et110 = t5.*t91.*t5824.*t6216.*(-5.517689141340903e-72);
et111 = t5.*t5824.*t6230.*(t29-t30).*5.517689141340903e-72;
t7454 = t5657.*(et107+et108+et109+et110+et111).*(-1.0./2.0);
et112 = -t235+t315+t413+t539+t543+t567+t6081-t6167+t6182+t6521+t6537-t6677+t5704.*t5784+t91.*t5684.*(t6218+t5.*(t3136-t5691)).*1.015171749786156e-71;
et113 = t5684.*t6468.*(t29-t30).*5.517689141340903e-72;
et114 = t5684.*t6470.*(t29-t30).*1.015171749786156e-71;
et115 = t5.*t91.*t5824.*t6216.*(-5.517689141340903e-72);
et116 = t5.*t5824.*t6230.*(t29-t30).*5.517689141340903e-72;
t7455 = (t5657.*(et112+et113+et114+et115+et116))./2.0;
et117 = t5986-t6272+t6294+t6397-t6504+t6664+t6669-t6774+t91.*t5824.*(t5670+t4.*(t1458-t5665)).*1.015171749786156e-71;
et118 = t5824.*t6103.*(t29-t30).*1.015171749786156e-71;
et119 = t5822.*t6230.*(t29-t30).*1.015171749786156e-71;
et120 = t5822.*t6468.*(t29-t30).*1.065477564130357e-78;
t7458 = t5872.*(et117+et118+et119+et120).*(-1.0./2.0);
t7472 = t6020+t6025+t6028+t6038+t6704+t6706+t6707+t6716+t6737+t6739+t6740+t6748;
et121 = -t235+t315+t413+t539+t543+t567+t6081-t6167+t6182+t6521+t6537-t6677+t5704.*t5784+t91.*t5684.*(t6218+t5.*(t3136-t5691)).*1.015171749786156e-71;
et122 = t5684.*t6468.*(t29-t30).*5.517689141340903e-72;
et123 = t5684.*t6470.*(t29-t30).*1.015171749786156e-71;
et124 = t5.*t91.*t5824.*t6216.*(-5.517689141340903e-72);
et125 = t5.*t5824.*t6230.*(t29-t30).*5.517689141340903e-72;
t7478 = t6821.*(et121+et122+et123+et124+et125).*(-1.0./2.0);
t7481 = (t6136.*(t5983.*1.33637579258949e-4+t6025+t6028+t6693.*1.33637579258949e-4+t6697.*1.33637579258949e-4+t6704+t6716+t6737+t6748+t5086.*(t4148+t5.*(t2421-t4158))+t57.*t5861.*t6468-t4.*t6465.*(t3136-t5691).*7.26350610236655e-5))./2.0;
et126 = -t5905+t6048+t6053-t6056+t6060-t6487+t6724+t6727-t6738+t6756+t6758+t6230.*(t5878+t9.*(t7.*(t3719-t3788)+(t3.*t34.*t191.*(t29-t30))./8.112963841460668e+31)).*4.126305279697715e-13-t150.*t5861.*t6468+t4.*t6216.*(t3136-t5691).*8.40184101230148e-6;
et127 = t4.*t6465.*(t3136-t5691).*4.126305279697715e-13;
t7517 = t318.*(et126+et127).*(-1.0./2.0);
et128 = -t5905+t6048+t6053-t6056+t6060-t6487+t6724+t6727-t6738+t6756+t6758+t6230.*(t5878+t9.*(t7.*(t3719-t3788)+(t3.*t34.*t191.*(t29-t30))./8.112963841460668e+31)).*4.126305279697715e-13-t150.*t5861.*t6468+t4.*t6216.*(t3136-t5691).*8.40184101230148e-6;
et129 = t4.*t6465.*(t3136-t5691).*4.126305279697715e-13;
t7518 = (t318.*(et128+et129))./2.0;
et130 = t6005-t6486+(t5824.*t6230.*(t29-t30))./1.316403645856965e+67;
et131 = (t5983.*1.33637579258949e-4+t6025+t6028+t6693.*1.33637579258949e-4+t6697.*1.33637579258949e-4+t6704+t6716+t6737+t6748+t5086.*(t4148+t5.*(t2421-t4158))+t57.*t5861.*t6468-t4.*t6465.*(t3136-t5691).*7.26350610236655e-5).*(-1.0./2.0);
t7519 = et130.*et131;
et132 = t6005-t6486+(t5824.*t6230.*(t29-t30))./1.316403645856965e+67;
et133 = (t5983.*1.33637579258949e-4+t6025+t6028+t6693.*1.33637579258949e-4+t6697.*1.33637579258949e-4+t6704+t6716+t6737+t6748+t5086.*(t4148+t5.*(t2421-t4158))+t57.*t5861.*t6468-t4.*t6465.*(t3136-t5691).*7.26350610236655e-5)./2.0;
t7520 = et132.*et133;
et134 = -t5905+t6048+t6053-t6056+t6060-t6487+t6724+t6727-t6738+t6756+t6758+t6230.*(t5878+t9.*(t7.*(t3719-t3788)+(t3.*t34.*t191.*(t29-t30))./8.112963841460668e+31)).*4.126305279697715e-13-t150.*t5861.*t6468+t4.*t6216.*(t3136-t5691).*8.40184101230148e-6;
et135 = t4.*t6465.*(t3136-t5691).*4.126305279697715e-13;
t7523 = t5657.*(et134+et135).*(-1.0./2.0);
et136 = -t5905+t6048+t6053-t6056+t6060-t6487+t6724+t6727-t6738+t6756+t6758+t6230.*(t5878+t9.*(t7.*(t3719-t3788)+(t3.*t34.*t191.*(t29-t30))./8.112963841460668e+31)).*4.126305279697715e-13-t150.*t5861.*t6468+t4.*t6216.*(t3136-t5691).*8.40184101230148e-6;
et137 = t4.*t6465.*(t3136-t5691).*4.126305279697715e-13;
t7524 = (t5657.*(et136+et137))./2.0;
et138 = -t5905+t6048+t6053-t6056+t6060-t6487+t6724+t6727-t6738+t6756+t6758+t6230.*(t5878+t9.*(t7.*(t3719-t3788)+(t3.*t34.*t191.*(t29-t30))./8.112963841460668e+31)).*4.126305279697715e-13-t150.*t5861.*t6468+t4.*t6216.*(t3136-t5691).*8.40184101230148e-6;
et139 = t4.*t6465.*(t3136-t5691).*4.126305279697715e-13;
t7531 = t6821.*(et138+et139).*(-1.0./2.0);
t6318 = -t6314;
t6916 = -t6911;
t6917 = -t6914;
t6923 = -t6921;
t6925 = -t6924;
t6947 = -t6944;
t6956 = -t6952;
t6957 = -t6954;
t6965 = -t6962;
t7004 = -t7002;
t7059 = -t7058;
t7074 = -t7073;
t7099 = (t5925.*t7075)./2.0;
t7102 = (t5939.*t7075)./2.0;
t7123 = t234+t273+t464+t497+t576+t6342+t6788+t6806;
t7126 = (t6436.*t7075)./2.0;
t7127 = (t9.*t7124)./2.0;
t7131 = (t6469.*t7075)./2.0;
t7133 = t6266+t6967+t6999;
t7134 = t6255+t6970+t7003;
t7135 = (t3443.*t7129)./2.0;
t7137 = (t3514.*t7130)./2.0;
t7144 = t7124.*(t4148+t5.*(t2421-t4158)).*(-1.0./2.0);
t7145 = (t7124.*(t4148+t5.*(t2421-t4158)))./2.0;
t7150 = (t6689.*t7075)./2.0;
t7155 = -t7154;
t7156 = (t6350.*t7122)./2.0;
t7160 = (t6351.*t7122)./2.0;
t7164 = t6463.*(t464+t497+t576+t6342+t6788+t6806).*(-1.0./2.0);
t7166 = (t6462.*t7122)./2.0;
t7180 = -t7179;
t7187 = (t6827.*t7122)./2.0;
t7192 = t5676+t6199+t6226+t6252+t6931+t6938;
t7196 = (t6934.*t7122)./2.0;
t7200 = (t3444.*t7191)./2.0;
t7208 = t4.*t9.*(t5709-t6255+t6282+t6296-t7003+t6216.*(t6218+t5.*(t3136-t5691)).*1.40259855e-11).*(-3.0./1.0e+3);
t7210 = (t7019.*t7122)./2.0;
t7218 = -t7217;
t7221 = t9.*t7219.*7.01299275e-12;
t7231 = (t7042.*t7129)./2.0;
t7233 = (t7043.*t7129)./2.0;
t7235 = (t7045.*t7130)./2.0;
t7237 = (t7046.*t7130)./2.0;
t7239 = t7061.*(t464+t497+t576+t6342+t6788+t6806).*(-1.0./2.0);
t7241 = (t7061.*(t464+t497+t576+t6342+t6788+t6806))./2.0;
t7243 = t6349.*(t5709-t6255+t6282+t6296-t7003+t6216.*(t6218+t5.*(t3136-t5691)).*1.40259855e-11).*(-1.0./2.0);
t7247 = t6352.*(t5709-t6255+t6282+t6296-t7003+t6216.*(t6218+t5.*(t3136-t5691)).*1.40259855e-11).*(-1.0./2.0);
t7249 = (t7060.*t7122)./2.0;
t7255 = t6391.*(t5709-t6255+t6282+t6296-t7003+t6216.*(t6218+t5.*(t3136-t5691)).*1.40259855e-11).*(-1.0./2.0);
t7262 = -t7261;
t7265 = (t7067.*t7129)./2.0;
t7266 = (t7069.*t7130)./2.0;
t7267 = t297+t316+t324+t344+t352+t388+t415+t471+t6067+t6348+t6519+t6535+t6798+t6815;
t7270 = (t5.*t7269)./2.0;
t7272 = (t1460.*t7263)./2.0;
t7274 = t6214+t6364+t6638+t6640+t6703+t6725;
t7280 = t5.*t5657.*t7269.*(-1.0./2.0);
t7281 = t6273+t6374+t6658+t6662+t6767+t6777;
t7285 = (t5775.*t7269)./2.0;
t7289 = (t5839.*t7269)./2.0;
t7290 = (t7079.*t7129)./2.0;
t7291 = (t7080.*t7130)./2.0;
t7294 = (t5872.*t7269)./2.0;
t7298 = (t6463.*t7227)./2.0;
t7307 = (t1471.*t7304)./2.0;
t7308 = (t1460.*t7305)./2.0;
t7309 = t437+t472+t527+t538+t544+t595+t6339+t6341+t6786+t6793+t6805+t6811;
t7310 = (t3515.*t7304)./2.0;
t7311 = (t3444.*t7305)./2.0;
t7321 = -t7320;
t7322 = (t7026.*t7215)./2.0;
t7324 = (t7026.*t7219)./2.0;
t7327 = t6221+t6240+t6948+t6949+t6979+t6980;
t7331 = t6258+t6264+t6964+t6972+t6996+t7005;
t7337 = (t7129.*t7153)./2.0;
t7339 = (t7130.*t7159)./2.0;
t7341 = (t7129.*t7162)./2.0;
t7342 = (t7130.*t7163)./2.0;
t7343 = (t7082.*t7191)./2.0;
t7347 = t5762+t5965+t6262+t6315+t6326+t6644+t6652+t6966+t6998;
t7351 = (t7061.*t7227)./2.0;
t7358 = (t7129.*t7177)./2.0;
t7360 = (t7130.*t7178)./2.0;
t7363 = t5904+t6049+t6063+t6475+t6485+t6726+t6732+t6757+t6762;
t7365 = t5750+t6232+t6248+t6303+t6322+t6952+t6960+t6983+t6991;
t7366 = t5755+t6231+t6250+t6308+t6323+t6950+t6959+t6981+t6990;
t7367 = (t8.*t9.*(-t5744+t6232+t6248+t6303+t6322+t6952+t6960+t6983+t6991))./2.0;
t7374 = (t435.*(-t5744+t6232+t6248+t6303+t6322+t6952+t6960+t6983+t6991))./2.0;
t7375 = (t461.*(-t5744+t6232+t6248+t6303+t6322+t6952+t6960+t6983+t6991))./2.0;
t7386 = (t7082.*t7263)./2.0;
C_dq = ft_15({dq1,dq2,dq3,dq4,dq5,dq6,t1004,t1016,t1019,t1020,t1031,t1039,t1046,t1050,t1056,t1061,t1069,t1075,t1076,t1077,t1081,t1083,t1088,t1090,t1095,t1099,t1101,t1106,t1108,t112,t1122,t113,t1133,t1144,t1146,t1147,t115,t1150,t1152,t1155,t1156,t1158,t116,t1165,t1170,t1171,t1174,t1177,t1179,t1184,t1185,t1191,t1193,t1194,t1196,t1201,t1203,t1205,t1207,t121,t1211,t1212,t1213,t1215,t1221,t1224,t1225,t1227,t1228,t1233,t1245,t125,t1250,t1253,t1254,t1258,t1273,t1274,t1282,t1285,t1288,t1292,t1300,t1301,t1306,t131,t1316,t132,t1322,t1323,t1324,t133,t1330,t1331,t1333,t1337,t1342,t1344,t1345,t1348,t1353,t1365,t1377,t1379,t1380,t1383,t1388,t1391,t1402,t1407,t1409,t1411,t1413,t1419,t1423,t1426,t1427,t1428,t1429,t1436,t144,t1440,t1441,t1443,t1445,t1446,t1449,t1454,t1457,t1458,t1460,t1471,t148,t1486,t1487,t1489,t1493,t1494,t1495,t1496,t15,t150,t1503,t1508,t1517,t1520,t1523,t1526,t1530,t1531,t1534,t1537,t1538,t1540,t1541,t1542,t1548,t1550,t1551,t156,t1568,t1570,t1574,t1577,t1578,t158,t1581,t1582,t1584,t1587,t1590,t1592,t1593,t1594,t1598,t16,t1600,t1601,t1602,t1606,t1607,t1609,t1612,t1614,t1615,t1616,t1617,t1619,t1620,t1621,t1622,t1625,t1627,t1630,t1642,t1647,t1648,t1651,t1655,t1656,t1659,t166,t1660,t1661,t1667,t1670,t1672,t1674,t1681,t1687,t1692,t1697,t1699,t17,t1701,t1704,t1705,t1706,t1707,t1708,t171,t1710,t1715,t1716,t1718,t1719,t1721,t1724,t1731,t1732,t1734,t1736,t1740,t1745,t1747,t1748,t1753,t1754,t1756,t1758,t1759,t1761,t1762,t1766,t1767,t1769,t1770,t1771,t1772,t1775,t1776,t1777,t1781,t1783,t1784,t1792,t1793,t1794,t1795,t1797,t1798,t18,t1800,t1805,t1806,t1808,t1811,t1812,t1814,t1815,t1816,t1820,t1821,t1823,t1827,t1828,t1829,t183,t1831,t1833,t1834,t1835,t1836,t1839,t1847,t185,t1855,t1856,t1858,t1860,t1861,t1863,t1868,t1870,t1873,t1878,t1882,t1884,t1886,t1892,t1899,t19,t190,t1900,t1902,t1906,t1908,t1909,t191,t1913,t1916,t1917,t1922,t1925,t1930,t1937,t1938,t1941,t1942,t1947,t1951,t1952,t196,t1967,t1968,t197,t1974,t1977,t1981,t1983,t1984,t1985,t1986,t1989,t199,t1992,t1993,t1995,t1997,t1999,t2,t20,t200,t2002,t2003,t2004,t2006,t2008,t201,t2014,t2015,t2017,t202,t2026,t2027,t2028,t2034,t2035,t2038,t2039,t2043,t2047,t2050,t2052,t2053,t2060,t2062,t2066,t2068,t2069,t2070,t2075,t2076,t2077,t2083,t2085,t2088,t2091,t2096,t2098,t21,t2106,t2110,t2113,t2115,t2118,t2119,t2121,t2123,t2128,t2130,t2132,t2133,t2134,t2136,t2142,t2143,t2145,t2149,t2150,t2154,t2158,t2164,t2165,t2177,t2178,t2180,t2181,t2184,t2186,t2187,t2189,t2191,t2192,t2193,t2196,t2197,t2199,t22,t2200,t2202,t2203,t2211,t2213,t2214,t2217,t2220,t2224,t2234,t2236,t2243,t2253,t2256,t2257,t2266,t2267,t2289,t2291,t2298,t2299,t23,t2300,t2303,t2304,t231,t2312,t2314,t2315,t2320,t2326,t2330,t2333,t2334,t2338,t2341,t2342,t235,t236,t2383,t2390,t2392,t2395,t2396,t2397,t2398,t24,t240,t2416,t2420,t2421,t2424,t2443,t2444,t2449,t2465,t2466,t2474,t2481,t2483,t2486,t2490,t2494,t2497,t2502,t2524,t2525,t2530,t2539,t2544,t2546,t2549,t2552,t2554,t2555,t2556,t2560,t2563,t2564,t2565,t2566,t2567,t2568,t2569,t257,t2571,t2574,t2575,t2576,t2578,t2579,t258,t2588,t2589,t2597,t2598,t2599,t2611,t2612,t2615,t2617,t2627,t263,t2640,t2641,t2655,t2656,t2666,t2684,t2686,t2692,t2694,t2706,t2720,t2722,t2724,t2726,t2737,t2741,t2743,t2748,t2749,t275,t2753,t2755,t2757,t2759,t2761,t2764,t277,t2771,t2778,t278,t2791,t2793,t2795,t2797,t2798,t2799,t2800,t2802,t2806,t2812,t2816,t2818,t2824,t2825,t2827,t2833,t2835,t284,t2851,t2857,t2861,t2868,t287,t2872,t2877,t2880,t2881,t2893,t2895,t2896,t29,t290,t2906,t2911,t2913,t2916,t2918,t2921,t2922,t2932,t2941,t2944,t2956,t2958,t2965,t2973,t2977,t2987,t2999,t3,t30,t300,t302,t3047,t305,t3083,t309,t310,t311,t313,t3136,t314,t3142,t315,t318,t319,t3200,t3209,t3213,t3219,t322,t3222,t3224,t3230,t3239,t3247,t3266,t3268,t3274,t3321,t3338,t336,t3365,t3368,t3369,t337,t3375,t3378,t3380,t3383,t3387,t3390,t3391,t3392,t3397,t34,t3400,t3405,t3407,t3409,t3416,t3417,t3418,t3420,t3422,t3426,t3429,t3430,t3432,t3434,t3435,t3436,t3437,t3439,t3440,t3441,t3443,t3444,t3445,t3446,t3449,t3450,t3453,t3457,t3458,t3462,t3463,t3464,t3465,t3468,t3469,t3471,t3472,t3474,t3475,t3476,t3479,t3480,t3483,t3485,t3489,t349,t3490,t3491,t3492,t3493,t3496,t3498,t3499,t3500,t3501,t3504,t3506,t3507,t3510,t3511,t3513,t3514,t3515,t3517,t3518,t3521,t3522,t3523,t3526,t3530,t3531,t3532,t3535,t3536,t3539,t3540,t3542,t3543,t3547,t3554,t3556,t3557,t356,t3562,t3568,t3569,t357,t3571,t3574,t3577,t3578,t358,t3582,t3583,t3584,t3585,t3592,t3593,t3605,t3606,t3607,t361,t3610,t3611,t3612,t3618,t3634,t3635,t3637,t3642,t3644,t3656,t3658,t3659,t3662,t3666,t3667,t3668,t3673,t3678,t3682,t3694,t3702,t3706,t3708,t371,t3719,t372,t3725,t3726,t373,t3732,t3733,t3734,t3738,t374,t3743,t3746,t3753,t3755,t3757,t3759,t3761,t3763,t3765,t3767,t377,t3772,t378,t3783,t3785,t3788,t379,t3792,t3819,t3821,t3822,t3824,t3831,t3843,t3845,t3851,t3852,t3863,t3869,t3871,t3873,t3874,t3875,t3876,t3882,t3884,t3889,t3890,t3891,t3907,t391,t3910,t3913,t3921,t3922,t3923,t3944,t395,t3951,t3954,t3956,t3957,t3959,t3960,t3968,t3969,t3971,t3972,t3976,t3978,t3979,t3992,t3993,t3995,t3997,t4,t4000,t4004,t401,t4010,t4011,t4014,t4015,t402,t403,t406,t4089,t4099,t410,t4100,t4103,t4108,t411,t4113,t4115,t4118,t4119,t4121,t4123,t4126,t413,t4132,t4134,t4138,t414,t4143,t4146,t4148,t4152,t4153,t4158,t4166,t4173,t4178,t4179,t418,t4181,t4183,t4185,t4190,t4196,t4197,t4206,t4208,t4210,t4217,t422,t4221,t4223,t4226,t4228,t423,t4230,t4232,t4234,t424,t4243,t4249,t425,t4251,t4254,t4255,t4259,t4261,t4263,t427,t4274,t4276,t4278,t4279,t428,t4285,t4286,t429,t4293,t4298,t4301,t4304,t4306,t431,t4317,t4318,t432,t4327,t4329,t433,t4332,t4335,t4337,t4339,t434,t4342,t4344,t4345,t4347,t4348,t4349,t435,t4350,t436,t4369,t4370,t4378,t4380,t4382,t4385,t4388,t4392,t4394,t4395,t4396,t4397,t440,t4402,t4403,t4405,t4406,t4407,t441,t4410,t4412,t4413,t4414,t4416,t4417,t4418,t4419,t442,t4420,t4423,t4425,t4426,t4428,t4429,t4431,t4436,t4437,t444,t4440,t4444,t4446,t4447,t4449,t445,t4450,t4453,t4462,t4467,t4468,t4469,t4471,t4473,t4475,t4478,t4479,t448,t4482,t4483,t4485,t4486,t4487,t4488,t4489,t449,t4490,t4494,t4495,t4498,t4499,t450,t4500,t4501,t4502,t4505,t4506,t4509,t4510,t4515,t4518,t4519,t452,t4520,t4521,t4522,t4523,t4526,t4527,t4528,t453,t4530,t4534,t4536,t4538,t454,t4541,t4543,t4545,t4546,t4549,t4551,t4552,t4553,t4556,t4557,t4558,t4559,t4565,t4568,t457,t4570,t4572,t4575,t4577,t4578,t458,t4581,t4582,t4586,t4587,t4588,t4589,t459,t4590,t4591,t4592,t4593,t4595,t4596,t4598,t460,t4600,t4601,t4602,t4604,t4605,t4606,t4607,t4608,t4614,t4616,t4619,t4621,t4622,t4623,t4624,t4625,t4626,t4629,t463,t4633,t4634,t4636,t4644,t4645,t4647,t4648,t4654,t4656,t4659,t4660,t4666,t4667,t4669,t4673,t4674,t4675,t4678,t468,t4682,t469,t4694,t4695,t4696,t4697,t470,t4707,t4708,t472,t4724,t4727,t4728,t4731,t4732,t4733,t4737,t4738,t4739,t4742,t4743,t4745,t4747,t4748,t475,t4755,t4756,t4762,t477,t4773,t4775,t4780,t4781,t4782,t4783,t4785,t4786,t479,t480,t481,t4810,t482,t4824,t483,t4838,t4842,t485,t486,t4864,t4866,t4869,t4870,t488,t4884,t489,t4903,t4904,t491,t4911,t4914,t4919,t492,t493,t4934,t4936,t494,t4950,t4953,t4957,t496,t4973,t498,t4981,t4983,t4984,t4987,t4990,t4993,t4994,t4995,t4996,t5,t50,t500,t5000,t5002,t5007,t5008,t5009,t5021,t5022,t5023,t5026,t5027,t5032,t5039,t5058,t5061,t5063,t5065,t5075,t5076,t508,t5080,t5084,t509,t5097,t5099,t510,t5102,t5107,t5112,t5114,t512,t5121,t5123,t513,t5132,t5136,t514,t5147,t5150,t5151,t516,t5164,t5166,t517,t518,t5184,t5195,t520,t5203,t5204,t5206,t521,t5210,t5215,t5217,t5219,t522,t5227,t5228,t523,t5232,t5233,t5236,t5238,t524,t5242,t5244,t5249,t525,t5251,t5255,t5258,t5259,t5262,t5269,t527,t5275,t5279,t5280,t5285,t529,t5297,t53,t531,t5316,t5318,t532,t5320,t5323,t5324,t533,t5333,t5339,t534,t5344,t535,t5354,t536,t5370,t539,t540,t543,t5443,t545,t5450,t5457,t5459,t5464,t5465,t5466,t547,t548,t5480,t5482,t5483,t5484,t5486,t5487,t5488,t549,t5507,t552,t5521,t553,t559,t560,t5602,t5605,t561,t5621,t5622,t563,t5633,t5634,t5636,t564,t5647,t5648,t5657,t5658,t5662,t5665,t5666,t567,t5670,t5676,t5679,t568,t5683,t5684,t5688,t5691,t5699,t5700,t5702,t5704,t5706,t5708,t5709,t5710,t5717,t5718,t572,t5729,t5730,t5735,t5738,t5739,t5740,t5742,t5744,t5756,t5757,t5766,t5767,t5769,t5770,t5772,t5774,t5775,t5776,t5778,t578,t5784,t5786,t5787,t5790,t5791,t5792,t5794,t5795,t5797,t580,t5808,t581,t5810,t582,t5822,t5823,t5824,t5825,t5826,t5831,t5838,t5839,t584,t5840,t5841,t5842,t5844,t5845,t5846,t5847,t5848,t5849,t5850,t5851,t5852,t586,t5861,t587,t5872,t5878,t5881,t5882,t5883,t5888,t5889,t589,t5892,t5894,t5895,t5897,t5898,t5899,t590,t5900,t5905,t5907,t5909,t591,t5915,t5916,t5917,t5918,t5919,t592,t5921,t5922,t5923,t5924,t5925,t5926,t5928,t5930,t5934,t5935,t5936,t5937,t5938,t5939,t594,t5940,t5941,t5942,t5943,t5944,t5947,t5949,t5950,t5951,t5952,t5953,t5954,t5956,t5958,t5959,t596,t5960,t5961,t5964,t5966,t5967,t5968,t597,t5970,t5971,t5972,t5973,t5974,t5975,t5976,t5977,t5978,t5979,t5980,t5981,t5982,t5984,t5985,t5986,t5988,t5996,t5998,t5999,t6,t600,t6001,t6002,t6003,t6004,t6005,t6007,t6008,t6009,t6011,t6012,t6013,t6014,t6017,t6019,t602,t6024,t6026,t6029,t603,t6030,t6032,t6035,t6037,t604,t6040,t6041,t6042,t6043,t6044,t6045,t6046,t6047,t6048,t605,t6051,t6052,t6053,t6056,t6057,t6060,t6064,t6065,t6069,t6074,t6081,t609,t6095,t610,t6103,t6108,t6109,t611,t6118,t6119,t612,t6121,t6123,t6125,t6127,t6128,t613,t6130,t6131,t6136,t6137,t6138,t614,t6141,t6142,t6143,t6144,t6145,t6146,t6147,t615,t6150,t6151,t6152,t6154,t6155,t6157,t6158,t6159,t616,t6160,t6161,t6162,t6164,t6165,t6167,t6170,t6171,t6172,t6173,t6175,t6176,t6177,t6179,t618,t6182,t6183,t6185,t6186,t6188,t6189,t619,t6190,t6191,t6194,t6195,t6196,t6197,t620,t6201,t6202,t6203,t6204,t6205,t6206,t6207,t6208,t6209,t621,t6210,t6211,t6212,t6213,t6215,t6216,t6218,t622,t6220,t6222,t6225,t6226,t6228,t6229,t623,t6230,t6231,t6232,t6235,t6239,t624,t6241,t6242,t6243,t6244,t6245,t6248,t6249,t625,t6251,t6252,t6255,t6256,t6260,t6267,t6268,t6270,t6271,t6272,t6274,t6275,t6276,t6278,t6280,t6281,t6282,t6283,t6284,t6285,t6288,t6289,t6290,t6292,t6293,t6294,t6295,t6296,t6297,t6299,t6300,t6303,t6306,t6307,t6309,t6311,t6312,t6313,t6316,t6317,t6318,t632,t6322,t6324,t6327,t6328,t6329,t6330,t6331,t6332,t6345,t6349,t6350,t6351,t6352,t6359,t6360,t6361,t6362,t6370,t6378,t638,t6380,t6382,t6385,t6386,t6391,t6393,t6395,t6396,t6397,t6399,t640,t6400,t6401,t6402,t6404,t6405,t6406,t6407,t6408,t6412,t6414,t6422,t6426,t6427,t6431,t6432,t6433,t6434,t6435,t6442,t6443,t6444,t6445,t6446,t6449,t6451,t6454,t6462,t6463,t6465,t6468,t6470,t6471,t6473,t6476,t6477,t6482,t6486,t6487,t6488,t6489,t6492,t6498,t6501,t6503,t6504,t6507,t6513,t6521,t6536,t6537,t6544,t6546,t6547,t6548,t6549,t6551,t6555,t6556,t6557,t6560,t6561,t6562,t6563,t6564,t6566,t6567,t6569,t6571,t6574,t6576,t6578,t6579,t6580,t6582,t6585,t6586,t6593,t6594,t6595,t6599,t6600,t6601,t6602,t6603,t6604,t6605,t6606,t6607,t6608,t6610,t6616,t6620,t6621,t6631,t6632,t6642,t6646,t6648,t6649,t6650,t6654,t6656,t6657,t6659,t6660,t6663,t6664,t6665,t6669,t6672,t6676,t6677,t6694,t6695,t6699,t6709,t6710,t6711,t6712,t6713,t6714,t6715,t6717,t6718,t6719,t6720,t6721,t6724,t6727,t6728,t6729,t6730,t6733,t6738,t6741,t6742,t6743,t6744,t6745,t6746,t6747,t6749,t6750,t6751,t6752,t6753,t6756,t6758,t6759,t6761,t6763,t6765,t6771,t6772,t6774,t6776,t6783,t6787,t6789,t6807,t681,t6818,t6821,t6826,t6831,t6832,t6837,t6838,t6839,t684,t6840,t6841,t6842,t6844,t6845,t6847,t6848,t6849,t6850,t6851,t6855,t6856,t6857,t6858,t6859,t6860,t6862,t6863,t6865,t6866,t6867,t6868,t6869,t6870,t6871,t6872,t6873,t6879,t6880,t6881,t6882,t6883,t6884,t6885,t6888,t6889,t6890,t6891,t6892,t6893,t6894,t6896,t6897,t6898,t6900,t6901,t6902,t6903,t6904,t6906,t6907,t6908,t6909,t6910,t6911,t6913,t6914,t6915,t6916,t6917,t6918,t6919,t6920,t6921,t6922,t6923,t6924,t6925,t6926,t6927,t6928,t6930,t6933,t6935,t6936,t6937,t6939,t6941,t6942,t6943,t6944,t6945,t6946,t6947,t6951,t6952,t6953,t6954,t6955,t6956,t6957,t6958,t6959,t6960,t6961,t6963,t6965,t6968,t6971,t6973,t6974,t6975,t6976,t6977,t6978,t6982,t6983,t6984,t6985,t6986,t6987,t6988,t6989,t6990,t6991,t6992,t6994,t6995,t6997,t7,t7000,t7001,t7003,t7004,t7006,t7007,t7008,t7009,t7010,t7011,t7012,t7013,t7015,t7016,t7017,t7018,t7020,t7022,t7023,t7024,t7025,t7026,t7027,t7028,t7029,t7030,t7031,t7032,t7033,t7034,t7035,t7036,t7039,t7040,t7041,t7042,t7044,t7045,t7048,t7051,t7052,t7053,t7054,t7055,t7056,t7057,t7059,t7060,t7061,t7064,t7066,t7067,t7068,t7069,t7070,t7071,t7072,t7073,t7074,t7075,t7076,t7077,t7078,t7081,t7082,t7083,t7084,t7085,t7086,t7087,t7088,t7089,t7090,t7091,t7092,t7093,t7094,t7095,t7096,t7097,t7098,t7099,t7100,t7101,t7102,t7103,t7104,t7108,t7110,t7111,t7113,t7114,t7115,t7116,t712,t7120,t7121,t7122,t7123,t7124,t7126,t7127,t7128,t7129,t7130,t7131,t7133,t7134,t7135,t7137,t7139,t7140,t7141,t7142,t7143,t7144,t7145,t7146,t7147,t7148,t7149,t7150,t7155,t7156,t7160,t7164,t7165,t7166,t7168,t7169,t7170,t7171,t7173,t7174,t7175,t7176,t7179,t7180,t7182,t7183,t7185,t7187,t7191,t7192,t7193,t7194,t7195,t7196,t72,t7200,t7208,t7209,t7210,t7215,t7217,t7218,t7219,t7221,t7223,t7224,t7225,t7226,t7231,t7233,t7235,t7237,t7238,t7239,t724,t7240,t7241,t7243,t7244,t7247,t7248,t7249,t7255,t7256,t7257,t7258,t7259,t7260,t7261,t7262,t7263,t7265,t7266,t7267,t7269,t7270,t7271,t7272,t7273,t7274,t7275,t7276,t7280,t7281,t7284,t7285,t7289,t7290,t7291,t7294,t7296,t7297,t7298,t7299,t73,t7300,t7301,t7302,t7303,t7304,t7305,t7307,t7308,t7309,t7310,t7311,t7314,t7315,t7319,t7320,t7321,t7322,t7323,t7324,t7326,t7327,t7331,t7334,t7335,t7337,t7339,t7341,t7342,t7343,t7347,t7351,t7354,t7355,t7357,t7358,t7360,t7362,t7363,t7364,t7366,t7367,t7374,t7375,t738,t7386,t7387,t7388,t739,t7397,t7400,t7405,t7408,t741,t7411,t7414,t7415,t742,t7421,t7437,t7438,t7450,t7454,t7455,t7458,t7467,t7478,t7481,t7517,t7519,t7523,t7524,t7528,t753,t7531,t7544,t7549,t7550,t7551,t7553,t7557,t7558,t7560,t7564,t7565,t7567,t7568,t7569,t7570,t7571,t7573,t7574,t7575,t7576,t7577,t7578,t7579,t7580,t7581,t760,t781,t792,t796,t797,t8,t803,t81,t825,t826,t827,t830,t832,t845,t847,t848,t852,t856,t86,t861,t866,t868,t869,t874,t875,t877,t878,t881,t893,t899,t9,t90,t902,t903,t905,t908,t909,t91,t910,t911,t912,t915,t917,t919,t922,t925,t926,t928,t929,t930,t931,t932,t934,t940,t944,t945,t947,t95,t952,t954,t955,t957,t958,t968,t970,t971,t972,t975,t976,t984,t985,t986,t989,t99,t991,t998});
end
function C_dq = ft_15(ct)
dq1 = ct{1};
dq2 = ct{2};
dq3 = ct{3};
dq4 = ct{4};
dq5 = ct{5};
dq6 = ct{6};
t1004 = ct{7};
t1016 = ct{8};
t1019 = ct{9};
t1020 = ct{10};
t1031 = ct{11};
t1039 = ct{12};
t1046 = ct{13};
t1050 = ct{14};
t1056 = ct{15};
t1061 = ct{16};
t1069 = ct{17};
t1075 = ct{18};
t1076 = ct{19};
t1077 = ct{20};
t1081 = ct{21};
t1083 = ct{22};
t1088 = ct{23};
t1090 = ct{24};
t1095 = ct{25};
t1099 = ct{26};
t1101 = ct{27};
t1106 = ct{28};
t1108 = ct{29};
t112 = ct{30};
t1122 = ct{31};
t113 = ct{32};
t1133 = ct{33};
t1144 = ct{34};
t1146 = ct{35};
t1147 = ct{36};
t115 = ct{37};
t1150 = ct{38};
t1152 = ct{39};
t1155 = ct{40};
t1156 = ct{41};
t1158 = ct{42};
t116 = ct{43};
t1165 = ct{44};
t1170 = ct{45};
t1171 = ct{46};
t1174 = ct{47};
t1177 = ct{48};
t1179 = ct{49};
t1184 = ct{50};
t1185 = ct{51};
t1191 = ct{52};
t1193 = ct{53};
t1194 = ct{54};
t1196 = ct{55};
t1201 = ct{56};
t1203 = ct{57};
t1205 = ct{58};
t1207 = ct{59};
t121 = ct{60};
t1211 = ct{61};
t1212 = ct{62};
t1213 = ct{63};
t1215 = ct{64};
t1221 = ct{65};
t1224 = ct{66};
t1225 = ct{67};
t1227 = ct{68};
t1228 = ct{69};
t1233 = ct{70};
t1245 = ct{71};
t125 = ct{72};
t1250 = ct{73};
t1253 = ct{74};
t1254 = ct{75};
t1258 = ct{76};
t1273 = ct{77};
t1274 = ct{78};
t1282 = ct{79};
t1285 = ct{80};
t1288 = ct{81};
t1292 = ct{82};
t1300 = ct{83};
t1301 = ct{84};
t1306 = ct{85};
t131 = ct{86};
t1316 = ct{87};
t132 = ct{88};
t1322 = ct{89};
t1323 = ct{90};
t1324 = ct{91};
t133 = ct{92};
t1330 = ct{93};
t1331 = ct{94};
t1333 = ct{95};
t1337 = ct{96};
t1342 = ct{97};
t1344 = ct{98};
t1345 = ct{99};
t1348 = ct{100};
t1353 = ct{101};
t1365 = ct{102};
t1377 = ct{103};
t1379 = ct{104};
t1380 = ct{105};
t1383 = ct{106};
t1388 = ct{107};
t1391 = ct{108};
t1402 = ct{109};
t1407 = ct{110};
t1409 = ct{111};
t1411 = ct{112};
t1413 = ct{113};
t1419 = ct{114};
t1423 = ct{115};
t1426 = ct{116};
t1427 = ct{117};
t1428 = ct{118};
t1429 = ct{119};
t1436 = ct{120};
t144 = ct{121};
t1440 = ct{122};
t1441 = ct{123};
t1443 = ct{124};
t1445 = ct{125};
t1446 = ct{126};
t1449 = ct{127};
t1454 = ct{128};
t1457 = ct{129};
t1458 = ct{130};
t1460 = ct{131};
t1471 = ct{132};
t148 = ct{133};
t1486 = ct{134};
t1487 = ct{135};
t1489 = ct{136};
t1493 = ct{137};
t1494 = ct{138};
t1495 = ct{139};
t1496 = ct{140};
t15 = ct{141};
t150 = ct{142};
t1503 = ct{143};
t1508 = ct{144};
t1517 = ct{145};
t1520 = ct{146};
t1523 = ct{147};
t1526 = ct{148};
t1530 = ct{149};
t1531 = ct{150};
t1534 = ct{151};
t1537 = ct{152};
t1538 = ct{153};
t1540 = ct{154};
t1541 = ct{155};
t1542 = ct{156};
t1548 = ct{157};
t1550 = ct{158};
t1551 = ct{159};
t156 = ct{160};
t1568 = ct{161};
t1570 = ct{162};
t1574 = ct{163};
t1577 = ct{164};
t1578 = ct{165};
t158 = ct{166};
t1581 = ct{167};
t1582 = ct{168};
t1584 = ct{169};
t1587 = ct{170};
t1590 = ct{171};
t1592 = ct{172};
t1593 = ct{173};
t1594 = ct{174};
t1598 = ct{175};
t16 = ct{176};
t1600 = ct{177};
t1601 = ct{178};
t1602 = ct{179};
t1606 = ct{180};
t1607 = ct{181};
t1609 = ct{182};
t1612 = ct{183};
t1614 = ct{184};
t1615 = ct{185};
t1616 = ct{186};
t1617 = ct{187};
t1619 = ct{188};
t1620 = ct{189};
t1621 = ct{190};
t1622 = ct{191};
t1625 = ct{192};
t1627 = ct{193};
t1630 = ct{194};
t1642 = ct{195};
t1647 = ct{196};
t1648 = ct{197};
t1651 = ct{198};
t1655 = ct{199};
t1656 = ct{200};
t1659 = ct{201};
t166 = ct{202};
t1660 = ct{203};
t1661 = ct{204};
t1667 = ct{205};
t1670 = ct{206};
t1672 = ct{207};
t1674 = ct{208};
t1681 = ct{209};
t1687 = ct{210};
t1692 = ct{211};
t1697 = ct{212};
t1699 = ct{213};
t17 = ct{214};
t1701 = ct{215};
t1704 = ct{216};
t1705 = ct{217};
t1706 = ct{218};
t1707 = ct{219};
t1708 = ct{220};
t171 = ct{221};
t1710 = ct{222};
t1715 = ct{223};
t1716 = ct{224};
t1718 = ct{225};
t1719 = ct{226};
t1721 = ct{227};
t1724 = ct{228};
t1731 = ct{229};
t1732 = ct{230};
t1734 = ct{231};
t1736 = ct{232};
t1740 = ct{233};
t1745 = ct{234};
t1747 = ct{235};
t1748 = ct{236};
t1753 = ct{237};
t1754 = ct{238};
t1756 = ct{239};
t1758 = ct{240};
t1759 = ct{241};
t1761 = ct{242};
t1762 = ct{243};
t1766 = ct{244};
t1767 = ct{245};
t1769 = ct{246};
t1770 = ct{247};
t1771 = ct{248};
t1772 = ct{249};
t1775 = ct{250};
t1776 = ct{251};
t1777 = ct{252};
t1781 = ct{253};
t1783 = ct{254};
t1784 = ct{255};
t1792 = ct{256};
t1793 = ct{257};
t1794 = ct{258};
t1795 = ct{259};
t1797 = ct{260};
t1798 = ct{261};
t18 = ct{262};
t1800 = ct{263};
t1805 = ct{264};
t1806 = ct{265};
t1808 = ct{266};
t1811 = ct{267};
t1812 = ct{268};
t1814 = ct{269};
t1815 = ct{270};
t1816 = ct{271};
t1820 = ct{272};
t1821 = ct{273};
t1823 = ct{274};
t1827 = ct{275};
t1828 = ct{276};
t1829 = ct{277};
t183 = ct{278};
t1831 = ct{279};
t1833 = ct{280};
t1834 = ct{281};
t1835 = ct{282};
t1836 = ct{283};
t1839 = ct{284};
t1847 = ct{285};
t185 = ct{286};
t1855 = ct{287};
t1856 = ct{288};
t1858 = ct{289};
t1860 = ct{290};
t1861 = ct{291};
t1863 = ct{292};
t1868 = ct{293};
t1870 = ct{294};
t1873 = ct{295};
t1878 = ct{296};
t1882 = ct{297};
t1884 = ct{298};
t1886 = ct{299};
t1892 = ct{300};
t1899 = ct{301};
t19 = ct{302};
t190 = ct{303};
t1900 = ct{304};
t1902 = ct{305};
t1906 = ct{306};
t1908 = ct{307};
t1909 = ct{308};
t191 = ct{309};
t1913 = ct{310};
t1916 = ct{311};
t1917 = ct{312};
t1922 = ct{313};
t1925 = ct{314};
t1930 = ct{315};
t1937 = ct{316};
t1938 = ct{317};
t1941 = ct{318};
t1942 = ct{319};
t1947 = ct{320};
t1951 = ct{321};
t1952 = ct{322};
t196 = ct{323};
t1967 = ct{324};
t1968 = ct{325};
t197 = ct{326};
t1974 = ct{327};
t1977 = ct{328};
t1981 = ct{329};
t1983 = ct{330};
t1984 = ct{331};
t1985 = ct{332};
t1986 = ct{333};
t1989 = ct{334};
t199 = ct{335};
t1992 = ct{336};
t1993 = ct{337};
t1995 = ct{338};
t1997 = ct{339};
t1999 = ct{340};
t2 = ct{341};
t20 = ct{342};
t200 = ct{343};
t2002 = ct{344};
t2003 = ct{345};
t2004 = ct{346};
t2006 = ct{347};
t2008 = ct{348};
t201 = ct{349};
t2014 = ct{350};
t2015 = ct{351};
t2017 = ct{352};
t202 = ct{353};
t2026 = ct{354};
t2027 = ct{355};
t2028 = ct{356};
t2034 = ct{357};
t2035 = ct{358};
t2038 = ct{359};
t2039 = ct{360};
t2043 = ct{361};
t2047 = ct{362};
t2050 = ct{363};
t2052 = ct{364};
t2053 = ct{365};
t2060 = ct{366};
t2062 = ct{367};
t2066 = ct{368};
t2068 = ct{369};
t2069 = ct{370};
t2070 = ct{371};
t2075 = ct{372};
t2076 = ct{373};
t2077 = ct{374};
t2083 = ct{375};
t2085 = ct{376};
t2088 = ct{377};
t2091 = ct{378};
t2096 = ct{379};
t2098 = ct{380};
t21 = ct{381};
t2106 = ct{382};
t2110 = ct{383};
t2113 = ct{384};
t2115 = ct{385};
t2118 = ct{386};
t2119 = ct{387};
t2121 = ct{388};
t2123 = ct{389};
t2128 = ct{390};
t2130 = ct{391};
t2132 = ct{392};
t2133 = ct{393};
t2134 = ct{394};
t2136 = ct{395};
t2142 = ct{396};
t2143 = ct{397};
t2145 = ct{398};
t2149 = ct{399};
t2150 = ct{400};
t2154 = ct{401};
t2158 = ct{402};
t2164 = ct{403};
t2165 = ct{404};
t2177 = ct{405};
t2178 = ct{406};
t2180 = ct{407};
t2181 = ct{408};
t2184 = ct{409};
t2186 = ct{410};
t2187 = ct{411};
t2189 = ct{412};
t2191 = ct{413};
t2192 = ct{414};
t2193 = ct{415};
t2196 = ct{416};
t2197 = ct{417};
t2199 = ct{418};
t22 = ct{419};
t2200 = ct{420};
t2202 = ct{421};
t2203 = ct{422};
t2211 = ct{423};
t2213 = ct{424};
t2214 = ct{425};
t2217 = ct{426};
t2220 = ct{427};
t2224 = ct{428};
t2234 = ct{429};
t2236 = ct{430};
t2243 = ct{431};
t2253 = ct{432};
t2256 = ct{433};
t2257 = ct{434};
t2266 = ct{435};
t2267 = ct{436};
t2289 = ct{437};
t2291 = ct{438};
t2298 = ct{439};
t2299 = ct{440};
t23 = ct{441};
t2300 = ct{442};
t2303 = ct{443};
t2304 = ct{444};
t231 = ct{445};
t2312 = ct{446};
t2314 = ct{447};
t2315 = ct{448};
t2320 = ct{449};
t2326 = ct{450};
t2330 = ct{451};
t2333 = ct{452};
t2334 = ct{453};
t2338 = ct{454};
t2341 = ct{455};
t2342 = ct{456};
t235 = ct{457};
t236 = ct{458};
t2383 = ct{459};
t2390 = ct{460};
t2392 = ct{461};
t2395 = ct{462};
t2396 = ct{463};
t2397 = ct{464};
t2398 = ct{465};
t24 = ct{466};
t240 = ct{467};
t2416 = ct{468};
t2420 = ct{469};
t2421 = ct{470};
t2424 = ct{471};
t2443 = ct{472};
t2444 = ct{473};
t2449 = ct{474};
t2465 = ct{475};
t2466 = ct{476};
t2474 = ct{477};
t2481 = ct{478};
t2483 = ct{479};
t2486 = ct{480};
t2490 = ct{481};
t2494 = ct{482};
t2497 = ct{483};
t2502 = ct{484};
t2524 = ct{485};
t2525 = ct{486};
t2530 = ct{487};
t2539 = ct{488};
t2544 = ct{489};
t2546 = ct{490};
t2549 = ct{491};
t2552 = ct{492};
t2554 = ct{493};
t2555 = ct{494};
t2556 = ct{495};
t2560 = ct{496};
t2563 = ct{497};
t2564 = ct{498};
t2565 = ct{499};
t2566 = ct{500};
t2567 = ct{501};
t2568 = ct{502};
t2569 = ct{503};
t257 = ct{504};
t2571 = ct{505};
t2574 = ct{506};
t2575 = ct{507};
t2576 = ct{508};
t2578 = ct{509};
t2579 = ct{510};
t258 = ct{511};
t2588 = ct{512};
t2589 = ct{513};
t2597 = ct{514};
t2598 = ct{515};
t2599 = ct{516};
t2611 = ct{517};
t2612 = ct{518};
t2615 = ct{519};
t2617 = ct{520};
t2627 = ct{521};
t263 = ct{522};
t2640 = ct{523};
t2641 = ct{524};
t2655 = ct{525};
t2656 = ct{526};
t2666 = ct{527};
t2684 = ct{528};
t2686 = ct{529};
t2692 = ct{530};
t2694 = ct{531};
t2706 = ct{532};
t2720 = ct{533};
t2722 = ct{534};
t2724 = ct{535};
t2726 = ct{536};
t2737 = ct{537};
t2741 = ct{538};
t2743 = ct{539};
t2748 = ct{540};
t2749 = ct{541};
t275 = ct{542};
t2753 = ct{543};
t2755 = ct{544};
t2757 = ct{545};
t2759 = ct{546};
t2761 = ct{547};
t2764 = ct{548};
t277 = ct{549};
t2771 = ct{550};
t2778 = ct{551};
t278 = ct{552};
t2791 = ct{553};
t2793 = ct{554};
t2795 = ct{555};
t2797 = ct{556};
t2798 = ct{557};
t2799 = ct{558};
t2800 = ct{559};
t2802 = ct{560};
t2806 = ct{561};
t2812 = ct{562};
t2816 = ct{563};
t2818 = ct{564};
t2824 = ct{565};
t2825 = ct{566};
t2827 = ct{567};
t2833 = ct{568};
t2835 = ct{569};
t284 = ct{570};
t2851 = ct{571};
t2857 = ct{572};
t2861 = ct{573};
t2868 = ct{574};
t287 = ct{575};
t2872 = ct{576};
t2877 = ct{577};
t2880 = ct{578};
t2881 = ct{579};
t2893 = ct{580};
t2895 = ct{581};
t2896 = ct{582};
t29 = ct{583};
t290 = ct{584};
t2906 = ct{585};
t2911 = ct{586};
t2913 = ct{587};
t2916 = ct{588};
t2918 = ct{589};
t2921 = ct{590};
t2922 = ct{591};
t2932 = ct{592};
t2941 = ct{593};
t2944 = ct{594};
t2956 = ct{595};
t2958 = ct{596};
t2965 = ct{597};
t2973 = ct{598};
t2977 = ct{599};
t2987 = ct{600};
t2999 = ct{601};
t3 = ct{602};
t30 = ct{603};
t300 = ct{604};
t302 = ct{605};
t3047 = ct{606};
t305 = ct{607};
t3083 = ct{608};
t309 = ct{609};
t310 = ct{610};
t311 = ct{611};
t313 = ct{612};
t3136 = ct{613};
t314 = ct{614};
t3142 = ct{615};
t315 = ct{616};
t318 = ct{617};
t319 = ct{618};
t3200 = ct{619};
t3209 = ct{620};
t3213 = ct{621};
t3219 = ct{622};
t322 = ct{623};
t3222 = ct{624};
t3224 = ct{625};
t3230 = ct{626};
t3239 = ct{627};
t3247 = ct{628};
t3266 = ct{629};
t3268 = ct{630};
t3274 = ct{631};
t3321 = ct{632};
t3338 = ct{633};
t336 = ct{634};
t3365 = ct{635};
t3368 = ct{636};
t3369 = ct{637};
t337 = ct{638};
t3375 = ct{639};
t3378 = ct{640};
t3380 = ct{641};
t3383 = ct{642};
t3387 = ct{643};
t3390 = ct{644};
t3391 = ct{645};
t3392 = ct{646};
t3397 = ct{647};
t34 = ct{648};
t3400 = ct{649};
t3405 = ct{650};
t3407 = ct{651};
t3409 = ct{652};
t3416 = ct{653};
t3417 = ct{654};
t3418 = ct{655};
t3420 = ct{656};
t3422 = ct{657};
t3426 = ct{658};
t3429 = ct{659};
t3430 = ct{660};
t3432 = ct{661};
t3434 = ct{662};
t3435 = ct{663};
t3436 = ct{664};
t3437 = ct{665};
t3439 = ct{666};
t3440 = ct{667};
t3441 = ct{668};
t3443 = ct{669};
t3444 = ct{670};
t3445 = ct{671};
t3446 = ct{672};
t3449 = ct{673};
t3450 = ct{674};
t3453 = ct{675};
t3457 = ct{676};
t3458 = ct{677};
t3462 = ct{678};
t3463 = ct{679};
t3464 = ct{680};
t3465 = ct{681};
t3468 = ct{682};
t3469 = ct{683};
t3471 = ct{684};
t3472 = ct{685};
t3474 = ct{686};
t3475 = ct{687};
t3476 = ct{688};
t3479 = ct{689};
t3480 = ct{690};
t3483 = ct{691};
t3485 = ct{692};
t3489 = ct{693};
t349 = ct{694};
t3490 = ct{695};
t3491 = ct{696};
t3492 = ct{697};
